simulink model "simulator_prototype_v2"  (R2021b)
(part 5 of 12)

tau_c = ft_4({t100,t1000,t1001,t1002,t1003,t1006,t1009,t101,t1011,t1014,t1015,t1017,t1018,t1019,t1020,t1021,t1023,t1024,t1025,t1028,t1029,t103,t1030,t1031,t1032,t1035,t1038,t1039,t104,t1041,t1042,t1044,t1045,t1046,t1048,t1049,t1050,t1051,t1052,t1055,t1056,t1057,t1058,t1059,t106,t1061,t1062,t1065,t1066,t1067,t107,t1070,t1071,t1072,t1073,t1074,t1075,t1076,t108,t1080,t1083,t1084,t1089,t109,t1090,t1091,t1092,t1094,t1095,t1098,t1099,t110,t1100,t1102,t1103,t1104,t1105,t1106,t1107,t1108,t1109,t111,t1110,t1111,t1112,t1113,t1114,t1115,t1116,t1117,t1118,t1119,t1120,t1121,t1122,t1123,t1124,t1125,t1126,t1129,t113,t1132,t1135,t1137,t1138,t1139,t114,t1140,t1141,t1142,t1144,t1145,t1146,t1147,t1148,t1149,t115,t1150,t1154,t1158,t1159,t1162,t1165,t1166,t1167,t1170,t1174,t1176,t1177,t1178,t1179,t118,t1180,t1184,t1185,t1186,t1187,t1188,t1189,t1190,t1192,t1193,t1194,t1195,t1196,t1197,t1198,t1199,t120,t1202,t1203,t1204,t1205,t1206,t1207,t1208,t1209,t121,t1210,t1212,t1213,t1214,t1217,t1218,t1219,t122,t1220,t1221,t1222,t1223,t1224,t1229,t123,t1230,t1232,t1234,t1235,t1236,t1237,t1238,t124,t1241,t1242,t1245,t1246,t1247,t1248,t125,t1251,t1252,t1253,t1254,t1255,t1256,t1259,t126,t1260,t1261,t1262,t1263,t1264,t1265,t1266,t1267,t1268,t127,t1270,t1271,t1272,t1277,t1278,t128,t1280,t1281,t1285,t1286,t1287,t1288,t1289,t1290,t1291,t1292,t1294,t1295,t1296,t1297,t1298,t1299,t130,t1300,t1301,t1302,t1303,t1304,t1305,t1307,t1310,t1311,t1316,t1317,t1319,t132,t1320,t1322,t1323,t1324,t1325,t1326,t1328,t133,t1330,t1331,t1332,t1334,t1335,t1336,t1337,t1338,t134,t1342,t1343,t1344,t1345,t1348,t1349,t1350,t1351,t1352,t1353,t1354,t136,t1360,t1364,t1366,t1367,t1368,t1369,t1370,t1371,t1372,t1374,t1375,t1376,t1377,t1378,t1379,t138,t1380,t1383,t1385,t1386,t1387,t1388,t1389,t139,t1392,t1393,t1394,t1395,t1396,t1397,t1398,t1399,t14,t140,t1401,t1402,t1403,t1404,t1405,t1406,t1407,t1408,t1409,t1410,t1411,t1412,t1413,t1414,t1415,t1416,t1417,t1418,t1419,t1420,t1421,t1422,t1423,t1424,t1425,t1426,t1427,t1428,t1429,t1430,t1431,t1432,t1433,t1434,t1435,t1436,t1437,t1439,t144,t1440,t1441,t1443,t1444,t1445,t1446,t1447,t1448,t145,t1451,t1453,t1454,t1456,t1457,t1458,t1459,t1460,t1461,t1462,t1463,t1464,t1468,t1469,t1471,t1474,t1477,t1478,t1479,t148,t1480,t1481,t1482,t1483,t1484,t1485,t1486,t1487,t1488,t1489,t149,t1490,t1491,t1492,t1493,t1494,t1495,t1497,t1498,t1499,t15,t150,t1500,t1501,t1503,t1504,t1505,t1506,t1507,t1509,t151,t1510,t1512,t1513,t1514,t1515,t1516,t1517,t1518,t1519,t152,t1520,t1522,t1523,t1525,t1526,t1527,t1528,t1529,t153,t1530,t1531,t1532,t1533,t1535,t1536,t1537,t1538,t1539,t1541,t1542,t1543,t1544,t1545,t1546,t1547,t1549,t1550,t1551,t1552,t1554,t1555,t1556,t1558,t1559,t156,t1560,t1565,t1567,t1568,t1569,t157,t1570,t1571,t1572,t1574,t1575,t1576,t1577,t1578,t1579,t158,t1581,t1582,t1583,t1584,t1585,t1586,t1587,t1588,t1591,t1592,t1593,t1594,t1595,t1596,t1599,t16,t160,t1600,t1601,t1602,t1604,t1605,t1606,t1607,t1608,t1609,t161,t1613,t1614,t1615,t1616,t1618,t1619,t162,t1620,t1621,t1622,t1623,t1624,t1625,t1626,t1627,t1628,t1629,t1631,t1633,t1634,t1635,t1636,t1637,t1638,t1639,t1640,t1641,t1642,t1643,t1644,t1645,t1646,t1648,t1649,t165,t1650,t1651,t1652,t1653,t1654,t1655,t1656,t1657,t1658,t166,t1660,t167,t168,t1686,t1688,t1689,t1690,t1695,t17,t170,t1700,t1701,t1702,t171,t172,t173,t174,t175,t1750,t176,t1765,t177,t178,t1780,t1782,t1795,t1796,t1797,t1798,t18,t180,t1807,t181,t1817,t182,t185,t186,t1865,t1868,t1870,t1871,t1872,t1873,t1874,t1875,t1876,t1877,t1879,t188,t1880,t1881,t1882,t1883,t1884,t1886,t1887,t1889,t189,t1890,t1891,t1894,t1895,t1897,t1898,t1899,t19,t190,t1901,t1902,t1903,t1904,t1907,t1909,t191,t1914,t1915,t1916,t1917,t1919,t192,t1920,t1922,t1923,t1924,t1925,t1926,t1927,t1928,t1929,t1930,t1931,t1936,t1937,t1940,t1941,t1942,t1943,t1947,t1948,t1949,t195,t1950,t1951,t1952,t1953,t1956,t1958,t1959,t196,t1960,t1961,t1965,t1966,t1967,t1968,t197,t1970,t1971,t1975,t1977,t198,t1982,t1991,t1997,t2,t20,t201,t2017,t202,t2021,t2022,t2024,t2025,t2027,t2028,t2029,t203,t2030,t2032,t2034,t2035,t2038,t2039,t204,t2043,t2044,t2045,t2049,t205,t2050,t2051,t2052,t2054,t2055,t2056,t2057,t2058,t2059,t2061,t2062,t2063,t2069,t207,t2075,t2077,t208,t2080,t2081,t2082,t2083,t2084,t2085,t2086,t2087,t2088,t2089,t209,t2090,t2091,t2092,t2093,t2096,t2097,t2098,t2099,t21,t210,t2100,t2101,t2102,t2103,t2104,t2105,t211,t2117,t2118,t2119,t212,t2120,t2121,t2122,t2123,t2124,t2131,t2138,t2139,t2140,t2147,t2149,t2150,t2151,t2152,t2153,t2154,t2155,t2156,t2157,t2158,t2159,t216,t217,t218,t219,t22,t221,t223,t225,t226,t227,t229,t2294,t2296,t2299,t23,t230,t2300,t2302,t2303,t2305,t2306,t2308,t2309,t231,t2310,t2313,t2314,t2315,t2316,t2317,t2318,t2319,t2322,t2323,t2324,t2325,t2326,t2327,t2328,t2329,t233,t2330,t2331,t2332,t2334,t2339,t2340,t2345,t2346,t2348,t2349,t2352,t2353,t2354,t2357,t2358,t2359,t236,t2360,t2361,t2362,t2364,t2365,t2366,t2367,t237,t2374,t2378,t238,t2382,t2383,t239,t2391,t2392,t2393,t24,t240,t2402,t2404,t2405,t2406,t2407,t2409,t241,t2411,t2415,t2416,t2417,t2418,t242,t2420,t2426,t2427,t2428,t2429,t243,t2430,t2431,t2432,t2433,t2434,t2435,t2436,t2437,t2438,t2439,t244,t2440,t2441,t2442,t2443,t2444,t2446,t2447,t2448,t2449,t245,t2451,t2452,t2453,t2454,t2455,t2456,t2457,t2459,t246,t2460,t2461,t2463,t2466,t2467,t2469,t247,t2471,t2475,t2482,t2483,t2484,t2485,t2486,t2487,t2488,t2491,t2495,t2498,t2499,t25,t2505,t251,t2512,t2513,t2515,t2529,t2541,t2544,t2546,t2551,t2560,t2567,t2568,t257,t2573,t2577,t2579,t2581,t2586,t2587,t2588,t259,t2593,t2594,t2595,t2596,t2597,t2599,t26,t260,t2600,t2601,t2603,t2605,t2606,t2607,t2608,t2609,t261,t2610,t2611,t2612,t2613,t2614,t2616,t2617,t2618,t2619,t262,t2620,t2621,t2622,t2623,t2624,t2625,t2626,t2627,t2628,t263,t2631,t2632,t2633,t2635,t2639,t264,t2640,t2641,t2642,t2643,t2645,t2646,t2647,t265,t2651,t2652,t2653,t2656,t266,t267,t268,t269,t27,t270,t271,t272,t2723,t2724,t2725,t2726,t2727,t2728,t2729,t273,t2730,t2735,t2736,t274,t2745,t2748,t2749,t275,t2750,t276,t2773,t2774,t2775,t2777,t2778,t2779,t2780,t2781,t2782,t2783,t2785,t2786,t2787,t2788,t279,t2797,t28,t280,t2800,t282,t283,t285,t2857,t2858,t2859,t286,t2860,t2865,t2867,t2868,t2872,t2879,t2883,t2884,t2886,t2887,t289,t2890,t2891,t2892,t2894,t2895,t2896,t2898,t2899,t2900,t2901,t2903,t2905,t2906,t2907,t2908,t291,t2915,t2917,t2918,t2919,t292,t293,t294,t295,t2959,t296,t2960,t2963,t2964,t2967,t2968,t297,t298,t299,t3,t30,t301,t303,t305,t306,t308,t309,t31,t310,t311,t312,t313,t314,t315,t316,t318,t319,t32,t320,t321,t322,t323,t325,t326,t328,t329,t33,t330,t331,t332,t333,t335,t336,t337,t338,t339,t34,t341,t343,t346,t348,t35,t350,t351,t352,t354,t355,t356,t358,t359,t36,t360,t361,t362,t363,t364,t365,t366,t368,t369,t370,t371,t372,t373,t377,t378,t38,t380,t381,t382,t385,t386,t387,t388,t389,t39,t390,t391,t392,t393,t396,t4,t403,t404,t406,t407,t408,t410,t411,t412,t413,t414,t415,t419,t42,t420,t421,t422,t424,t425,t426,t427,t428,t429,t43,t430,t431,t432,t433,t434,t435,t437,t438,t439,t440,t444,t445,t446,t448,t451,t452,t455,t456,t457,t458,t459,t46,t461,t463,t464,t465,t466,t467,t468,t469,t47,t471,t472,t473,t474,t476,t477,t478,t479,t480,t483,t485,t486,t488,t489,t49,t490,t491,t493,t494,t495,t496,t497,t498,t5,t50,t503,t504,t506,t507,t508,t509,t51,t510,t511,t512,t513,t514,t515,t516,t517,t518,t519,t52,t520,t521,t522,t523,t524,t525,t526,t527,t528,t53,t530,t531,t532,t533,t536,t537,t538,t539,t54,t540,t542,t543,t544,t545,t546,t547,t548,t550,t551,t552,t553,t554,t555,t556,t557,t559,t56,t560,t561,t562,t563,t565,t566,t568,t569,t570,t571,t572,t573,t574,t575,t576,t577,t578,t58,t580,t582,t583,t584,t585,t589,t59,t590,t591,t592,t595,t597,t599,t6,t60,t600,t601,t605,t606,t607,t608,t609,t610,t611,t612,t614,t615,t616,t618,t619,t620,t621,t622,t623,t624,t625,t627,t628,t629,t63,t631,t634,t635,t636,t638,t64,t640,t641,t642,t643,t645,t646,t648,t649,t65,t650,t651,t652,t654,t655,t656,t657,t658,t659,t660,t662,t663,t664,t665,t666,t667,t668,t669,t67,t670,t672,t673,t674,t675,t676,t677,t678,t679,t68,t681,t682,t683,t684,t685,t686,t687,t689,t69,t691,t692,t693,t694,t696,t698,t7,t70,t701,t702,t704,t705,t707,t708,t71,t710,t711,t712,t713,t714,t715,t716,t717,t718,t719,t720,t721,t722,t723,t724,t725,t726,t728,t73,t733,t735,t736,t738,t739,t740,t741,t742,t743,t744,t745,t746,t747,t749,t75,t750,t751,t755,t756,t757,t758,t759,t76,t762,t763,t764,t765,t766,t767,t768,t77,t770,t771,t772,t773,t774,t775,t776,t777,t778,t78,t781,t782,t783,t784,t785,t786,t787,t789,t79,t790,t791,t792,t793,t794,t796,t797,t798,t799,t80,t800,t801,t802,t806,t807,t808,t809,t81,t812,t813,t816,t817,t818,t819,t82,t820,t821,t822,t823,t824,t825,t826,t827,t828,t829,t830,t831,t832,t833,t836,t837,t838,t839,t84,t840,t841,t844,t845,t846,t85,t850,t851,t852,t853,t854,t855,t856,t857,t858,t859,t860,t861,t863,t864,t865,t866,t867,t868,t869,t870,t871,t872,t874,t875,t876,t877,t878,t881,t882,t883,t885,t887,t889,t89,t890,t891,t893,t894,t895,t896,t897,t898,t90,t900,t901,t902,t903,t904,t905,t906,t907,t908,t909,t91,t911,t912,t913,t914,t915,t916,t917,t918,t92,t920,t921,t923,t924,t926,t927,t929,t93,t930,t932,t933,t934,t935,t936,t937,t938,t939,t94,t940,t942,t943,t944,t945,t946,t947,t948,t950,t951,t952,t954,t956,t957,t959,t96,t960,t961,t962,t963,t964,t965,t966,t967,t969,t97,t970,t974,t975,t976,t977,t978,t981,t983,t985,t986,t987,t988,t989,t99,t990,t992,t993,t994,t995,t996,t997,t998,t999});
end
function tau_c = ft_4(ct)
t100 = ct{1};
t1000 = ct{2};
t1001 = ct{3};
t1002 = ct{4};
t1003 = ct{5};
t1006 = ct{6};
t1009 = ct{7};
t101 = ct{8};
t1011 = ct{9};
t1014 = ct{10};
t1015 = ct{11};
t1017 = ct{12};
t1018 = ct{13};
t1019 = ct{14};
t1020 = ct{15};
t1021 = ct{16};
t1023 = ct{17};
t1024 = ct{18};
t1025 = ct{19};
t1028 = ct{20};
t1029 = ct{21};
t103 = ct{22};
t1030 = ct{23};
t1031 = ct{24};
t1032 = ct{25};
t1035 = ct{26};
t1038 = ct{27};
t1039 = ct{28};
t104 = ct{29};
t1041 = ct{30};
t1042 = ct{31};
t1044 = ct{32};
t1045 = ct{33};
t1046 = ct{34};
t1048 = ct{35};
t1049 = ct{36};
t1050 = ct{37};
t1051 = ct{38};
t1052 = ct{39};
t1055 = ct{40};
t1056 = ct{41};
t1057 = ct{42};
t1058 = ct{43};
t1059 = ct{44};
t106 = ct{45};
t1061 = ct{46};
t1062 = ct{47};
t1065 = ct{48};
t1066 = ct{49};
t1067 = ct{50};
t107 = ct{51};
t1070 = ct{52};
t1071 = ct{53};
t1072 = ct{54};
t1073 = ct{55};
t1074 = ct{56};
t1075 = ct{57};
t1076 = ct{58};
t108 = ct{59};
t1080 = ct{60};
t1083 = ct{61};
t1084 = ct{62};
t1089 = ct{63};
t109 = ct{64};
t1090 = ct{65};
t1091 = ct{66};
t1092 = ct{67};
t1094 = ct{68};
t1095 = ct{69};
t1098 = ct{70};
t1099 = ct{71};
t110 = ct{72};
t1100 = ct{73};
t1102 = ct{74};
t1103 = ct{75};
t1104 = ct{76};
t1105 = ct{77};
t1106 = ct{78};
t1107 = ct{79};
t1108 = ct{80};
t1109 = ct{81};
t111 = ct{82};
t1110 = ct{83};
t1111 = ct{84};
t1112 = ct{85};
t1113 = ct{86};
t1114 = ct{87};
t1115 = ct{88};
t1116 = ct{89};
t1117 = ct{90};
t1118 = ct{91};
t1119 = ct{92};
t1120 = ct{93};
t1121 = ct{94};
t1122 = ct{95};
t1123 = ct{96};
t1124 = ct{97};
t1125 = ct{98};
t1126 = ct{99};
t1129 = ct{100};
t113 = ct{101};
t1132 = ct{102};
t1135 = ct{103};
t1137 = ct{104};
t1138 = ct{105};
t1139 = ct{106};
t114 = ct{107};
t1140 = ct{108};
t1141 = ct{109};
t1142 = ct{110};
t1144 = ct{111};
t1145 = ct{112};
t1146 = ct{113};
t1147 = ct{114};
t1148 = ct{115};
t1149 = ct{116};
t115 = ct{117};
t1150 = ct{118};
t1154 = ct{119};
t1158 = ct{120};
t1159 = ct{121};
t1162 = ct{122};
t1165 = ct{123};
t1166 = ct{124};
t1167 = ct{125};
t1170 = ct{126};
t1174 = ct{127};
t1176 = ct{128};
t1177 = ct{129};
t1178 = ct{130};
t1179 = ct{131};
t118 = ct{132};
t1180 = ct{133};
t1184 = ct{134};
t1185 = ct{135};
t1186 = ct{136};
t1187 = ct{137};
t1188 = ct{138};
t1189 = ct{139};
t1190 = ct{140};
t1192 = ct{141};
t1193 = ct{142};
t1194 = ct{143};
t1195 = ct{144};
t1196 = ct{145};
t1197 = ct{146};
t1198 = ct{147};
t1199 = ct{148};
t120 = ct{149};
t1202 = ct{150};
t1203 = ct{151};
t1204 = ct{152};
t1205 = ct{153};
t1206 = ct{154};
t1207 = ct{155};
t1208 = ct{156};
t1209 = ct{157};
t121 = ct{158};
t1210 = ct{159};
t1212 = ct{160};
t1213 = ct{161};
t1214 = ct{162};
t1217 = ct{163};
t1218 = ct{164};
t1219 = ct{165};
t122 = ct{166};
t1220 = ct{167};
t1221 = ct{168};
t1222 = ct{169};
t1223 = ct{170};
t1224 = ct{171};
t1229 = ct{172};
t123 = ct{173};
t1230 = ct{174};
t1232 = ct{175};
t1234 = ct{176};
t1235 = ct{177};
t1236 = ct{178};
t1237 = ct{179};
t1238 = ct{180};
t124 = ct{181};
t1241 = ct{182};
t1242 = ct{183};
t1245 = ct{184};
t1246 = ct{185};
t1247 = ct{186};
t1248 = ct{187};
t125 = ct{188};
t1251 = ct{189};
t1252 = ct{190};
t1253 = ct{191};
t1254 = ct{192};
t1255 = ct{193};
t1256 = ct{194};
t1259 = ct{195};
t126 = ct{196};
t1260 = ct{197};
t1261 = ct{198};
t1262 = ct{199};
t1263 = ct{200};
t1264 = ct{201};
t1265 = ct{202};
t1266 = ct{203};
t1267 = ct{204};
t1268 = ct{205};
t127 = ct{206};
t1270 = ct{207};
t1271 = ct{208};
t1272 = ct{209};
t1277 = ct{210};
t1278 = ct{211};
t128 = ct{212};
t1280 = ct{213};
t1281 = ct{214};
t1285 = ct{215};
t1286 = ct{216};
t1287 = ct{217};
t1288 = ct{218};
t1289 = ct{219};
t1290 = ct{220};
t1291 = ct{221};
t1292 = ct{222};
t1294 = ct{223};
t1295 = ct{224};
t1296 = ct{225};
t1297 = ct{226};
t1298 = ct{227};
t1299 = ct{228};
t130 = ct{229};
t1300 = ct{230};
t1301 = ct{231};
t1302 = ct{232};
t1303 = ct{233};
t1304 = ct{234};
t1305 = ct{235};
t1307 = ct{236};
t1310 = ct{237};
t1311 = ct{238};
t1316 = ct{239};
t1317 = ct{240};
t1319 = ct{241};
t132 = ct{242};
t1320 = ct{243};
t1322 = ct{244};
t1323 = ct{245};
t1324 = ct{246};
t1325 = ct{247};
t1326 = ct{248};
t1328 = ct{249};
t133 = ct{250};
t1330 = ct{251};
t1331 = ct{252};
t1332 = ct{253};
t1334 = ct{254};
t1335 = ct{255};
t1336 = ct{256};
t1337 = ct{257};
t1338 = ct{258};
t134 = ct{259};
t1342 = ct{260};
t1343 = ct{261};
t1344 = ct{262};
t1345 = ct{263};
t1348 = ct{264};
t1349 = ct{265};
t1350 = ct{266};
t1351 = ct{267};
t1352 = ct{268};
t1353 = ct{269};
t1354 = ct{270};
t136 = ct{271};
t1360 = ct{272};
t1364 = ct{273};
t1366 = ct{274};
t1367 = ct{275};
t1368 = ct{276};
t1369 = ct{277};
t1370 = ct{278};
t1371 = ct{279};
t1372 = ct{280};
t1374 = ct{281};
t1375 = ct{282};
t1376 = ct{283};
t1377 = ct{284};
t1378 = ct{285};
t1379 = ct{286};
t138 = ct{287};
t1380 = ct{288};
t1383 = ct{289};
t1385 = ct{290};
t1386 = ct{291};
t1387 = ct{292};
t1388 = ct{293};
t1389 = ct{294};
t139 = ct{295};
t1392 = ct{296};
t1393 = ct{297};
t1394 = ct{298};
t1395 = ct{299};
t1396 = ct{300};
t1397 = ct{301};
t1398 = ct{302};
t1399 = ct{303};
t14 = ct{304};
t140 = ct{305};
t1401 = ct{306};
t1402 = ct{307};
t1403 = ct{308};
t1404 = ct{309};
t1405 = ct{310};
t1406 = ct{311};
t1407 = ct{312};
t1408 = ct{313};
t1409 = ct{314};
t1410 = ct{315};
t1411 = ct{316};
t1412 = ct{317};
t1413 = ct{318};
t1414 = ct{319};
t1415 = ct{320};
t1416 = ct{321};
t1417 = ct{322};
t1418 = ct{323};
t1419 = ct{324};
t1420 = ct{325};
t1421 = ct{326};
t1422 = ct{327};
t1423 = ct{328};
t1424 = ct{329};
t1425 = ct{330};
t1426 = ct{331};
t1427 = ct{332};
t1428 = ct{333};
t1429 = ct{334};
t1430 = ct{335};
t1431 = ct{336};
t1432 = ct{337};
t1433 = ct{338};
t1434 = ct{339};
t1435 = ct{340};
t1436 = ct{341};
t1437 = ct{342};
t1439 = ct{343};
t144 = ct{344};
t1440 = ct{345};
t1441 = ct{346};
t1443 = ct{347};
t1444 = ct{348};
t1445 = ct{349};
t1446 = ct{350};
t1447 = ct{351};
t1448 = ct{352};
t145 = ct{353};
t1451 = ct{354};
t1453 = ct{355};
t1454 = ct{356};
t1456 = ct{357};
t1457 = ct{358};
t1458 = ct{359};
t1459 = ct{360};
t1460 = ct{361};
t1461 = ct{362};
t1462 = ct{363};
t1463 = ct{364};
t1464 = ct{365};
t1468 = ct{366};
t1469 = ct{367};
t1471 = ct{368};
t1474 = ct{369};
t1477 = ct{370};
t1478 = ct{371};
t1479 = ct{372};
t148 = ct{373};
t1480 = ct{374};
t1481 = ct{375};
t1482 = ct{376};
t1483 = ct{377};
t1484 = ct{378};
t1485 = ct{379};
t1486 = ct{380};
t1487 = ct{381};
t1488 = ct{382};
t1489 = ct{383};
t149 = ct{384};
t1490 = ct{385};
t1491 = ct{386};
t1492 = ct{387};
t1493 = ct{388};
t1494 = ct{389};
t1495 = ct{390};
t1497 = ct{391};
t1498 = ct{392};
t1499 = ct{393};
t15 = ct{394};
t150 = ct{395};
t1500 = ct{396};
t1501 = ct{397};
t1503 = ct{398};
t1504 = ct{399};
t1505 = ct{400};
t1506 = ct{401};
t1507 = ct{402};
t1509 = ct{403};
t151 = ct{404};
t1510 = ct{405};
t1512 = ct{406};
t1513 = ct{407};
t1514 = ct{408};
t1515 = ct{409};
t1516 = ct{410};
t1517 = ct{411};
t1518 = ct{412};
t1519 = ct{413};
t152 = ct{414};
t1520 = ct{415};
t1522 = ct{416};
t1523 = ct{417};
t1525 = ct{418};
t1526 = ct{419};
t1527 = ct{420};
t1528 = ct{421};
t1529 = ct{422};
t153 = ct{423};
t1530 = ct{424};
t1531 = ct{425};
t1532 = ct{426};
t1533 = ct{427};
t1535 = ct{428};
t1536 = ct{429};
t1537 = ct{430};
t1538 = ct{431};
t1539 = ct{432};
t1541 = ct{433};
t1542 = ct{434};
t1543 = ct{435};
t1544 = ct{436};
t1545 = ct{437};
t1546 = ct{438};
t1547 = ct{439};
t1549 = ct{440};
t1550 = ct{441};
t1551 = ct{442};
t1552 = ct{443};
t1554 = ct{444};
t1555 = ct{445};
t1556 = ct{446};
t1558 = ct{447};
t1559 = ct{448};
t156 = ct{449};
t1560 = ct{450};
t1565 = ct{451};
t1567 = ct{452};
t1568 = ct{453};
t1569 = ct{454};
t157 = ct{455};
t1570 = ct{456};
t1571 = ct{457};
t1572 = ct{458};
t1574 = ct{459};
t1575 = ct{460};
t1576 = ct{461};
t1577 = ct{462};
t1578 = ct{463};
t1579 = ct{464};
t158 = ct{465};
t1581 = ct{466};
t1582 = ct{467};
t1583 = ct{468};
t1584 = ct{469};
t1585 = ct{470};
t1586 = ct{471};
t1587 = ct{472};
t1588 = ct{473};
t1591 = ct{474};
t1592 = ct{475};
t1593 = ct{476};
t1594 = ct{477};
t1595 = ct{478};
t1596 = ct{479};
t1599 = ct{480};
t16 = ct{481};
t160 = ct{482};
t1600 = ct{483};
t1601 = ct{484};
t1602 = ct{485};
t1604 = ct{486};
t1605 = ct{487};
t1606 = ct{488};
t1607 = ct{489};
t1608 = ct{490};
t1609 = ct{491};
t161 = ct{492};
t1613 = ct{493};
t1614 = ct{494};
t1615 = ct{495};
t1616 = ct{496};
t1618 = ct{497};
t1619 = ct{498};
t162 = ct{499};
t1620 = ct{500};
t1621 = ct{501};
t1622 = ct{502};
t1623 = ct{503};
t1624 = ct{504};
t1625 = ct{505};
t1626 = ct{506};
t1627 = ct{507};
t1628 = ct{508};
t1629 = ct{509};
t1631 = ct{510};
t1633 = ct{511};
t1634 = ct{512};
t1635 = ct{513};
t1636 = ct{514};
t1637 = ct{515};
t1638 = ct{516};
t1639 = ct{517};
t1640 = ct{518};
t1641 = ct{519};
t1642 = ct{520};
t1643 = ct{521};
t1644 = ct{522};
t1645 = ct{523};
t1646 = ct{524};
t1648 = ct{525};
t1649 = ct{526};
t165 = ct{527};
t1650 = ct{528};
t1651 = ct{529};
t1652 = ct{530};
t1653 = ct{531};
t1654 = ct{532};
t1655 = ct{533};
t1656 = ct{534};
t1657 = ct{535};
t1658 = ct{536};
t166 = ct{537};
t1660 = ct{538};
t167 = ct{539};
t168 = ct{540};
t1686 = ct{541};
t1688 = ct{542};
t1689 = ct{543};
t1690 = ct{544};
t1695 = ct{545};
t17 = ct{546};
t170 = ct{547};
t1700 = ct{548};
t1701 = ct{549};
t1702 = ct{550};
t171 = ct{551};
t172 = ct{552};
t173 = ct{553};
t174 = ct{554};
t175 = ct{555};
t1750 = ct{556};
t176 = ct{557};
t1765 = ct{558};
t177 = ct{559};
t178 = ct{560};
t1780 = ct{561};
t1782 = ct{562};
t1795 = ct{563};
t1796 = ct{564};
t1797 = ct{565};
t1798 = ct{566};
t18 = ct{567};
t180 = ct{568};
t1807 = ct{569};
t181 = ct{570};
t1817 = ct{571};
t182 = ct{572};
t185 = ct{573};
t186 = ct{574};
t1865 = ct{575};
t1868 = ct{576};
t1870 = ct{577};
t1871 = ct{578};
t1872 = ct{579};
t1873 = ct{580};
t1874 = ct{581};
t1875 = ct{582};
t1876 = ct{583};
t1877 = ct{584};
t1879 = ct{585};
t188 = ct{586};
t1880 = ct{587};
t1881 = ct{588};
t1882 = ct{589};
t1883 = ct{590};
t1884 = ct{591};
t1886 = ct{592};
t1887 = ct{593};
t1889 = ct{594};
t189 = ct{595};
t1890 = ct{596};
t1891 = ct{597};
t1894 = ct{598};
t1895 = ct{599};
t1897 = ct{600};
t1898 = ct{601};
t1899 = ct{602};
t19 = ct{603};
t190 = ct{604};
t1901 = ct{605};
t1902 = ct{606};
t1903 = ct{607};
t1904 = ct{608};
t1907 = ct{609};
t1909 = ct{610};
t191 = ct{611};
t1914 = ct{612};
t1915 = ct{613};
t1916 = ct{614};
t1917 = ct{615};
t1919 = ct{616};
t192 = ct{617};
t1920 = ct{618};
t1922 = ct{619};
t1923 = ct{620};
t1924 = ct{621};
t1925 = ct{622};
t1926 = ct{623};
t1927 = ct{624};
t1928 = ct{625};
t1929 = ct{626};
t1930 = ct{627};
t1931 = ct{628};
t1936 = ct{629};
t1937 = ct{630};
t1940 = ct{631};
t1941 = ct{632};
t1942 = ct{633};
t1943 = ct{634};
t1947 = ct{635};
t1948 = ct{636};
t1949 = ct{637};
t195 = ct{638};
t1950 = ct{639};
t1951 = ct{640};
t1952 = ct{641};
t1953 = ct{642};
t1956 = ct{643};
t1958 = ct{644};
t1959 = ct{645};
t196 = ct{646};
t1960 = ct{647};
t1961 = ct{648};
t1965 = ct{649};
t1966 = ct{650};
t1967 = ct{651};
t1968 = ct{652};
t197 = ct{653};
t1970 = ct{654};
t1971 = ct{655};
t1975 = ct{656};
t1977 = ct{657};
t198 = ct{658};
t1982 = ct{659};
t1991 = ct{660};
t1997 = ct{661};
t2 = ct{662};
t20 = ct{663};
t201 = ct{664};
t2017 = ct{665};
t202 = ct{666};
t2021 = ct{667};
t2022 = ct{668};
t2024 = ct{669};
t2025 = ct{670};
t2027 = ct{671};
t2028 = ct{672};
t2029 = ct{673};
t203 = ct{674};
t2030 = ct{675};
t2032 = ct{676};
t2034 = ct{677};
t2035 = ct{678};
t2038 = ct{679};
t2039 = ct{680};
t204 = ct{681};
t2043 = ct{682};
t2044 = ct{683};
t2045 = ct{684};
t2049 = ct{685};
t205 = ct{686};
t2050 = ct{687};
t2051 = ct{688};
t2052 = ct{689};
t2054 = ct{690};
t2055 = ct{691};
t2056 = ct{692};
t2057 = ct{693};
t2058 = ct{694};
t2059 = ct{695};
t2061 = ct{696};
t2062 = ct{697};
t2063 = ct{698};
t2069 = ct{699};
t207 = ct{700};
t2075 = ct{701};
t2077 = ct{702};
t208 = ct{703};
t2080 = ct{704};
t2081 = ct{705};
t2082 = ct{706};
t2083 = ct{707};
t2084 = ct{708};
t2085 = ct{709};
t2086 = ct{710};
t2087 = ct{711};
t2088 = ct{712};
t2089 = ct{713};
t209 = ct{714};
t2090 = ct{715};
t2091 = ct{716};
t2092 = ct{717};
t2093 = ct{718};
t2096 = ct{719};
t2097 = ct{720};
t2098 = ct{721};
t2099 = ct{722};
t21 = ct{723};
t210 = ct{724};
t2100 = ct{725};
t2101 = ct{726};
t2102 = ct{727};
t2103 = ct{728};
t2104 = ct{729};
t2105 = ct{730};
t211 = ct{731};
t2117 = ct{732};
t2118 = ct{733};
t2119 = ct{734};
t212 = ct{735};
t2120 = ct{736};
t2121 = ct{737};
t2122 = ct{738};
t2123 = ct{739};
t2124 = ct{740};
t2131 = ct{741};
t2138 = ct{742};
t2139 = ct{743};
t2140 = ct{744};
t2147 = ct{745};
t2149 = ct{746};
t2150 = ct{747};
t2151 = ct{748};
t2152 = ct{749};
t2153 = ct{750};
t2154 = ct{751};
t2155 = ct{752};
t2156 = ct{753};
t2157 = ct{754};
t2158 = ct{755};
t2159 = ct{756};
t216 = ct{757};
t217 = ct{758};
t218 = ct{759};
t219 = ct{760};
t22 = ct{761};
t221 = ct{762};
t223 = ct{763};
t225 = ct{764};
t226 = ct{765};
t227 = ct{766};
t229 = ct{767};
t2294 = ct{768};
t2296 = ct{769};
t2299 = ct{770};
t23 = ct{771};
t230 = ct{772};
t2300 = ct{773};
t2302 = ct{774};
t2303 = ct{775};
t2305 = ct{776};
t2306 = ct{777};
t2308 = ct{778};
t2309 = ct{779};
t231 = ct{780};
t2310 = ct{781};
t2313 = ct{782};
t2314 = ct{783};
t2315 = ct{784};
t2316 = ct{785};
t2317 = ct{786};
t2318 = ct{787};
t2319 = ct{788};
t2322 = ct{789};
t2323 = ct{790};
t2324 = ct{791};
t2325 = ct{792};
t2326 = ct{793};
t2327 = ct{794};
t2328 = ct{795};
t2329 = ct{796};
t233 = ct{797};
t2330 = ct{798};
t2331 = ct{799};
t2332 = ct{800};
t2334 = ct{801};
t2339 = ct{802};
t2340 = ct{803};
t2345 = ct{804};
t2346 = ct{805};
t2348 = ct{806};
t2349 = ct{807};
t2352 = ct{808};
t2353 = ct{809};
t2354 = ct{810};
t2357 = ct{811};
t2358 = ct{812};
t2359 = ct{813};
t236 = ct{814};
t2360 = ct{815};
t2361 = ct{816};
t2362 = ct{817};
t2364 = ct{818};
t2365 = ct{819};
t2366 = ct{820};
t2367 = ct{821};
t237 = ct{822};
t2374 = ct{823};
t2378 = ct{824};
t238 = ct{825};
t2382 = ct{826};
t2383 = ct{827};
t239 = ct{828};
t2391 = ct{829};
t2392 = ct{830};
t2393 = ct{831};
t24 = ct{832};
t240 = ct{833};
t2402 = ct{834};
t2404 = ct{835};
t2405 = ct{836};
t2406 = ct{837};
t2407 = ct{838};
t2409 = ct{839};
t241 = ct{840};
t2411 = ct{841};
t2415 = ct{842};
t2416 = ct{843};
t2417 = ct{844};
t2418 = ct{845};
t242 = ct{846};
t2420 = ct{847};
t2426 = ct{848};
t2427 = ct{849};
t2428 = ct{850};
t2429 = ct{851};
t243 = ct{852};
t2430 = ct{853};
t2431 = ct{854};
t2432 = ct{855};
t2433 = ct{856};
t2434 = ct{857};
t2435 = ct{858};
t2436 = ct{859};
t2437 = ct{860};
t2438 = ct{861};
t2439 = ct{862};
t244 = ct{863};
t2440 = ct{864};
t2441 = ct{865};
t2442 = ct{866};
t2443 = ct{867};
t2444 = ct{868};
t2446 = ct{869};
t2447 = ct{870};
t2448 = ct{871};
t2449 = ct{872};
t245 = ct{873};
t2451 = ct{874};
t2452 = ct{875};
t2453 = ct{876};
t2454 = ct{877};
t2455 = ct{878};
t2456 = ct{879};
t2457 = ct{880};
t2459 = ct{881};
t246 = ct{882};
t2460 = ct{883};
t2461 = ct{884};
t2463 = ct{885};
t2466 = ct{886};
t2467 = ct{887};
t2469 = ct{888};
t247 = ct{889};
t2471 = ct{890};
t2475 = ct{891};
t2482 = ct{892};
t2483 = ct{893};
t2484 = ct{894};
t2485 = ct{895};
t2486 = ct{896};
t2487 = ct{897};
t2488 = ct{898};
t2491 = ct{899};
t2495 = ct{900};
t2498 = ct{901};
t2499 = ct{902};
t25 = ct{903};
t2505 = ct{904};
t251 = ct{905};
t2512 = ct{906};
t2513 = ct{907};
t2515 = ct{908};
t2529 = ct{909};
t2541 = ct{910};
t2544 = ct{911};
t2546 = ct{912};
t2551 = ct{913};
t2560 = ct{914};
t2567 = ct{915};
t2568 = ct{916};
t257 = ct{917};
t2573 = ct{918};
t2577 = ct{919};
t2579 = ct{920};
t2581 = ct{921};
t2586 = ct{922};
t2587 = ct{923};
t2588 = ct{924};
t259 = ct{925};
t2593 = ct{926};
t2594 = ct{927};
t2595 = ct{928};
t2596 = ct{929};
t2597 = ct{930};
t2599 = ct{931};
t26 = ct{932};
t260 = ct{933};
t2600 = ct{934};
t2601 = ct{935};
t2603 = ct{936};
t2605 = ct{937};
t2606 = ct{938};
t2607 = ct{939};
t2608 = ct{940};
t2609 = ct{941};
t261 = ct{942};
t2610 = ct{943};
t2611 = ct{944};
t2612 = ct{945};
t2613 = ct{946};
t2614 = ct{947};
t2616 = ct{948};
t2617 = ct{949};
t2618 = ct{950};
t2619 = ct{951};
t262 = ct{952};
t2620 = ct{953};
t2621 = ct{954};
t2622 = ct{955};
t2623 = ct{956};
t2624 = ct{957};
t2625 = ct{958};
t2626 = ct{959};
t2627 = ct{960};
t2628 = ct{961};
t263 = ct{962};
t2631 = ct{963};
t2632 = ct{964};
t2633 = ct{965};
t2635 = ct{966};
t2639 = ct{967};
t264 = ct{968};
t2640 = ct{969};
t2641 = ct{970};
t2642 = ct{971};
t2643 = ct{972};
t2645 = ct{973};
t2646 = ct{974};
t2647 = ct{975};
t265 = ct{976};
t2651 = ct{977};
t2652 = ct{978};
t2653 = ct{979};
t2656 = ct{980};
t266 = ct{981};
t267 = ct{982};
t268 = ct{983};
t269 = ct{984};
t27 = ct{985};
t270 = ct{986};
t271 = ct{987};
t272 = ct{988};
t2723 = ct{989};
t2724 = ct{990};
t2725 = ct{991};
t2726 = ct{992};
t2727 = ct{993};
t2728 = ct{994};
t2729 = ct{995};
t273 = ct{996};
t2730 = ct{997};
t2735 = ct{998};
t2736 = ct{999};
t274 = ct{1000};
t2745 = ct{1001};
t2748 = ct{1002};
t2749 = ct{1003};
t275 = ct{1004};
t2750 = ct{1005};
t276 = ct{1006};
t2773 = ct{1007};
t2774 = ct{1008};
t2775 = ct{1009};
t2777 = ct{1010};
t2778 = ct{1011};
t2779 = ct{1012};
t2780 = ct{1013};
t2781 = ct{1014};
t2782 = ct{1015};
t2783 = ct{1016};
t2785 = ct{1017};
t2786 = ct{1018};
t2787 = ct{1019};
t2788 = ct{1020};
t279 = ct{1021};
t2797 = ct{1022};
t28 = ct{1023};
t280 = ct{1024};
t2800 = ct{1025};
t282 = ct{1026};
t283 = ct{1027};
t285 = ct{1028};
t2857 = ct{1029};
t2858 = ct{1030};
t2859 = ct{1031};
t286 = ct{1032};
t2860 = ct{1033};
t2865 = ct{1034};
t2867 = ct{1035};
t2868 = ct{1036};
t2872 = ct{1037};
t2879 = ct{1038};
t2883 = ct{1039};
t2884 = ct{1040};
t2886 = ct{1041};
t2887 = ct{1042};
t289 = ct{1043};
t2890 = ct{1044};
t2891 = ct{1045};
t2892 = ct{1046};
t2894 = ct{1047};
t2895 = ct{1048};
t2896 = ct{1049};
t2898 = ct{1050};
t2899 = ct{1051};
t2900 = ct{1052};
t2901 = ct{1053};
t2903 = ct{1054};
t2905 = ct{1055};
t2906 = ct{1056};
t2907 = ct{1057};
t2908 = ct{1058};
t291 = ct{1059};
t2915 = ct{1060};
t2917 = ct{1061};
t2918 = ct{1062};
t2919 = ct{1063};
t292 = ct{1064};
t293 = ct{1065};
t294 = ct{1066};
t295 = ct{1067};
t2959 = ct{1068};
t296 = ct{1069};
t2960 = ct{1070};
t2963 = ct{1071};
t2964 = ct{1072};
t2967 = ct{1073};
t2968 = ct{1074};
t297 = ct{1075};
t298 = ct{1076};
t299 = ct{1077};
t3 = ct{1078};
t30 = ct{1079};
t301 = ct{1080};
t303 = ct{1081};
t305 = ct{1082};
t306 = ct{1083};
t308 = ct{1084};
t309 = ct{1085};
t31 = ct{1086};
t310 = ct{1087};
t311 = ct{1088};
t312 = ct{1089};
t313 = ct{1090};
t314 = ct{1091};
t315 = ct{1092};
t316 = ct{1093};
t318 = ct{1094};
t319 = ct{1095};
t32 = ct{1096};
t320 = ct{1097};
t321 = ct{1098};
t322 = ct{1099};
t323 = ct{1100};
t325 = ct{1101};
t326 = ct{1102};
t328 = ct{1103};
t329 = ct{1104};
t33 = ct{1105};
t330 = ct{1106};
t331 = ct{1107};
t332 = ct{1108};
t333 = ct{1109};
t335 = ct{1110};
t336 = ct{1111};
t337 = ct{1112};
t338 = ct{1113};
t339 = ct{1114};
t34 = ct{1115};
t341 = ct{1116};
t343 = ct{1117};
t346 = ct{1118};
t348 = ct{1119};
t35 = ct{1120};
t350 = ct{1121};
t351 = ct{1122};
t352 = ct{1123};
t354 = ct{1124};
t355 = ct{1125};
t356 = ct{1126};
t358 = ct{1127};
t359 = ct{1128};
t36 = ct{1129};
t360 = ct{1130};
t361 = ct{1131};
t362 = ct{1132};
t363 = ct{1133};
t364 = ct{1134};
t365 = ct{1135};
t366 = ct{1136};
t368 = ct{1137};
t369 = ct{1138};
t370 = ct{1139};
t371 = ct{1140};
t372 = ct{1141};
t373 = ct{1142};
t377 = ct{1143};
t378 = ct{1144};
t38 = ct{1145};
t380 = ct{1146};
t381 = ct{1147};
t382 = ct{1148};
t385 = ct{1149};
t386 = ct{1150};
t387 = ct{1151};
t388 = ct{1152};
t389 = ct{1153};
t39 = ct{1154};
t390 = ct{1155};
t391 = ct{1156};
t392 = ct{1157};
t393 = ct{1158};
t396 = ct{1159};
t4 = ct{1160};
t403 = ct{1161};
t404 = ct{1162};
t406 = ct{1163};
t407 = ct{1164};
t408 = ct{1165};
t410 = ct{1166};
t411 = ct{1167};
t412 = ct{1168};
t413 = ct{1169};
t414 = ct{1170};
t415 = ct{1171};
t419 = ct{1172};
t42 = ct{1173};
t420 = ct{1174};
t421 = ct{1175};
t422 = ct{1176};
t424 = ct{1177};
t425 = ct{1178};
t426 = ct{1179};
t427 = ct{1180};
t428 = ct{1181};
t429 = ct{1182};
t43 = ct{1183};
t430 = ct{1184};
t431 = ct{1185};
t432 = ct{1186};
t433 = ct{1187};
t434 = ct{1188};
t435 = ct{1189};
t437 = ct{1190};
t438 = ct{1191};
t439 = ct{1192};
t440 = ct{1193};
t444 = ct{1194};
t445 = ct{1195};
t446 = ct{1196};
t448 = ct{1197};
t451 = ct{1198};
t452 = ct{1199};
t455 = ct{1200};
t456 = ct{1201};
t457 = ct{1202};
t458 = ct{1203};
t459 = ct{1204};
t46 = ct{1205};
t461 = ct{1206};
t463 = ct{1207};
t464 = ct{1208};
t465 = ct{1209};
t466 = ct{1210};
t467 = ct{1211};
t468 = ct{1212};
t469 = ct{1213};
t47 = ct{1214};
t471 = ct{1215};
t472 = ct{1216};
t473 = ct{1217};
t474 = ct{1218};
t476 = ct{1219};
t477 = ct{1220};
t478 = ct{1221};
t479 = ct{1222};
t480 = ct{1223};
t483 = ct{1224};
t485 = ct{1225};
t486 = ct{1226};
t488 = ct{1227};
t489 = ct{1228};
t49 = ct{1229};
t490 = ct{1230};
t491 = ct{1231};
t493 = ct{1232};
t494 = ct{1233};
t495 = ct{1234};
t496 = ct{1235};
t497 = ct{1236};
t498 = ct{1237};
t5 = ct{1238};
t50 = ct{1239};
t503 = ct{1240};
t504 = ct{1241};
t506 = ct{1242};
t507 = ct{1243};
t508 = ct{1244};
t509 = ct{1245};
t51 = ct{1246};
t510 = ct{1247};
t511 = ct{1248};
t512 = ct{1249};
t513 = ct{1250};
t514 = ct{1251};
t515 = ct{1252};
t516 = ct{1253};
t517 = ct{1254};
t518 = ct{1255};
t519 = ct{1256};
t52 = ct{1257};
t520 = ct{1258};
t521 = ct{1259};
t522 = ct{1260};
t523 = ct{1261};
t524 = ct{1262};
t525 = ct{1263};
t526 = ct{1264};
t527 = ct{1265};
t528 = ct{1266};
t53 = ct{1267};
t530 = ct{1268};
t531 = ct{1269};
t532 = ct{1270};
t533 = ct{1271};
t536 = ct{1272};
t537 = ct{1273};
t538 = ct{1274};
t539 = ct{1275};
t54 = ct{1276};
t540 = ct{1277};
t542 = ct{1278};
t543 = ct{1279};
t544 = ct{1280};
t545 = ct{1281};
t546 = ct{1282};
t547 = ct{1283};
t548 = ct{1284};
t550 = ct{1285};
t551 = ct{1286};
t552 = ct{1287};
t553 = ct{1288};
t554 = ct{1289};
t555 = ct{1290};
t556 = ct{1291};
t557 = ct{1292};
t559 = ct{1293};
t56 = ct{1294};
t560 = ct{1295};
t561 = ct{1296};
t562 = ct{1297};
t563 = ct{1298};
t565 = ct{1299};
t566 = ct{1300};
t568 = ct{1301};
t569 = ct{1302};
t570 = ct{1303};
t571 = ct{1304};
t572 = ct{1305};
t573 = ct{1306};
t574 = ct{1307};
t575 = ct{1308};
t576 = ct{1309};
t577 = ct{1310};
t578 = ct{1311};
t58 = ct{1312};
t580 = ct{1313};
t582 = ct{1314};
t583 = ct{1315};
t584 = ct{1316};
t585 = ct{1317};
t589 = ct{1318};
t59 = ct{1319};
t590 = ct{1320};
t591 = ct{1321};
t592 = ct{1322};
t595 = ct{1323};
t597 = ct{1324};
t599 = ct{1325};
t6 = ct{1326};
t60 = ct{1327};
t600 = ct{1328};
t601 = ct{1329};
t605 = ct{1330};
t606 = ct{1331};
t607 = ct{1332};
t608 = ct{1333};
t609 = ct{1334};
t610 = ct{1335};
t611 = ct{1336};
t612 = ct{1337};
t614 = ct{1338};
t615 = ct{1339};
t616 = ct{1340};
t618 = ct{1341};
t619 = ct{1342};
t620 = ct{1343};
t621 = ct{1344};
t622 = ct{1345};
t623 = ct{1346};
t624 = ct{1347};
t625 = ct{1348};
t627 = ct{1349};
t628 = ct{1350};
t629 = ct{1351};
t63 = ct{1352};
t631 = ct{1353};
t634 = ct{1354};
t635 = ct{1355};
t636 = ct{1356};
t638 = ct{1357};
t64 = ct{1358};
t640 = ct{1359};
t641 = ct{1360};
t642 = ct{1361};
t643 = ct{1362};
t645 = ct{1363};
t646 = ct{1364};
t648 = ct{1365};
t649 = ct{1366};
t65 = ct{1367};
t650 = ct{1368};
t651 = ct{1369};
t652 = ct{1370};
t654 = ct{1371};
t655 = ct{1372};
t656 = ct{1373};
t657 = ct{1374};
t658 = ct{1375};
t659 = ct{1376};
t660 = ct{1377};
t662 = ct{1378};
t663 = ct{1379};
t664 = ct{1380};
t665 = ct{1381};
t666 = ct{1382};
t667 = ct{1383};
t668 = ct{1384};
t669 = ct{1385};
t67 = ct{1386};
t670 = ct{1387};
t672 = ct{1388};
t673 = ct{1389};
t674 = ct{1390};
t675 = ct{1391};
t676 = ct{1392};
t677 = ct{1393};
t678 = ct{1394};
t679 = ct{1395};
t68 = ct{1396};
t681 = ct{1397};
t682 = ct{1398};
t683 = ct{1399};
t684 = ct{1400};
t685 = ct{1401};
t686 = ct{1402};
t687 = ct{1403};
t689 = ct{1404};
t69 = ct{1405};
t691 = ct{1406};
t692 = ct{1407};
t693 = ct{1408};
t694 = ct{1409};
t696 = ct{1410};
t698 = ct{1411};
t7 = ct{1412};
t70 = ct{1413};
t701 = ct{1414};
t702 = ct{1415};
t704 = ct{1416};
t705 = ct{1417};
t707 = ct{1418};
t708 = ct{1419};
t71 = ct{1420};
t710 = ct{1421};
t711 = ct{1422};
t712 = ct{1423};
t713 = ct{1424};
t714 = ct{1425};
t715 = ct{1426};
t716 = ct{1427};
t717 = ct{1428};
t718 = ct{1429};
t719 = ct{1430};
t720 = ct{1431};
t721 = ct{1432};
t722 = ct{1433};
t723 = ct{1434};
t724 = ct{1435};
t725 = ct{1436};
t726 = ct{1437};
t728 = ct{1438};
t73 = ct{1439};
t733 = ct{1440};
t735 = ct{1441};
t736 = ct{1442};
t738 = ct{1443};
t739 = ct{1444};
t740 = ct{1445};
t741 = ct{1446};
t742 = ct{1447};
t743 = ct{1448};
t744 = ct{1449};
t745 = ct{1450};
t746 = ct{1451};
t747 = ct{1452};
t749 = ct{1453};
t75 = ct{1454};
t750 = ct{1455};
t751 = ct{1456};
t755 = ct{1457};
t756 = ct{1458};
t757 = ct{1459};
t758 = ct{1460};
t759 = ct{1461};
t76 = ct{1462};
t762 = ct{1463};
t763 = ct{1464};
t764 = ct{1465};
t765 = ct{1466};
t766 = ct{1467};
t767 = ct{1468};
t768 = ct{1469};
t77 = ct{1470};
t770 = ct{1471};
t771 = ct{1472};
t772 = ct{1473};
t773 = ct{1474};
t774 = ct{1475};
t775 = ct{1476};
t776 = ct{1477};
t777 = ct{1478};
t778 = ct{1479};
t78 = ct{1480};
t781 = ct{1481};
t782 = ct{1482};
t783 = ct{1483};
t784 = ct{1484};
t785 = ct{1485};
t786 = ct{1486};
t787 = ct{1487};
t789 = ct{1488};
t79 = ct{1489};
t790 = ct{1490};
t791 = ct{1491};
t792 = ct{1492};
t793 = ct{1493};
t794 = ct{1494};
t796 = ct{1495};
t797 = ct{1496};
t798 = ct{1497};
t799 = ct{1498};
t80 = ct{1499};
t800 = ct{1500};
t801 = ct{1501};
t802 = ct{1502};
t806 = ct{1503};
t807 = ct{1504};
t808 = ct{1505};
t809 = ct{1506};
t81 = ct{1507};
t812 = ct{1508};
t813 = ct{1509};
t816 = ct{1510};
t817 = ct{1511};
t818 = ct{1512};
t819 = ct{1513};
t82 = ct{1514};
t820 = ct{1515};
t821 = ct{1516};
t822 = ct{1517};
t823 = ct{1518};
t824 = ct{1519};
t825 = ct{1520};
t826 = ct{1521};
t827 = ct{1522};
t828 = ct{1523};
t829 = ct{1524};
t830 = ct{1525};
t831 = ct{1526};
t832 = ct{1527};
t833 = ct{1528};
t836 = ct{1529};
t837 = ct{1530};
t838 = ct{1531};
t839 = ct{1532};
t84 = ct{1533};
t840 = ct{1534};
t841 = ct{1535};
t844 = ct{1536};
t845 = ct{1537};
t846 = ct{1538};
t85 = ct{1539};
t850 = ct{1540};
t851 = ct{1541};
t852 = ct{1542};
t853 = ct{1543};
t854 = ct{1544};
t855 = ct{1545};
t856 = ct{1546};
t857 = ct{1547};
t858 = ct{1548};
t859 = ct{1549};
t860 = ct{1550};
t861 = ct{1551};
t863 = ct{1552};
t864 = ct{1553};
t865 = ct{1554};
t866 = ct{1555};
t867 = ct{1556};
t868 = ct{1557};
t869 = ct{1558};
t870 = ct{1559};
t871 = ct{1560};
t872 = ct{1561};
t874 = ct{1562};
t875 = ct{1563};
t876 = ct{1564};
t877 = ct{1565};
t878 = ct{1566};
t881 = ct{1567};
t882 = ct{1568};
t883 = ct{1569};
t885 = ct{1570};
t887 = ct{1571};
t889 = ct{1572};
t89 = ct{1573};
t890 = ct{1574};
t891 = ct{1575};
t893 = ct{1576};
t894 = ct{1577};
t895 = ct{1578};
t896 = ct{1579};
t897 = ct{1580};
t898 = ct{1581};
t90 = ct{1582};
t900 = ct{1583};
t901 = ct{1584};
t902 = ct{1585};
t903 = ct{1586};
t904 = ct{1587};
t905 = ct{1588};
t906 = ct{1589};
t907 = ct{1590};
t908 = ct{1591};
t909 = ct{1592};
t91 = ct{1593};
t911 = ct{1594};
t912 = ct{1595};
t913 = ct{1596};
t914 = ct{1597};
t915 = ct{1598};
t916 = ct{1599};
t917 = ct{1600};
t918 = ct{1601};
t92 = ct{1602};
t920 = ct{1603};
t921 = ct{1604};
t923 = ct{1605};
t924 = ct{1606};
t926 = ct{1607};
t927 = ct{1608};
t929 = ct{1609};
t93 = ct{1610};
t930 = ct{1611};
t932 = ct{1612};
t933 = ct{1613};
t934 = ct{1614};
t935 = ct{1615};
t936 = ct{1616};
t937 = ct{1617};
t938 = ct{1618};
t939 = ct{1619};
t94 = ct{1620};
t940 = ct{1621};
t942 = ct{1622};
t943 = ct{1623};
t944 = ct{1624};
t945 = ct{1625};
t946 = ct{1626};
t947 = ct{1627};
t948 = ct{1628};
t950 = ct{1629};
t951 = ct{1630};
t952 = ct{1631};
t954 = ct{1632};
t956 = ct{1633};
t957 = ct{1634};
t959 = ct{1635};
t96 = ct{1636};
t960 = ct{1637};
t961 = ct{1638};
t962 = ct{1639};
t963 = ct{1640};
t964 = ct{1641};
t965 = ct{1642};
t966 = ct{1643};
t967 = ct{1644};
t969 = ct{1645};
t97 = ct{1646};
t970 = ct{1647};
t974 = ct{1648};
t975 = ct{1649};
t976 = ct{1650};
t977 = ct{1651};
t978 = ct{1652};
t981 = ct{1653};
t983 = ct{1654};
t985 = ct{1655};
t986 = ct{1656};
t987 = ct{1657};
t988 = ct{1658};
t989 = ct{1659};
t99 = ct{1660};
t990 = ct{1661};
t992 = ct{1662};
t993 = ct{1663};
t994 = ct{1664};
t995 = ct{1665};
t996 = ct{1666};
t997 = ct{1667};
t998 = ct{1668};
t999 = ct{1669};
t1659 = t17.*t19.*t20.*t237.*3.257046415933332e-3;
t1661 = t14.*t15.*t22.*t237.*1.485161268617439e-3;
t1662 = t14.*t17.*t20.*t237.*1.485161268617439e-3;
t1663 = t15.*t17.*t19.*t237.*1.485161268617439e-3;
t1664 = t14.*t15.*t22.*t237.*5.478347731418506e-3;
t1665 = t14.*t15.*t17.*t238.*5.478347731418506e-3;
t1666 = t14.*t17.*t20.*t237.*5.478347731418506e-3;
t1667 = t15.*t17.*t19.*t237.*5.478347731418506e-3;
t1668 = t19.*t20.*t22.*t238.*2.498039274760989e-3;
t1669 = -t1623;
t1670 = t19.*t20.*t22.*t237.*3.257046415933332e-3;
t1671 = t17.*t19.*t20.*t238.*3.257046415933332e-3;
t1672 = t14.*t15.*t22.*t238.*1.485161268617439e-3;
t1673 = t14.*t20.*t22.*t237.*1.485161268617439e-3;
t1674 = t15.*t19.*t22.*t237.*1.485161268617439e-3;
t1675 = t17.*t19.*t20.*t237.*1.485161268617439e-3;
t1676 = t14.*t20.*t22.*t237.*5.478347731418506e-3;
t1677 = t14.*t17.*t20.*t238.*5.478347731418506e-3;
t1678 = t15.*t19.*t22.*t237.*5.478347731418506e-3;
t1679 = t15.*t17.*t19.*t238.*5.478347731418506e-3;
t1680 = t17.*t19.*t20.*t237.*5.478347731418506e-3;
t1681 = t14.*t20.*t22.*t238.*1.485161268617439e-3;
t1682 = t15.*t19.*t22.*t238.*1.485161268617439e-3;
t1683 = t19.*t20.*t22.*t237.*1.485161268617439e-3;
t1684 = t19.*t20.*t22.*t237.*5.478347731418506e-3;
t1685 = t17.*t19.*t20.*t238.*5.478347731418506e-3;
t1687 = t19.*t20.*t22.*t238.*1.485161268617439e-3;
t1691 = t14.*t15.*t237.*1.509490621508912e-3;
t1692 = t14.*t15.*t238.*1.509490621508912e-3;
t1693 = t14.*t20.*t237.*1.509490621508912e-3;
t1694 = t15.*t19.*t237.*1.509490621508912e-3;
t1696 = t14.*t20.*t238.*1.509490621508912e-3;
t1697 = t15.*t19.*t238.*1.509490621508912e-3;
t1698 = t19.*t20.*t237.*1.509490621508912e-3;
t1699 = t264.*3.212809800067317e-5;
t1704 = t262.*(t46-t47).*(-7.183142969324763e-22);
t1705 = t14.*t15.*t237.*1.689683482265228e-6;
t1706 = t14.*t15.*t238.*1.689683482265228e-6;
t1707 = t14.*t20.*t237.*1.689683482265228e-6;
t1708 = t15.*t19.*t237.*1.689683482265228e-6;
t1710 = t14.*t20.*t238.*1.689683482265228e-6;
t1711 = t15.*t19.*t238.*1.689683482265228e-6;
t1712 = t19.*t20.*t237.*1.689683482265228e-6;
t1716 = t19.*t20.*t238.*1.689683482265228e-6;
t1717 = -t1638;
t1738 = -t1686;
t1739 = t33.*t262.*3.161027044821787e-5;
t1740 = t27.*t264.*3.161027044821787e-5;
t1741 = -t1688;
t1742 = -t1689;
t1743 = t33.*t264.*3.161027044821787e-5;
t1745 = t27.*t262.*6.932319085178867e-5;
t1749 = t27.*t264.*6.932319085178867e-5;
t1751 = t33.*t264.*6.932319085178867e-5;
t1752 = -t1700;
t1753 = -t1701;
t1754 = -t1702;
t1756 = t14.*t15.*t237.*2.842045365580232e-6;
t1757 = t14.*t15.*t238.*2.842045365580232e-6;
t1758 = t14.*t20.*t237.*2.842045365580232e-6;
t1759 = t15.*t19.*t237.*2.842045365580232e-6;
t1760 = t14.*t20.*t238.*2.842045365580232e-6;
t1761 = t15.*t19.*t238.*2.842045365580232e-6;
t1762 = t19.*t20.*t237.*2.842045365580232e-6;
t1764 = t19.*t20.*t238.*2.842045365580232e-6;
t1766 = t262.*9.554306323645785e-8;
t1768 = t262.*3.596333474007969e-8;
t1769 = t264.*9.554306323645785e-8;
t1770 = t14.*t15.*t237.*2.538961213904336e-3;
t1771 = t14.*t15.*t238.*2.538961213904336e-3;
t1772 = t14.*t20.*t237.*2.538961213904336e-3;
t1773 = t15.*t19.*t237.*2.538961213904336e-3;
t1775 = t14.*t20.*t238.*2.538961213904336e-3;
t1776 = t15.*t19.*t238.*2.538961213904336e-3;
t1777 = t19.*t20.*t237.*2.538961213904336e-3;
t1779 = t19.*t20.*t238.*2.538961213904336e-3;
t1786 = t26.*t50.*t240.*1.553819674864718e+37i;
t1793 = -t1780;
t1794 = -t1782;
t1799 = t26.*t28.*t50.*t240.*2.657049668350291e+37i;
t1800 = -t1798;
t1801 = t26.*t34.*t50.*t240.*4.888570919953966e+37i;
t1802 = t32.*t50.*t240.*1.720021026545681e+34i;
t1810 = t24.*t25.*t262.*3.212809800067317e-5;
t1813 = t24.*t31.*t262.*3.212809800067317e-5;
t1814 = t25.*t30.*t262.*3.212809800067317e-5;
t1816 = t30.*t31.*t262.*3.212809800067317e-5;
t1819 = t24.*t25.*t33.*t264.*(-3.161027044821787e-5);
t1820 = t24.*t25.*t264.*3.596333474007969e-8;
t1821 = t24.*t31.*t33.*t264.*(-3.161027044821787e-5);
t1822 = t25.*t30.*t33.*t264.*(-3.161027044821787e-5);
t1823 = t24.*t31.*t264.*3.596333474007969e-8;
t1824 = t25.*t30.*t264.*3.596333474007969e-8;
t1825 = t24.*t25.*t33.*t264.*5.316843277159623e-5;
t1826 = t24.*t25.*t27.*t264.*1.166015146360021e-4;
t1827 = t30.*t31.*t264.*3.596333474007969e-8;
t1828 = t24.*t31.*t33.*t264.*5.316843277159623e-5;
t1829 = t25.*t30.*t33.*t264.*5.316843277159623e-5;
t1830 = t24.*t25.*t262.*5.403941802479429e-5;
t1831 = t24.*t27.*t31.*t264.*1.166015146360021e-4;
t1832 = t25.*t27.*t30.*t264.*1.166015146360021e-4;
t1834 = t30.*t31.*t33.*t264.*5.316843277159623e-5;
t1835 = t24.*t31.*t262.*5.403941802479429e-5;
t1836 = t25.*t30.*t262.*5.403941802479429e-5;
t1837 = t27.*t30.*t31.*t264.*1.166015146360021e-4;
t1840 = t30.*t31.*t262.*5.403941802479429e-5;
t1841 = t27.*t30.*t31.*t264.*(-6.932319085178867e-5);
t1842 = t26.*t27.*t50.*t240.*4.064789595703988e+32i;
t1843 = t24.*t25.*t264.*6.049028110982645e-8;
t1844 = t24.*t31.*t264.*6.049028110982645e-8;
t1845 = t25.*t30.*t264.*6.049028110982645e-8;
t1850 = t26.*t33.*t50.*t240.*1.618908833671003e+34i;
t1851 = t30.*t31.*t264.*6.049028110982645e-8;
t1856 = t32.*t33.*t34.*t50.*t240.*2.657049668350291e+37i;
t1858 = t28.*t32.*t33.*t50.*t240.*4.888570919953966e+37i;
t1860 = (t16.*t50.*t123.*t189)./8.112963841460668e+31;
t1861 = (t21.*t50.*t123.*t189)./8.112963841460668e+31;
t1862 = t26.*t27.*t34.*t50.*t240.*1.297387533374166e+34i;
t1866 = t26.*t27.*t28.*t50.*t240.*2.386997519508773e+34i;
t1878 = -t1872;
t1885 = -t1873;
t1888 = -t1874;
t1892 = -t1877;
t1900 = -t1879;
t1905 = -t1887;
t1906 = -t1889;
t1908 = t26.*t50.*t202.*(t46-t47).*(-1.232595164407831e-32);
t1910 = -t1895;
t1911 = -t1894;
t1913 = t32.*t50.*t202.*(t46-t47).*(-1.232595164407831e-32);
t1918 = -t1897;
t1921 = -t1899;
t1932 = -t1907;
t1933 = (t26.*t50.*t202.*(t46-t47))./8.112963841460668e+31;
t1934 = -t1916;
t1935 = -t1915;
t1938 = -t1919;
t1939 = -t1922;
t1944 = -t1928;
t1945 = -t1929;
t1946 = -t1930;
t1954 = -t1940;
t1955 = -t1941;
t1957 = -t1942;
t1962 = -t1947;
t1963 = -t1949;
t1964 = -t1950;
t1969 = -t1953;
t1972 = -t1959;
t1973 = t14.*t15.*t1924;
t1974 = t14.*t20.*t1922;
t1976 = t15.*t19.*t1922;
t1978 = -t1965;
t1979 = t14.*t20.*t1924;
t1980 = t15.*t19.*t1924;
t1981 = t19.*t20.*t1922;
t1983 = t14.*t15.*t16.*t1884;
t1984 = t14.*t15.*t21.*t1882;
t1985 = t19.*t20.*t1924;
t1986 = t14.*t15.*t21.*t1884;
t1987 = t14.*t16.*t20.*t1884;
t1988 = t14.*t20.*t21.*t1882;
t1989 = t15.*t16.*t19.*t1884;
t1990 = t15.*t19.*t21.*t1882;
t1992 = -t1967;
t1993 = t14.*t20.*t21.*t1884;
t1994 = t15.*t19.*t21.*t1884;
t1995 = t16.*t19.*t20.*t1884;
t1996 = t19.*t20.*t21.*t1882;
t1998 = -t1968;
t1999 = t19.*t20.*t21.*t1884;
t2000 = t14.*t15.*t16.*t1889;
t2001 = t14.*t15.*t21.*t1889;
t2002 = t14.*t16.*t20.*t1889;
t2003 = t15.*t16.*t19.*t1889;
t2004 = -t1970;
t2005 = t14.*t15.*t21.*t1890;
t2006 = t14.*t20.*t21.*t1889;
t2007 = t15.*t19.*t21.*t1889;
t2008 = t16.*t19.*t20.*t1889;
t2009 = t14.*t20.*t21.*t1890;
t2010 = t15.*t19.*t21.*t1890;
t2011 = t19.*t20.*t21.*t1889;
t2012 = t19.*t20.*t21.*t1890;
t2013 = t14.*t15.*t1909;
t2014 = t14.*t15.*t1915;
t2015 = t14.*t20.*t1909;
t2016 = t15.*t19.*t1909;
t2018 = t14.*t20.*t1915;
t2019 = t15.*t19.*t1915;
t2020 = t19.*t20.*t1909;
t2023 = t19.*t20.*t1915;
t2026 = t14.*t15.*t1922;
t2031 = -t1975;
t2033 = -t1977;
t2036 = -t1982;
t2037 = t14.*t15.*t1940;
t2040 = t14.*t15.*t1942;
t2041 = t14.*t20.*t1940;
t2042 = t15.*t19.*t1940;
t2046 = t14.*t20.*t1942;
t2047 = t15.*t19.*t1942;
t2048 = t19.*t20.*t1940;
t2053 = t19.*t20.*t1942;
t2060 = t14.*t15.*t1936;
t2064 = t14.*t15.*t1937;
t2065 = t14.*t20.*t1936;
t2066 = t15.*t19.*t1936;
t2067 = -t2021;
t2068 = -t2022;
t2070 = t14.*t20.*t1937;
t2071 = t15.*t19.*t1937;
t2072 = t19.*t20.*t1936;
t2073 = -t2024;
t2074 = -t2025;
t2076 = t19.*t20.*t1937;
t2078 = -t2038;
t2079 = -t2039;
t2094 = -t2055;
t2095 = -t2057;
t2106 = -t2080;
t2107 = -t2088;
t2108 = -t2092;
t2109 = -t2096;
t2110 = -t2097;
t2111 = -t2098;
t2112 = -t2099;
t2113 = t963+2.61156643317655e-1;
t2114 = t964+7.38843356682345e-1;
t2115 = t986+2.61156643317655e-1;
t2116 = t988+7.38843356682345e-1;
t2126 = -t2120;
t2127 = -t2122;
t2128 = -t2123;
t2129 = -t2124;
t2130 = t264.*(t46-t47).*(-1.875105520197095e-20);
t2136 = t264.*7.0482312e-7;
t2141 = -t2131;
t2144 = t264.*(t46-t47).*(-7.825108561121397e-23);
t2145 = -t2139;
t2146 = -t2140;
t2148 = t33.*t262.*6.1855407534e-5;
t2160 = t262.*(t46-t47).*(-2.075672598245148e-23);
t2161 = t27.*t262.*1.35652563578e-4;
t2162 = t264.*(t46-t47).*7.825108561121397e-23;
t2164 = -t2152;
t2165 = -t2153;
t2166 = -t2154;
t2167 = -t2155;
t2168 = -t2158;
t2169 = -t2159;
t2174 = t24.*t25.*t27.*t262.*3.542656816146526e-5;
t2175 = t24.*t25.*t33.*t262.*3.542656816146526e-5;
t2176 = t24.*t25.*t27.*t264.*3.542656816146526e-5;
t2177 = t24.*t27.*t31.*t262.*3.542656816146526e-5;
t2178 = t25.*t27.*t30.*t262.*3.542656816146526e-5;
t2179 = t24.*t31.*t33.*t262.*3.542656816146526e-5;
t2180 = t24.*t27.*t31.*t264.*3.542656816146526e-5;
t2181 = t25.*t30.*t33.*t262.*3.542656816146526e-5;
t2182 = t25.*t27.*t30.*t264.*3.542656816146526e-5;
t2183 = t27.*t30.*t31.*t262.*3.542656816146526e-5;
t2184 = t30.*t31.*t33.*t262.*3.542656816146526e-5;
t2185 = t27.*t30.*t31.*t264.*3.542656816146526e-5;
t2186 = t24.*t25.*t262.*1.641857854109028e-5;
t2187 = t24.*t25.*t264.*1.641857854109028e-5;
t2188 = t24.*t31.*t262.*1.641857854109028e-5;
t2189 = t25.*t30.*t262.*1.641857854109028e-5;
t2190 = t24.*t31.*t264.*1.641857854109028e-5;
t2191 = t25.*t30.*t264.*1.641857854109028e-5;
t2192 = t30.*t31.*t262.*1.641857854109028e-5;
t2193 = t30.*t31.*t264.*1.641857854109028e-5;
t2194 = t24.*t31.*t264.*2.761602722751607e-5;
t2195 = t25.*t30.*t264.*2.761602722751607e-5;
t2196 = t30.*t31.*t262.*2.761602722751607e-5;
t2197 = t24.*t25.*t27.*t262.*1.615395060262503e-5;
t2198 = t30.*t31.*t264.*2.761602722751607e-5;
t2199 = t24.*t25.*t33.*t262.*1.615395060262503e-5;
t2200 = t24.*t27.*t31.*t262.*1.615395060262503e-5;
t2201 = t25.*t27.*t30.*t262.*1.615395060262503e-5;
t2203 = t24.*t25.*t262.*1.837851826825065e-8;
t2204 = t24.*t25.*t33.*t264.*1.615395060262503e-5;
t2205 = t24.*t31.*t33.*t262.*1.615395060262503e-5;
t2206 = t25.*t30.*t33.*t262.*1.615395060262503e-5;
t2207 = t27.*t30.*t31.*t262.*1.615395060262503e-5;
t2209 = t24.*t25.*t264.*1.837851826825065e-8;
t2210 = t24.*t31.*t262.*1.837851826825065e-8;
t2211 = t25.*t30.*t262.*1.837851826825065e-8;
t2212 = t24.*t25.*t27.*t262.*5.958744043986595e-5;
t2213 = t24.*t31.*t33.*t264.*1.615395060262503e-5;
t2214 = t25.*t30.*t33.*t264.*1.615395060262503e-5;
t2215 = t30.*t31.*t33.*t262.*1.615395060262503e-5;
t2217 = t24.*t31.*t264.*1.837851826825065e-8;
t2218 = t25.*t30.*t264.*1.837851826825065e-8;
t2219 = t30.*t31.*t262.*1.837851826825065e-8;
t2220 = t24.*t25.*t33.*t262.*5.958744043986595e-5;
t2221 = t24.*t25.*t27.*t264.*5.958744043986595e-5;
t2222 = t24.*t27.*t31.*t262.*5.958744043986595e-5;
t2223 = t25.*t27.*t30.*t262.*5.958744043986595e-5;
t2224 = t30.*t31.*t33.*t264.*1.615395060262503e-5;
t2225 = t30.*t31.*t264.*1.837851826825065e-8;
t2226 = t24.*t31.*t33.*t262.*5.958744043986595e-5;
t2227 = t24.*t27.*t31.*t264.*5.958744043986595e-5;
t2228 = t25.*t30.*t33.*t262.*5.958744043986595e-5;
t2229 = t25.*t27.*t30.*t264.*5.958744043986595e-5;
t2230 = t27.*t30.*t31.*t262.*5.958744043986595e-5;
t2231 = t24.*t25.*t27.*t262.*2.71709233876478e-5;
t2232 = t30.*t31.*t33.*t262.*5.958744043986595e-5;
t2233 = t27.*t30.*t31.*t264.*5.958744043986595e-5;
t2234 = t24.*t25.*t33.*t262.*2.71709233876478e-5;
t2235 = t24.*t27.*t31.*t262.*2.71709233876478e-5;
t2236 = t25.*t27.*t30.*t262.*2.71709233876478e-5;
t2238 = t24.*t25.*t33.*t264.*2.71709233876478e-5;
t2239 = t24.*t31.*t33.*t262.*2.71709233876478e-5;
t2240 = t25.*t30.*t33.*t262.*2.71709233876478e-5;
t2241 = t27.*t30.*t31.*t262.*2.71709233876478e-5;
t2244 = t24.*t31.*t33.*t264.*2.71709233876478e-5;
t2245 = t25.*t30.*t33.*t264.*2.71709233876478e-5;
t2246 = t30.*t31.*t33.*t262.*2.71709233876478e-5;
t2247 = t30.*t31.*t33.*t264.*2.71709233876478e-5;
t2249 = t24.*t25.*t262.*2.761602722751607e-5;
t2250 = t24.*t25.*t264.*2.761602722751607e-5;
t2251 = t24.*t31.*t262.*2.761602722751607e-5;
t2252 = t25.*t30.*t262.*2.761602722751607e-5;
t2253 = t24.*t25.*t262.*3.091264323687963e-8;
t2255 = t24.*t25.*t264.*3.091264323687963e-8;
t2256 = t24.*t31.*t262.*3.091264323687963e-8;
t2257 = t25.*t30.*t262.*3.091264323687963e-8;
t2259 = t24.*t31.*t264.*3.091264323687963e-8;
t2260 = t25.*t30.*t264.*3.091264323687963e-8;
t2261 = t30.*t31.*t262.*3.091264323687963e-8;
t2263 = t30.*t31.*t264.*3.091264323687963e-8;
t2290 = t16.*t50.*t123.*t189.*7.204296868834178e-35;
t2291 = t21.*t50.*t123.*t189.*7.204296868834178e-35;
t2292 = t16.*t50.*t123.*t189.*7.987216665362745e-37;
t2295 = t21.*t50.*t123.*t189.*7.987216665362745e-37;
t2297 = t238+t1454;
t2304 = t21.*t50.*t123.*t189.*7.974890713718666e-38;
t2311 = t16.*t50.*t123.*t189.*7.974890713718666e-38;
t2320 = -t2308;
t2333 = -t2318;
t2336 = -t2319;
t2341 = -t2326;
t2343 = -t2329;
t2347 = -t2330;
t2363 = t264+t1474;
t2370 = t26.*t50.*t202.*(t46-t47).*(-7.204296868834178e-35);
t2372 = t32.*t50.*t202.*(t46-t47).*(-7.204296868834178e-35);
t2375 = -t2348;
t2377 = -t2349;
t2379 = -t2352;
t2380 = -t2353;
t2384 = -t2359;
t2385 = -t2361;
t2386 = -t2362;
t2389 = -t2364;
t2394 = -t2365;
t2395 = -t2366;
t2396 = -t2367;
t2398 = t26.*t50.*t202.*(t46-t47).*(-7.987216665362745e-37);
t2401 = t32.*t50.*t202.*(t46-t47).*(-7.987216665362745e-37);
t2403 = t32.*t50.*t202.*(t46-t47).*7.204296868834178e-35;
t2408 = -t2383;
t2413 = -t2392;
t2414 = -t2393;
t2422 = -t2406;
t2425 = -t2407;
t2450 = -t2415;
t2458 = -t2420;
t2462 = t26.*t50.*t202.*(t46-t47).*(-7.974890713718666e-38);
t2464 = t32.*t50.*t202.*(t46-t47).*(-7.974890713718666e-38);
t2472 = -t2428;
t2473 = -t2429;
t2474 = -t2430;
t2476 = -t2435;
t2477 = -t2436;
t2478 = -t2437;
t2479 = -t2439;
t2480 = -t2442;
t2481 = -t2443;
t2489 = -t2454;
t2490 = -t2453;
t2492 = -t2456;
t2493 = t26.*t50.*t202.*(t46-t47).*7.974890713718666e-38;
t2494 = t32.*t50.*t202.*(t46-t47).*7.974890713718666e-38;
t2504 = -t2469;
t2508 = -t2475;
t2509 = t35.*t50.*t265.*6.209141233430105e-19i;
t2510 = t36.*t50.*t265.*6.209141233430105e-19i;
t2511 = -t2483;
t2514 = -t2486;
t2516 = -t2495;
t2518 = t188.*t201.*(t46-t47).*(-2.442490654175345e-23);
t2520 = t189.*t202.*(t46-t47).*(-2.442490654175345e-23);
t2524 = -t2513;
t2525 = t188.*t201.*(t46-t47).*2.442490654175345e-23;
t2530 = t35.*t50.*t265.*3.200438707086705e-18i;
t2532 = t36.*t50.*t265.*3.200438707086705e-18i;
t2540 = t24.*t25.*t2483;
t2542 = t24.*t25.*t2484;
t2543 = t24.*t31.*t2483;
t2545 = t25.*t30.*t2483;
t2548 = t24.*t31.*t2484;
t2549 = t25.*t30.*t2484;
t2550 = t30.*t31.*t2483;
t2552 = t24.*t25.*t2451;
t2555 = t30.*t31.*t2484;
t2556 = t24.*t25.*t2453;
t2557 = t24.*t31.*t2451;
t2558 = t25.*t30.*t2451;
t2559 = t24.*t25.*t2455;
t2561 = t24.*t31.*t2453;
t2562 = t25.*t30.*t2453;
t2563 = t30.*t31.*t2451;
t2564 = t24.*t25.*t2457;
t2565 = t24.*t31.*t2455;
t2566 = t25.*t30.*t2455;
t2569 = t30.*t31.*t2453;
t2570 = t24.*t31.*t2457;
t2571 = t25.*t30.*t2457;
t2572 = t30.*t31.*t2455;
t2574 = t30.*t31.*t2457;
t2578 = t24.*t25.*t2512;
t2580 = -t2544;
t2582 = -t2546;
t2583 = t24.*t25.*t2513;
t2584 = t24.*t31.*t2512;
t2585 = t25.*t30.*t2512;
t2589 = -t2551;
t2590 = t24.*t31.*t2513;
t2591 = t25.*t30.*t2513;
t2592 = t30.*t31.*t2512;
t2604 = t30.*t31.*t2513;
t2629 = -t2567;
t2630 = -t2568;
t2634 = -t2573;
t2644 = -t2588;
t2648 = -t2593;
t2649 = -t2594;
t2650 = -t2596;
t2654 = -t2607;
t2655 = -t2608;
t2657 = -t2609;
t2658 = -t2612;
t2659 = -t2613;
t2660 = -t2617;
t2661 = -t2625;
t2662 = -t2631;
t2665 = -t2639;
t2666 = -t2651;
t2667 = -t2652;
t2668 = -t2656;
t2699 = t850+t874;
t2718 = t855+t878;
t2731 = -t2726;
t2734 = -t2727;
t2741 = t26.*t50.*t202.*(t46-t47).*(-2.081785322124547e-36);
t2742 = t32.*t50.*t202.*(t46-t47).*(-2.081785322124547e-36);
t2753 = t26.*t50.*t202.*(t46-t47).*2.081785322124547e-36;
t2754 = t32.*t50.*t202.*(t46-t47).*2.081785322124547e-36;
t2759 = t32.*t50.*t202.*(t46-t47).*(-8.687615694748404e-39);
t2762 = -t2745;
t2769 = t26.*t50.*t202.*(t46-t47).*(-8.687615694748404e-39);
t2790 = t26.*t50.*t202.*(t46-t47).*(-2.304459510155286e-39);
t2792 = t32.*t50.*t202.*(t46-t47).*(-2.304459510155286e-39);
t2795 = -t2773;
t2796 = -t2774;
t2798 = -t2777;
t2799 = -t2778;
t2802 = -t2779;
t2803 = -t2780;
t2805 = -t2781;
t2807 = -t2782;
t2808 = -t2783;
t2811 = -t2785;
t2812 = -t2786;
t2814 = t26.*t50.*t202.*(t46-t47).*2.304459510155286e-39;
t2823 = -t2800;
t2893 = -t2860;
t2911 = -t2872;
t2914 = -t2879;
t2920 = -t2887;
t2922 = -t2891;
t2923 = -t2892;
t2925 = -t2896;
t2926 = -t2899;
t2930 = -t2906;
t2931 = -t2907;
t2933 = -t2908;
t2935 = -t2915;
t2962 = t50.*t188.*t202.*(t46-t47).*(-2.711709361697228e-39);
t2965 = -t2959;
t2966 = -t2960;
t2969 = -t2967;
t2970 = -t2968;
t3940 = t175+t210+t219+t433+t472+t477+t867+t897+t901+t1242+t1291+t1295;
t3961 = t166+t190+t403+t427+t431+t446+t851+t875+t1184+t1197+t1202+t1256;
t4220 = t52+t77+t84+t85+t122+t125+t245+t294+t296+t520+t548+t559+t560+t591+t619+t909+t952+t954;
t4280 = t145+t157+t171+t181+t390+t407+t415+t440+t840+t845+t854+t864+t1166+t1170+t1223+t1254;
t4295 = t64+t65+t96+t104+t115+t246+t247+t266+t298+t299+t532+t533+t561+t566+t595+t913+t920+t938+t946+t957;
t4644 = t51+t69+t75+t80+t81+t82+t93+t118+t233+t251+t269+t282+t289+t515+t519+t537+t545+t554+t555+t557+t570+t599+t923+t929+t939+t975+t977+3.064357668490995e+34;
tau_c = ft_5({t100,t1000,t1001,t1002,t1003,t1006,t1009,t101,t1011,t1014,t1015,t1017,t1018,t1019,t1020,t1021,t1023,t1024,t1025,t1028,t1029,t103,t1030,t1031,t1032,t1035,t1038,t1039,t1041,t1042,t1044,t1045,t1046,t1048,t1049,t1050,t1051,t1052,t1055,t1056,t1057,t1058,t1059,t106,t1061,t1062,t1065,t1066,t1067,t107,t1070,t1071,t1072,t1073,t1074,t1075,t1076,t108,t1080,t1083,t1084,t1089,t109,t1090,t1091,t1092,t1094,t1095,t1098,t1099,t110,t1100,t1102,t1103,t1104,t1105,t1106,t1107,t1108,t1109,t111,t1110,t1111,t1112,t1113,t1114,t1115,t1116,t1117,t1118,t1119,t1120,t1121,t1122,t1123,t1124,t1125,t1126,t1129,t113,t1132,t1135,t1137,t1138,t1139,t114,t1140,t1141,t1142,t1144,t1145,t1146,t1147,t1148,t1149,t1150,t1154,t1158,t1159,t1162,t1165,t1167,t1174,t1176,t1177,t1178,t1179,t1180,t1185,t1186,t1187,t1188,t1189,t1190,t1192,t1193,t1194,t1195,t1196,t1198,t1199,t120,t1203,t1204,t1205,t1206,t1207,t1208,t1209,t121,t1210,t1212,t1213,t1214,t1217,t1218,t1219,t1220,t1221,t1222,t1224,t1229,t123,t1230,t1232,t1234,t1235,t1236,t1237,t1238,t124,t1241,t1245,t1246,t1247,t1248,t1251,t1252,t1253,t1255,t1259,t126,t1260,t1261,t1262,t1263,t1264,t1265,t1266,t1267,t1268,t127,t1270,t1271,t1272,t1277,t1278,t128,t1280,t1281,t1285,t1286,t1287,t1288,t1289,t1290,t1292,t1294,t1296,t1297,t1298,t1299,t130,t1300,t1301,t1302,t1303,t1304,t1305,t1307,t1310,t1311,t1316,t1317,t1319,t132,t1320,t1322,t1323,t1324,t1325,t1326,t1328,t133,t1330,t1331,t1332,t1334,t1335,t1336,t1337,t1338,t134,t1342,t1343,t1344,t1345,t1348,t1349,t1350,t1351,t1352,t1353,t1354,t136,t1360,t1364,t1366,t1367,t1368,t1369,t1370,t1371,t1372,t1374,t1375,t1376,t1377,t1378,t1379,t138,t1380,t1383,t1385,t1386,t1387,t1388,t1389,t139,t1392,t1393,t1394,t1395,t1396,t1397,t1398,t1399,t14,t140,t1401,t1402,t1403,t1404,t1405,t1406,t1407,t1408,t1409,t1410,t1411,t1412,t1413,t1414,t1415,t1416,t1417,t1418,t1419,t1420,t1421,t1422,t1423,t1424,t1425,t1426,t1427,t1428,t1429,t1430,t1431,t1432,t1433,t1434,t1435,t1436,t1437,t1439,t144,t1440,t1441,t1443,t1444,t1445,t1446,t1447,t1448,t1451,t1453,t1456,t1457,t1458,t1459,t1460,t1461,t1462,t1463,t1464,t1468,t1469,t1471,t1477,t1478,t1479,t148,t1480,t1481,t1482,t1483,t1484,t1485,t1486,t1487,t1488,t1489,t149,t1490,t1491,t1492,t1493,t1494,t1495,t1497,t1498,t1499,t15,t150,t1500,t1501,t1503,t1504,t1505,t1506,t1507,t1509,t151,t1510,t1512,t1513,t1514,t1515,t1516,t1517,t1518,t1519,t152,t1520,t1522,t1523,t1525,t1526,t1527,t1528,t1529,t153,t1530,t1531,t1532,t1533,t1535,t1536,t1537,t1538,t1539,t1541,t1542,t1543,t1544,t1545,t1546,t1547,t1549,t1550,t1551,t1552,t1554,t1555,t1556,t1558,t1559,t156,t1560,t1565,t1567,t1568,t1569,t1570,t1571,t1572,t1574,t1575,t1576,t1577,t1578,t1579,t158,t1581,t1582,t1583,t1584,t1585,t1586,t1587,t1588,t1591,t1592,t1593,t1594,t1595,t1596,t1599,t16,t160,t1600,t1601,t1602,t1604,t1605,t1606,t1607,t1608,t1609,t161,t1613,t1614,t1615,t1616,t1618,t1619,t162,t1620,t1621,t1622,t1624,t1625,t1626,t1627,t1628,t1629,t1631,t1633,t1634,t1635,t1636,t1637,t1639,t1640,t1641,t1642,t1643,t1644,t1645,t1646,t1648,t1649,t165,t1650,t1651,t1652,t1653,t1654,t1655,t1656,t1657,t1658,t1659,t1660,t1661,t1662,t1663,t1664,t1665,t1666,t1667,t1668,t1669,t167,t1670,t1671,t1672,t1673,t1674,t1675,t1676,t1677,t1678,t1679,t168,t1680,t1681,t1682,t1683,t1684,t1685,t1686,t1687,t1690,t1691,t1692,t1693,t1694,t1695,t1696,t1697,t1698,t1699,t17,t170,t1700,t1701,t1704,t1705,t1706,t1707,t1708,t1710,t1711,t1712,t1716,t1717,t172,t173,t1738,t1739,t174,t1740,t1741,t1742,t1743,t1745,t1749,t1750,t1751,t1752,t1753,t1754,t1756,t1757,t1758,t1759,t176,t1760,t1761,t1762,t1764,t1765,t1766,t1768,t1769,t177,t1770,t1771,t1772,t1773,t1775,t1776,t1777,t1779,t178,t1786,t1793,t1794,t1795,t1796,t1797,t1799,t18,t180,t1800,t1801,t1802,t1807,t1810,t1813,t1814,t1816,t1817,t1819,t182,t1820,t1821,t1822,t1823,t1824,t1825,t1826,t1827,t1828,t1829,t1830,t1831,t1832,t1834,t1835,t1836,t1837,t1840,t1841,t1842,t1843,t1844,t1845,t185,t1850,t1851,t1856,t1858,t186,t1860,t1861,t1862,t1865,t1866,t1868,t1870,t1871,t1874,t1875,t1876,t1878,t1879,t188,t1880,t1881,t1882,t1883,t1884,t1885,t1886,t1887,t1888,t1889,t189,t1890,t1891,t1892,t1898,t19,t1900,t1901,t1902,t1903,t1904,t1905,t1906,t1909,t191,t1910,t1911,t1913,t1914,t1917,t1918,t192,t1920,t1921,t1923,t1924,t1925,t1926,t1927,t1929,t1930,t1931,t1932,t1933,t1934,t1935,t1936,t1937,t1938,t1939,t1940,t1941,t1943,t1944,t1945,t1946,t1948,t195,t1951,t1952,t1953,t1954,t1955,t1956,t1957,t1958,t1959,t196,t1960,t1961,t1962,t1963,t1964,t1966,t1967,t1969,t197,t1971,t1972,t1973,t1978,t1979,t198,t1980,t1981,t1983,t1984,t1985,t1988,t1990,t1991,t1992,t1993,t1994,t1997,t1998,t1999,t2,t20,t2001,t2002,t2003,t2004,t2005,t2006,t2007,t2008,t2009,t201,t2010,t2013,t2014,t2015,t2016,t2017,t202,t2023,t2024,t2027,t2028,t2029,t203,t2030,t2031,t2032,t2033,t2034,t2035,t2036,t2037,t2039,t204,t2040,t2041,t2042,t2043,t2044,t2045,t2049,t205,t2050,t2051,t2052,t2053,t2054,t2056,t2057,t2058,t2059,t2060,t2061,t2062,t2063,t2064,t2065,t2066,t2067,t2068,t2069,t207,t2070,t2071,t2072,t2073,t2074,t2075,t2077,t2078,t2079,t208,t2081,t2082,t2083,t2084,t2085,t2086,t2087,t2089,t209,t2090,t2091,t2093,t2094,t2095,t2098,t2099,t21,t2100,t2101,t2102,t2103,t2104,t2105,t2106,t2107,t2108,t2109,t211,t2110,t2111,t2112,t2113,t2114,t2115,t2116,t2117,t2118,t2119,t212,t2120,t2121,t2122,t2123,t2126,t2127,t2128,t2129,t2130,t2136,t2138,t2139,t2140,t2141,t2145,t2146,t2147,t2148,t2149,t2150,t2151,t2152,t2153,t2154,t2155,t2156,t2157,t2159,t216,t2160,t2161,t2162,t2164,t2165,t2166,t2167,t2168,t2169,t217,t2174,t2175,t2176,t2177,t2178,t2179,t218,t2180,t2181,t2182,t2183,t2184,t2185,t2186,t2187,t2188,t2189,t2190,t2191,t2192,t2193,t2194,t2195,t2196,t2197,t2198,t2199,t22,t2200,t2201,t2203,t2204,t2205,t2206,t2207,t2209,t221,t2210,t2211,t2212,t2213,t2214,t2215,t2217,t2218,t2219,t2220,t2221,t2222,t2223,t2224,t2225,t2226,t2227,t2228,t2229,t223,t2230,t2231,t2232,t2233,t2234,t2235,t2236,t2238,t2239,t2240,t2241,t2244,t2245,t2246,t2247,t2249,t225,t2250,t2251,t2252,t2253,t2255,t2256,t2257,t2259,t226,t2260,t2261,t2263,t227,t229,t2290,t2291,t2292,t2294,t2295,t2296,t2297,t2299,t23,t230,t2300,t2302,t2303,t2304,t2305,t2306,t2308,t2309,t231,t2310,t2311,t2313,t2314,t2315,t2316,t2317,t2320,t2322,t2323,t2324,t2325,t2326,t2327,t2328,t2329,t2331,t2332,t2333,t2334,t2336,t2339,t2340,t2341,t2343,t2345,t2346,t2347,t2352,t2353,t2354,t2357,t2358,t2359,t236,t2360,t2361,t2362,t2363,t2364,t2365,t2366,t2367,t237,t2370,t2374,t2375,t2377,t2378,t2379,t238,t2380,t2382,t2384,t2385,t2386,t2389,t239,t2391,t2393,t2394,t2395,t2396,t2398,t24,t240,t2401,t2402,t2403,t2404,t2405,t2408,t2409,t241,t2411,t2413,t2414,t2416,t2417,t2418,t242,t2422,t2425,t2426,t2427,t243,t2431,t2432,t2433,t2434,t2438,t244,t2440,t2441,t2444,t2446,t2447,t2448,t2449,t2450,t2451,t2452,t2455,t2457,t2458,t2459,t2460,t2461,t2463,t2466,t2467,t2471,t2472,t2473,t2474,t2476,t2477,t2478,t2479,t2480,t2481,t2482,t2484,t2485,t2487,t2488,t2489,t2490,t2491,t2492,t2493,t2494,t2498,t2499,t25,t2504,t2505,t2508,t2509,t2510,t2511,t2512,t2514,t2515,t2516,t2520,t2524,t2525,t2529,t2530,t2532,t2541,t2542,t2548,t2549,t2550,t2552,t2555,t2556,t2557,t2558,t2559,t2560,t2564,t2565,t2566,t2569,t257,t2570,t2571,t2572,t2577,t2578,t2579,t2580,t2581,t2582,t2583,t2584,t2585,t2586,t2587,t2589,t259,t2595,t2597,t2599,t26,t260,t2600,t2601,t2603,t2604,t2605,t2606,t261,t2610,t2611,t2612,t2613,t2614,t2616,t2618,t2619,t262,t2620,t2621,t2622,t2623,t2624,t2626,t2627,t2628,t2629,t263,t2630,t2632,t2633,t2634,t2635,t264,t2640,t2641,t2642,t2643,t2644,t2645,t2646,t2647,t2648,t2649,t2650,t2651,t2652,t2653,t2654,t2655,t2657,t2658,t2659,t2660,t2661,t2662,t2665,t2666,t2667,t2668,t267,t268,t2699,t27,t270,t271,t2718,t272,t2723,t2724,t2725,t2728,t2729,t273,t2730,t2731,t2734,t2735,t2736,t274,t2742,t2745,t2748,t2749,t275,t2750,t2753,t2754,t2759,t276,t2762,t2769,t2773,t2774,t2775,t2777,t2778,t2779,t2781,t2785,t2786,t2787,t2788,t279,t2790,t2792,t2795,t2796,t2797,t2798,t2799,t28,t280,t2802,t2803,t2805,t2807,t2808,t2811,t2812,t2814,t2823,t283,t285,t2857,t2858,t2859,t286,t2865,t2867,t2868,t2883,t2884,t2886,t2890,t2893,t2894,t2895,t2898,t2900,t2901,t2903,t2905,t291,t2911,t2914,t2917,t2918,t2919,t292,t2920,t2922,t2923,t2925,t2926,t293,t2930,t2931,t2933,t2935,t295,t2962,t2963,t2964,t2965,t2966,t2969,t297,t2970,t3,t30,t301,t303,t305,t306,t308,t309,t31,t310,t311,t312,t313,t314,t315,t316,t318,t319,t32,t320,t321,t322,t323,t325,t326,t328,t329,t33,t330,t331,t332,t333,t335,t336,t337,t338,t339,t34,t341,t343,t346,t348,t35,t350,t351,t352,t354,t355,t356,t358,t359,t36,t360,t361,t362,t363,t364,t365,t366,t368,t369,t370,t371,t372,t373,t377,t378,t38,t380,t381,t382,t385,t386,t387,t388,t389,t39,t391,t392,t393,t3940,t396,t3961,t4,t404,t406,t408,t410,t411,t412,t413,t414,t419,t42,t420,t421,t422,t4220,t424,t425,t426,t428,t4280,t429,t4295,t43,t430,t432,t434,t435,t437,t438,t439,t444,t445,t448,t451,t452,t455,t456,t457,t458,t459,t46,t461,t463,t464,t4644,t465,t466,t467,t468,t469,t47,t471,t473,t474,t476,t478,t479,t480,t483,t485,t486,t488,t489,t49,t490,t491,t493,t494,t495,t496,t497,t498,t5,t50,t503,t504,t506,t507,t508,t509,t510,t511,t512,t513,t514,t516,t517,t518,t521,t522,t523,t524,t525,t526,t527,t528,t53,t530,t531,t536,t538,t539,t54,t540,t542,t543,t544,t546,t547,t550,t551,t552,t553,t556,t56,t562,t563,t565,t568,t569,t571,t572,t573,t574,t575,t576,t577,t578,t58,t580,t582,t583,t584,t585,t589,t59,t590,t592,t597,t6,t60,t600,t601,t605,t606,t607,t608,t609,t610,t611,t612,t614,t615,t616,t618,t620,t621,t622,t623,t624,t625,t627,t628,t629,t63,t631,t634,t635,t636,t638,t640,t641,t642,t643,t645,t646,t648,t649,t650,t651,t652,t654,t655,t656,t657,t658,t659,t660,t662,t663,t664,t665,t666,t667,t668,t669,t67,t670,t672,t673,t674,t675,t676,t677,t678,t679,t68,t681,t682,t683,t684,t685,t686,t687,t689,t691,t692,t693,t694,t696,t698,t7,t70,t701,t702,t704,t705,t707,t708,t71,t710,t711,t712,t713,t714,t715,t716,t717,t718,t719,t720,t721,t722,t723,t724,t725,t726,t728,t73,t733,t735,t736,t738,t739,t740,t741,t742,t743,t744,t745,t746,t747,t749,t750,t751,t755,t756,t757,t758,t759,t76,t762,t763,t764,t765,t766,t767,t768,t770,t771,t772,t773,t774,t775,t776,t777,t778,t78,t781,t782,t783,t784,t785,t786,t787,t789,t79,t790,t791,t792,t793,t794,t796,t797,t798,t799,t800,t801,t802,t806,t807,t808,t809,t812,t813,t816,t817,t818,t819,t820,t821,t822,t823,t824,t825,t826,t827,t828,t829,t830,t831,t832,t833,t836,t837,t838,t839,t841,t844,t846,t850,t852,t853,t855,t856,t857,t858,t859,t860,t861,t863,t865,t866,t868,t869,t870,t871,t872,t874,t876,t877,t878,t881,t882,t883,t885,t887,t889,t89,t890,t891,t893,t894,t895,t896,t898,t90,t900,t902,t903,t904,t905,t906,t907,t908,t91,t911,t912,t914,t915,t916,t917,t918,t92,t921,t924,t926,t927,t930,t932,t933,t934,t935,t936,t937,t94,t940,t942,t943,t944,t945,t947,t948,t950,t951,t956,t959,t960,t961,t962,t965,t966,t967,t969,t97,t970,t974,t976,t978,t981,t983,t985,t987,t989,t99,t990,t992,t993,t994,t995,t996,t997,t998,t999});
end
function tau_c = ft_5(ct)
t100 = ct{1};
t1000 = ct{2};
t1001 = ct{3};
t1002 = ct{4};
t1003 = ct{5};
t1006 = ct{6};
t1009 = ct{7};
t101 = ct{8};
t1011 = ct{9};
t1014 = ct{10};
t1015 = ct{11};
t1017 = ct{12};
t1018 = ct{13};
t1019 = ct{14};
t1020 = ct{15};
t1021 = ct{16};
t1023 = ct{17};
t1024 = ct{18};
t1025 = ct{19};
t1028 = ct{20};
t1029 = ct{21};
t103 = ct{22};
t1030 = ct{23};
t1031 = ct{24};
t1032 = ct{25};
t1035 = ct{26};
t1038 = ct{27};
t1039 = ct{28};
t1041 = ct{29};
t1042 = ct{30};
t1044 = ct{31};
t1045 = ct{32};
t1046 = ct{33};
t1048 = ct{34};
t1049 = ct{35};
t1050 = ct{36};
t1051 = ct{37};
t1052 = ct{38};
t1055 = ct{39};
t1056 = ct{40};
t1057 = ct{41};
t1058 = ct{42};
t1059 = ct{43};
t106 = ct{44};
t1061 = ct{45};
t1062 = ct{46};
t1065 = ct{47};
t1066 = ct{48};
t1067 = ct{49};
t107 = ct{50};
t1070 = ct{51};
t1071 = ct{52};
t1072 = ct{53};
t1073 = ct{54};
t1074 = ct{55};
t1075 = ct{56};
t1076 = ct{57};
t108 = ct{58};
t1080 = ct{59};
t1083 = ct{60};
t1084 = ct{61};
t1089 = ct{62};
t109 = ct{63};
t1090 = ct{64};
t1091 = ct{65};
t1092 = ct{66};
t1094 = ct{67};
t1095 = ct{68};
t1098 = ct{69};
t1099 = ct{70};
t110 = ct{71};
t1100 = ct{72};
t1102 = ct{73};
t1103 = ct{74};
t1104 = ct{75};
t1105 = ct{76};
t1106 = ct{77};
t1107 = ct{78};
t1108 = ct{79};
t1109 = ct{80};
t111 = ct{81};
t1110 = ct{82};
t1111 = ct{83};
t1112 = ct{84};
t1113 = ct{85};
t1114 = ct{86};
t1115 = ct{87};
t1116 = ct{88};
t1117 = ct{89};
t1118 = ct{90};
t1119 = ct{91};
t1120 = ct{92};
t1121 = ct{93};
t1122 = ct{94};
t1123 = ct{95};
t1124 = ct{96};
t1125 = ct{97};
t1126 = ct{98};
t1129 = ct{99};
t113 = ct{100};
t1132 = ct{101};
t1135 = ct{102};
t1137 = ct{103};
t1138 = ct{104};
t1139 = ct{105};
t114 = ct{106};
t1140 = ct{107};
t1141 = ct{108};
t1142 = ct{109};
t1144 = ct{110};
t1145 = ct{111};
t1146 = ct{112};
t1147 = ct{113};
t1148 = ct{114};
t1149 = ct{115};
t1150 = ct{116};
t1154 = ct{117};
t1158 = ct{118};
t1159 = ct{119};
t1162 = ct{120};
t1165 = ct{121};
t1167 = ct{122};
t1174 = ct{123};
t1176 = ct{124};
t1177 = ct{125};
t1178 = ct{126};
t1179 = ct{127};
t1180 = ct{128};
t1185 = ct{129};
t1186 = ct{130};
t1187 = ct{131};
t1188 = ct{132};
t1189 = ct{133};
t1190 = ct{134};
t1192 = ct{135};
t1193 = ct{136};
t1194 = ct{137};
t1195 = ct{138};
t1196 = ct{139};
t1198 = ct{140};
t1199 = ct{141};
t120 = ct{142};
t1203 = ct{143};
t1204 = ct{144};
t1205 = ct{145};
t1206 = ct{146};
t1207 = ct{147};
t1208 = ct{148};
t1209 = ct{149};
t121 = ct{150};
t1210 = ct{151};
t1212 = ct{152};
t1213 = ct{153};
t1214 = ct{154};
t1217 = ct{155};
t1218 = ct{156};
t1219 = ct{157};
t1220 = ct{158};
t1221 = ct{159};
t1222 = ct{160};
t1224 = ct{161};
t1229 = ct{162};
t123 = ct{163};
t1230 = ct{164};
t1232 = ct{165};
t1234 = ct{166};
t1235 = ct{167};
t1236 = ct{168};
t1237 = ct{169};
t1238 = ct{170};
t124 = ct{171};
t1241 = ct{172};
t1245 = ct{173};
t1246 = ct{174};
t1247 = ct{175};
t1248 = ct{176};
t1251 = ct{177};
t1252 = ct{178};
t1253 = ct{179};
t1255 = ct{180};
t1259 = ct{181};
t126 = ct{182};
t1260 = ct{183};
t1261 = ct{184};
t1262 = ct{185};
t1263 = ct{186};
t1264 = ct{187};
t1265 = ct{188};
t1266 = ct{189};
t1267 = ct{190};
t1268 = ct{191};
t127 = ct{192};
t1270 = ct{193};
t1271 = ct{194};
t1272 = ct{195};
t1277 = ct{196};
t1278 = ct{197};
t128 = ct{198};
t1280 = ct{199};
t1281 = ct{200};
t1285 = ct{201};
t1286 = ct{202};
t1287 = ct{203};
t1288 = ct{204};
t1289 = ct{205};
t1290 = ct{206};
t1292 = ct{207};
t1294 = ct{208};
t1296 = ct{209};
t1297 = ct{210};
t1298 = ct{211};
t1299 = ct{212};
t130 = ct{213};
t1300 = ct{214};
t1301 = ct{215};
t1302 = ct{216};
t1303 = ct{217};
t1304 = ct{218};
t1305 = ct{219};
t1307 = ct{220};
t1310 = ct{221};
t1311 = ct{222};
t1316 = ct{223};
t1317 = ct{224};
t1319 = ct{225};
t132 = ct{226};
t1320 = ct{227};
t1322 = ct{228};
t1323 = ct{229};
t1324 = ct{230};
t1325 = ct{231};
t1326 = ct{232};
t1328 = ct{233};
t133 = ct{234};
t1330 = ct{235};
t1331 = ct{236};
t1332 = ct{237};
t1334 = ct{238};
t1335 = ct{239};
t1336 = ct{240};
t1337 = ct{241};
t1338 = ct{242};
t134 = ct{243};
t1342 = ct{244};
t1343 = ct{245};
t1344 = ct{246};
t1345 = ct{247};
t1348 = ct{248};
t1349 = ct{249};
t1350 = ct{250};
t1351 = ct{251};
t1352 = ct{252};
t1353 = ct{253};
t1354 = ct{254};
t136 = ct{255};
t1360 = ct{256};
t1364 = ct{257};
t1366 = ct{258};
t1367 = ct{259};
t1368 = ct{260};
t1369 = ct{261};
t1370 = ct{262};
t1371 = ct{263};
t1372 = ct{264};
t1374 = ct{265};
t1375 = ct{266};
t1376 = ct{267};
t1377 = ct{268};
t1378 = ct{269};
t1379 = ct{270};
t138 = ct{271};
t1380 = ct{272};
t1383 = ct{273};
t1385 = ct{274};
t1386 = ct{275};
t1387 = ct{276};
t1388 = ct{277};
t1389 = ct{278};
t139 = ct{279};
t1392 = ct{280};
t1393 = ct{281};
t1394 = ct{282};
t1395 = ct{283};
t1396 = ct{284};
t1397 = ct{285};
t1398 = ct{286};
t1399 = ct{287};
t14 = ct{288};
t140 = ct{289};
t1401 = ct{290};
t1402 = ct{291};
t1403 = ct{292};
t1404 = ct{293};
t1405 = ct{294};
t1406 = ct{295};
t1407 = ct{296};
t1408 = ct{297};
t1409 = ct{298};
t1410 = ct{299};
t1411 = ct{300};
t1412 = ct{301};
t1413 = ct{302};
t1414 = ct{303};
t1415 = ct{304};
t1416 = ct{305};
t1417 = ct{306};
t1418 = ct{307};
t1419 = ct{308};
t1420 = ct{309};
t1421 = ct{310};
t1422 = ct{311};
t1423 = ct{312};
t1424 = ct{313};
t1425 = ct{314};
t1426 = ct{315};
t1427 = ct{316};
t1428 = ct{317};
t1429 = ct{318};
t1430 = ct{319};
t1431 = ct{320};
t1432 = ct{321};
t1433 = ct{322};
t1434 = ct{323};
t1435 = ct{324};
t1436 = ct{325};
t1437 = ct{326};
t1439 = ct{327};
t144 = ct{328};
t1440 = ct{329};
t1441 = ct{330};
t1443 = ct{331};
t1444 = ct{332};
t1445 = ct{333};
t1446 = ct{334};
t1447 = ct{335};
t1448 = ct{336};
t1451 = ct{337};
t1453 = ct{338};
t1456 = ct{339};
t1457 = ct{340};
t1458 = ct{341};
t1459 = ct{342};
t1460 = ct{343};
t1461 = ct{344};
t1462 = ct{345};
t1463 = ct{346};
t1464 = ct{347};
t1468 = ct{348};
t1469 = ct{349};
t1471 = ct{350};
t1477 = ct{351};
t1478 = ct{352};
t1479 = ct{353};
t148 = ct{354};
t1480 = ct{355};
t1481 = ct{356};
t1482 = ct{357};
t1483 = ct{358};
t1484 = ct{359};
t1485 = ct{360};
t1486 = ct{361};
t1487 = ct{362};
t1488 = ct{363};
t1489 = ct{364};
t149 = ct{365};
t1490 = ct{366};
t1491 = ct{367};
t1492 = ct{368};
t1493 = ct{369};
t1494 = ct{370};
t1495 = ct{371};
t1497 = ct{372};
t1498 = ct{373};
t1499 = ct{374};
t15 = ct{375};
t150 = ct{376};
t1500 = ct{377};
t1501 = ct{378};
t1503 = ct{379};
t1504 = ct{380};
t1505 = ct{381};
t1506 = ct{382};
t1507 = ct{383};
t1509 = ct{384};
t151 = ct{385};
t1510 = ct{386};
t1512 = ct{387};
t1513 = ct{388};
t1514 = ct{389};
t1515 = ct{390};
t1516 = ct{391};
t1517 = ct{392};
t1518 = ct{393};
t1519 = ct{394};
t152 = ct{395};
t1520 = ct{396};
t1522 = ct{397};
t1523 = ct{398};
t1525 = ct{399};
t1526 = ct{400};
t1527 = ct{401};
t1528 = ct{402};
t1529 = ct{403};
t153 = ct{404};
t1530 = ct{405};
t1531 = ct{406};
t1532 = ct{407};
t1533 = ct{408};
t1535 = ct{409};
t1536 = ct{410};
t1537 = ct{411};
t1538 = ct{412};
t1539 = ct{413};
t1541 = ct{414};
t1542 = ct{415};
t1543 = ct{416};
t1544 = ct{417};
t1545 = ct{418};
t1546 = ct{419};
t1547 = ct{420};
t1549 = ct{421};
t1550 = ct{422};
t1551 = ct{423};
t1552 = ct{424};
t1554 = ct{425};
t1555 = ct{426};
t1556 = ct{427};
t1558 = ct{428};
t1559 = ct{429};
t156 = ct{430};
t1560 = ct{431};
t1565 = ct{432};
t1567 = ct{433};
t1568 = ct{434};
t1569 = ct{435};
t1570 = ct{436};
t1571 = ct{437};
t1572 = ct{438};
t1574 = ct{439};
t1575 = ct{440};
t1576 = ct{441};
t1577 = ct{442};
t1578 = ct{443};
t1579 = ct{444};
t158 = ct{445};
t1581 = ct{446};
t1582 = ct{447};
t1583 = ct{448};
t1584 = ct{449};
t1585 = ct{450};
t1586 = ct{451};
t1587 = ct{452};
t1588 = ct{453};
t1591 = ct{454};
t1592 = ct{455};
t1593 = ct{456};
t1594 = ct{457};
t1595 = ct{458};
t1596 = ct{459};
t1599 = ct{460};
t16 = ct{461};
t160 = ct{462};
t1600 = ct{463};
t1601 = ct{464};
t1602 = ct{465};
t1604 = ct{466};
t1605 = ct{467};
t1606 = ct{468};
t1607 = ct{469};
t1608 = ct{470};
t1609 = ct{471};
t161 = ct{472};
t1613 = ct{473};
t1614 = ct{474};
t1615 = ct{475};
t1616 = ct{476};
t1618 = ct{477};
t1619 = ct{478};
t162 = ct{479};
t1620 = ct{480};
t1621 = ct{481};
t1622 = ct{482};
t1624 = ct{483};
t1625 = ct{484};
t1626 = ct{485};
t1627 = ct{486};
t1628 = ct{487};
t1629 = ct{488};
t1631 = ct{489};
t1633 = ct{490};
t1634 = ct{491};
t1635 = ct{492};
t1636 = ct{493};
t1637 = ct{494};
t1639 = ct{495};
t1640 = ct{496};
t1641 = ct{497};
t1642 = ct{498};
t1643 = ct{499};
t1644 = ct{500};
t1645 = ct{501};
t1646 = ct{502};
t1648 = ct{503};
t1649 = ct{504};
t165 = ct{505};
t1650 = ct{506};
t1651 = ct{507};
t1652 = ct{508};
t1653 = ct{509};
t1654 = ct{510};
t1655 = ct{511};
t1656 = ct{512};
t1657 = ct{513};
t1658 = ct{514};
t1659 = ct{515};
t1660 = ct{516};
t1661 = ct{517};
t1662 = ct{518};
t1663 = ct{519};
t1664 = ct{520};
t1665 = ct{521};
t1666 = ct{522};
t1667 = ct{523};
t1668 = ct{524};
t1669 = ct{525};
t167 = ct{526};
t1670 = ct{527};
t1671 = ct{528};
t1672 = ct{529};
t1673 = ct{530};
t1674 = ct{531};
t1675 = ct{532};
t1676 = ct{533};
t1677 = ct{534};
t1678 = ct{535};
t1679 = ct{536};
t168 = ct{537};
t1680 = ct{538};
t1681 = ct{539};
t1682 = ct{540};
t1683 = ct{541};
t1684 = ct{542};
t1685 = ct{543};
t1686 = ct{544};
t1687 = ct{545};
t1690 = ct{546};
t1691 = ct{547};
t1692 = ct{548};
t1693 = ct{549};
t1694 = ct{550};
t1695 = ct{551};
t1696 = ct{552};
t1697 = ct{553};
t1698 = ct{554};
t1699 = ct{555};
t17 = ct{556};
t170 = ct{557};
t1700 = ct{558};
t1701 = ct{559};
t1704 = ct{560};
t1705 = ct{561};
t1706 = ct{562};
t1707 = ct{563};
t1708 = ct{564};
t1710 = ct{565};
t1711 = ct{566};
t1712 = ct{567};
t1716 = ct{568};
t1717 = ct{569};
t172 = ct{570};
t173 = ct{571};
t1738 = ct{572};
t1739 = ct{573};
t174 = ct{574};
t1740 = ct{575};
t1741 = ct{576};
t1742 = ct{577};
t1743 = ct{578};
t1745 = ct{579};
t1749 = ct{580};
t1750 = ct{581};
t1751 = ct{582};
t1752 = ct{583};
t1753 = ct{584};
t1754 = ct{585};
t1756 = ct{586};
t1757 = ct{587};
t1758 = ct{588};
t1759 = ct{589};
t176 = ct{590};
t1760 = ct{591};
t1761 = ct{592};
t1762 = ct{593};
t1764 = ct{594};
t1765 = ct{595};
t1766 = ct{596};
t1768 = ct{597};
t1769 = ct{598};
t177 = ct{599};
t1770 = ct{600};
t1771 = ct{601};
t1772 = ct{602};
t1773 = ct{603};
t1775 = ct{604};
t1776 = ct{605};
t1777 = ct{606};
t1779 = ct{607};
t178 = ct{608};
t1786 = ct{609};
t1793 = ct{610};
t1794 = ct{611};
t1795 = ct{612};
t1796 = ct{613};
t1797 = ct{614};
t1799 = ct{615};
t18 = ct{616};
t180 = ct{617};
t1800 = ct{618};
t1801 = ct{619};
t1802 = ct{620};
t1807 = ct{621};
t1810 = ct{622};
t1813 = ct{623};
t1814 = ct{624};
t1816 = ct{625};
t1817 = ct{626};
t1819 = ct{627};
t182 = ct{628};
t1820 = ct{629};
t1821 = ct{630};
t1822 = ct{631};
t1823 = ct{632};
t1824 = ct{633};
t1825 = ct{634};
t1826 = ct{635};
t1827 = ct{636};
t1828 = ct{637};
t1829 = ct{638};
t1830 = ct{639};
t1831 = ct{640};
t1832 = ct{641};
t1834 = ct{642};
t1835 = ct{643};
t1836 = ct{644};
t1837 = ct{645};
t1840 = ct{646};
t1841 = ct{647};
t1842 = ct{648};
t1843 = ct{649};
t1844 = ct{650};
t1845 = ct{651};
t185 = ct{652};
t1850 = ct{653};
t1851 = ct{654};
t1856 = ct{655};
t1858 = ct{656};
t186 = ct{657};
t1860 = ct{658};
t1861 = ct{659};
t1862 = ct{660};
t1865 = ct{661};
t1866 = ct{662};
t1868 = ct{663};
t1870 = ct{664};
t1871 = ct{665};
t1874 = ct{666};
t1875 = ct{667};
t1876 = ct{668};
t1878 = ct{669};
t1879 = ct{670};
t188 = ct{671};
t1880 = ct{672};
t1881 = ct{673};
t1882 = ct{674};
t1883 = ct{675};
t1884 = ct{676};
t1885 = ct{677};
t1886 = ct{678};
t1887 = ct{679};
t1888 = ct{680};
t1889 = ct{681};
t189 = ct{682};
t1890 = ct{683};
t1891 = ct{684};
t1892 = ct{685};
t1898 = ct{686};
t19 = ct{687};
t1900 = ct{688};
t1901 = ct{689};
t1902 = ct{690};
t1903 = ct{691};
t1904 = ct{692};
t1905 = ct{693};
t1906 = ct{694};
t1909 = ct{695};
t191 = ct{696};
t1910 = ct{697};
t1911 = ct{698};
t1913 = ct{699};
t1914 = ct{700};
t1917 = ct{701};
t1918 = ct{702};
t192 = ct{703};
t1920 = ct{704};
t1921 = ct{705};
t1923 = ct{706};
t1924 = ct{707};
t1925 = ct{708};
t1926 = ct{709};
t1927 = ct{710};
t1929 = ct{711};
t1930 = ct{712};
t1931 = ct{713};
t1932 = ct{714};
t1933 = ct{715};
t1934 = ct{716};
t1935 = ct{717};
t1936 = ct{718};
t1937 = ct{719};
t1938 = ct{720};
t1939 = ct{721};
t1940 = ct{722};
t1941 = ct{723};
t1943 = ct{724};
t1944 = ct{725};
t1945 = ct{726};
t1946 = ct{727};
t1948 = ct{728};
t195 = ct{729};
t1951 = ct{730};
t1952 = ct{731};
t1953 = ct{732};
t1954 = ct{733};
t1955 = ct{734};
t1956 = ct{735};
t1957 = ct{736};
t1958 = ct{737};
t1959 = ct{738};
t196 = ct{739};
t1960 = ct{740};
t1961 = ct{741};
t1962 = ct{742};
t1963 = ct{743};
t1964 = ct{744};
t1966 = ct{745};
t1967 = ct{746};
t1969 = ct{747};
t197 = ct{748};
t1971 = ct{749};
t1972 = ct{750};
t1973 = ct{751};
t1978 = ct{752};
t1979 = ct{753};
t198 = ct{754};
t1980 = ct{755};
t1981 = ct{756};
t1983 = ct{757};
t1984 = ct{758};
t1985 = ct{759};
t1988 = ct{760};
t1990 = ct{761};
t1991 = ct{762};
t1992 = ct{763};
t1993 = ct{764};
t1994 = ct{765};
t1997 = ct{766};
t1998 = ct{767};
t1999 = ct{768};
t2 = ct{769};
t20 = ct{770};
t2001 = ct{771};
t2002 = ct{772};
t2003 = ct{773};
t2004 = ct{774};
t2005 = ct{775};
t2006 = ct{776};
t2007 = ct{777};
t2008 = ct{778};
t2009 = ct{779};
t201 = ct{780};
t2010 = ct{781};
t2013 = ct{782};
t2014 = ct{783};
t2015 = ct{784};
t2016 = ct{785};
t2017 = ct{786};
t202 = ct{787};
t2023 = ct{788};
t2024 = ct{789};
t2027 = ct{790};
t2028 = ct{791};
t2029 = ct{792};
t203 = ct{793};
t2030 = ct{794};
t2031 = ct{795};
t2032 = ct{796};
t2033 = ct{797};
t2034 = ct{798};
t2035 = ct{799};
t2036 = ct{800};
t2037 = ct{801};
t2039 = ct{802};
t204 = ct{803};
t2040 = ct{804};
t2041 = ct{805};
t2042 = ct{806};
t2043 = ct{807};
t2044 = ct{808};
t2045 = ct{809};
t2049 = ct{810};
t205 = ct{811};
t2050 = ct{812};
t2051 = ct{813};
t2052 = ct{814};
t2053 = ct{815};
t2054 = ct{816};
t2056 = ct{817};
t2057 = ct{818};
t2058 = ct{819};
t2059 = ct{820};
t2060 = ct{821};
t2061 = ct{822};
t2062 = ct{823};
t2063 = ct{824};
t2064 = ct{825};
t2065 = ct{826};
t2066 = ct{827};
t2067 = ct{828};
t2068 = ct{829};
t2069 = ct{830};
t207 = ct{831};
t2070 = ct{832};
t2071 = ct{833};
t2072 = ct{834};
t2073 = ct{835};
t2074 = ct{836};
t2075 = ct{837};
t2077 = ct{838};
t2078 = ct{839};
t2079 = ct{840};
t208 = ct{841};
t2081 = ct{842};
t2082 = ct{843};
t2083 = ct{844};
t2084 = ct{845};
t2085 = ct{846};
t2086 = ct{847};
t2087 = ct{848};
t2089 = ct{849};
t209 = ct{850};
t2090 = ct{851};
t2091 = ct{852};
t2093 = ct{853};
t2094 = ct{854};
t2095 = ct{855};
t2098 = ct{856};
t2099 = ct{857};
t21 = ct{858};
t2100 = ct{859};
t2101 = ct{860};
t2102 = ct{861};
t2103 = ct{862};
t2104 = ct{863};
t2105 = ct{864};
t2106 = ct{865};
t2107 = ct{866};
t2108 = ct{867};
t2109 = ct{868};
t211 = ct{869};
t2110 = ct{870};
t2111 = ct{871};
t2112 = ct{872};
t2113 = ct{873};
t2114 = ct{874};
t2115 = ct{875};
t2116 = ct{876};
t2117 = ct{877};
t2118 = ct{878};
t2119 = ct{879};
t212 = ct{880};
t2120 = ct{881};
t2121 = ct{882};
t2122 = ct{883};
t2123 = ct{884};
t2126 = ct{885};
t2127 = ct{886};
t2128 = ct{887};
t2129 = ct{888};
t2130 = ct{889};
t2136 = ct{890};
t2138 = ct{891};
t2139 = ct{892};
t2140 = ct{893};
t2141 = ct{894};
t2145 = ct{895};
t2146 = ct{896};
t2147 = ct{897};
t2148 = ct{898};
t2149 = ct{899};
t2150 = ct{900};
t2151 = ct{901};
t2152 = ct{902};
t2153 = ct{903};
t2154 = ct{904};
t2155 = ct{905};
t2156 = ct{906};
t2157 = ct{907};
t2159 = ct{908};
t216 = ct{909};
t2160 = ct{910};
t2161 = ct{911};
t2162 = ct{912};
t2164 = ct{913};
t2165 = ct{914};
t2166 = ct{915};
t2167 = ct{916};
t2168 = ct{917};
t2169 = ct{918};
t217 = ct{919};
t2174 = ct{920};
t2175 = ct{921};
t2176 = ct{922};
t2177 = ct{923};
t2178 = ct{924};
t2179 = ct{925};
t218 = ct{926};
t2180 = ct{927};
t2181 = ct{928};
t2182 = ct{929};
t2183 = ct{930};
t2184 = ct{931};
t2185 = ct{932};
t2186 = ct{933};
t2187 = ct{934};
t2188 = ct{935};
t2189 = ct{936};
t2190 = ct{937};
t2191 = ct{938};
t2192 = ct{939};
t2193 = ct{940};
t2194 = ct{941};
t2195 = ct{942};
t2196 = ct{943};
t2197 = ct{944};
t2198 = ct{945};
t2199 = ct{946};
t22 = ct{947};
t2200 = ct{948};
t2201 = ct{949};
t2203 = ct{950};
t2204 = ct{951};
t2205 = ct{952};
t2206 = ct{953};
t2207 = ct{954};
t2209 = ct{955};
t221 = ct{956};
t2210 = ct{957};
t2211 = ct{958};
t2212 = ct{959};
t2213 = ct{960};
t2214 = ct{961};
t2215 = ct{962};
t2217 = ct{963};
t2218 = ct{964};
t2219 = ct{965};
t2220 = ct{966};
t2221 = ct{967};
t2222 = ct{968};
t2223 = ct{969};
t2224 = ct{970};
t2225 = ct{971};
t2226 = ct{972};
t2227 = ct{973};
t2228 = ct{974};
t2229 = ct{975};
t223 = ct{976};
t2230 = ct{977};
t2231 = ct{978};
t2232 = ct{979};
t2233 = ct{980};
t2234 = ct{981};
t2235 = ct{982};
t2236 = ct{983};
t2238 = ct{984};
t2239 = ct{985};
t2240 = ct{986};
t2241 = ct{987};
t2244 = ct{988};
t2245 = ct{989};
t2246 = ct{990};
t2247 = ct{991};
t2249 = ct{992};
t225 = ct{993};
t2250 = ct{994};
t2251 = ct{995};
t2252 = ct{996};
t2253 = ct{997};
t2255 = ct{998};
t2256 = ct{999};
t2257 = ct{1000};
t2259 = ct{1001};
t226 = ct{1002};
t2260 = ct{1003};
t2261 = ct{1004};
t2263 = ct{1005};
t227 = ct{1006};
t229 = ct{1007};
t2290 = ct{1008};
t2291 = ct{1009};
t2292 = ct{1010};
t2294 = ct{1011};
t2295 = ct{1012};
t2296 = ct{1013};
t2297 = ct{1014};
t2299 = ct{1015};
t23 = ct{1016};
t230 = ct{1017};
t2300 = ct{1018};
t2302 = ct{1019};
t2303 = ct{1020};
t2304 = ct{1021};
t2305 = ct{1022};
t2306 = ct{1023};
t2308 = ct{1024};
t2309 = ct{1025};
t231 = ct{1026};
t2310 = ct{1027};
t2311 = ct{1028};
t2313 = ct{1029};
t2314 = ct{1030};
t2315 = ct{1031};
t2316 = ct{1032};
t2317 = ct{1033};
t2320 = ct{1034};
t2322 = ct{1035};
t2323 = ct{1036};
t2324 = ct{1037};
t2325 = ct{1038};
t2326 = ct{1039};
t2327 = ct{1040};
t2328 = ct{1041};
t2329 = ct{1042};
t2331 = ct{1043};
t2332 = ct{1044};
t2333 = ct{1045};
t2334 = ct{1046};
t2336 = ct{1047};
t2339 = ct{1048};
t2340 = ct{1049};
t2341 = ct{1050};
t2343 = ct{1051};
t2345 = ct{1052};
t2346 = ct{1053};
t2347 = ct{1054};
t2352 = ct{1055};
t2353 = ct{1056};
t2354 = ct{1057};
t2357 = ct{1058};
t2358 = ct{1059};
t2359 = ct{1060};
t236 = ct{1061};
t2360 = ct{1062};
t2361 = ct{1063};
t2362 = ct{1064};
t2363 = ct{1065};
t2364 = ct{1066};
t2365 = ct{1067};
t2366 = ct{1068};
t2367 = ct{1069};
t237 = ct{1070};
t2370 = ct{1071};
t2374 = ct{1072};
t2375 = ct{1073};
t2377 = ct{1074};
t2378 = ct{1075};
t2379 = ct{1076};
t238 = ct{1077};
t2380 = ct{1078};
t2382 = ct{1079};
t2384 = ct{1080};
t2385 = ct{1081};
t2386 = ct{1082};
t2389 = ct{1083};
t239 = ct{1084};
t2391 = ct{1085};
t2393 = ct{1086};
t2394 = ct{1087};
t2395 = ct{1088};
t2396 = ct{1089};
t2398 = ct{1090};
t24 = ct{1091};
t240 = ct{1092};
t2401 = ct{1093};
t2402 = ct{1094};
t2403 = ct{1095};
t2404 = ct{1096};
t2405 = ct{1097};
t2408 = ct{1098};
t2409 = ct{1099};
t241 = ct{1100};
t2411 = ct{1101};
t2413 = ct{1102};
t2414 = ct{1103};
t2416 = ct{1104};
t2417 = ct{1105};
t2418 = ct{1106};
t242 = ct{1107};
t2422 = ct{1108};
t2425 = ct{1109};
t2426 = ct{1110};
t2427 = ct{1111};
t243 = ct{1112};
t2431 = ct{1113};
t2432 = ct{1114};
t2433 = ct{1115};
t2434 = ct{1116};
t2438 = ct{1117};
t244 = ct{1118};
t2440 = ct{1119};
t2441 = ct{1120};
t2444 = ct{1121};
t2446 = ct{1122};
t2447 = ct{1123};
t2448 = ct{1124};
t2449 = ct{1125};
t2450 = ct{1126};
t2451 = ct{1127};
t2452 = ct{1128};
t2455 = ct{1129};
t2457 = ct{1130};
t2458 = ct{1131};
t2459 = ct{1132};
t2460 = ct{1133};
t2461 = ct{1134};
t2463 = ct{1135};
t2466 = ct{1136};
t2467 = ct{1137};
t2471 = ct{1138};
t2472 = ct{1139};
t2473 = ct{1140};
t2474 = ct{1141};
t2476 = ct{1142};
t2477 = ct{1143};
t2478 = ct{1144};
t2479 = ct{1145};
t2480 = ct{1146};
t2481 = ct{1147};
t2482 = ct{1148};
t2484 = ct{1149};
t2485 = ct{1150};
t2487 = ct{1151};
t2488 = ct{1152};
t2489 = ct{1153};
t2490 = ct{1154};
t2491 = ct{1155};
t2492 = ct{1156};
t2493 = ct{1157};
t2494 = ct{1158};
t2498 = ct{1159};
t2499 = ct{1160};
t25 = ct{1161};
t2504 = ct{1162};
t2505 = ct{1163};
t2508 = ct{1164};
t2509 = ct{1165};
t2510 = ct{1166};
t2511 = ct{1167};
t2512 = ct{1168};
t2514 = ct{1169};
t2515 = ct{1170};
t2516 = ct{1171};
t2520 = ct{1172};
t2524 = ct{1173};
t2525 = ct{1174};
t2529 = ct{1175};
t2530 = ct{1176};
t2532 = ct{1177};
t2541 = ct{1178};
t2542 = ct{1179};
t2548 = ct{1180};
t2549 = ct{1181};
t2550 = ct{1182};
t2552 = ct{1183};
t2555 = ct{1184};
t2556 = ct{1185};
t2557 = ct{1186};
t2558 = ct{1187};
t2559 = ct{1188};
t2560 = ct{1189};
t2564 = ct{1190};
t2565 = ct{1191};
t2566 = ct{1192};
t2569 = ct{1193};
t257 = ct{1194};
t2570 = ct{1195};
t2571 = ct{1196};
t2572 = ct{1197};
t2577 = ct{1198};
t2578 = ct{1199};
t2579 = ct{1200};
t2580 = ct{1201};
t2581 = ct{1202};
t2582 = ct{1203};
t2583 = ct{1204};
t2584 = ct{1205};
t2585 = ct{1206};
t2586 = ct{1207};
t2587 = ct{1208};
t2589 = ct{1209};
t259 = ct{1210};
t2595 = ct{1211};
t2597 = ct{1212};
t2599 = ct{1213};
t26 = ct{1214};
t260 = ct{1215};
t2600 = ct{1216};
t2601 = ct{1217};
t2603 = ct{1218};
t2604 = ct{1219};
t2605 = ct{1220};
t2606 = ct{1221};
t261 = ct{1222};
t2610 = ct{1223};
t2611 = ct{1224};
t2612 = ct{1225};
t2613 = ct{1226};
t2614 = ct{1227};
t2616 = ct{1228};
t2618 = ct{1229};
t2619 = ct{1230};
t262 = ct{1231};
t2620 = ct{1232};
t2621 = ct{1233};
t2622 = ct{1234};
t2623 = ct{1235};
t2624 = ct{1236};
t2626 = ct{1237};
t2627 = ct{1238};
t2628 = ct{1239};
t2629 = ct{1240};
t263 = ct{1241};
t2630 = ct{1242};
t2632 = ct{1243};
t2633 = ct{1244};
t2634 = ct{1245};
t2635 = ct{1246};
t264 = ct{1247};
t2640 = ct{1248};
t2641 = ct{1249};
t2642 = ct{1250};
t2643 = ct{1251};
t2644 = ct{1252};
t2645 = ct{1253};
t2646 = ct{1254};
t2647 = ct{1255};
t2648 = ct{1256};
t2649 = ct{1257};
t2650 = ct{1258};
t2651 = ct{1259};
t2652 = ct{1260};
t2653 = ct{1261};
t2654 = ct{1262};
t2655 = ct{1263};
t2657 = ct{1264};
t2658 = ct{1265};
t2659 = ct{1266};
t2660 = ct{1267};
t2661 = ct{1268};
t2662 = ct{1269};
t2665 = ct{1270};
t2666 = ct{1271};
t2667 = ct{1272};
t2668 = ct{1273};
t267 = ct{1274};
t268 = ct{1275};
t2699 = ct{1276};
t27 = ct{1277};
t270 = ct{1278};
t271 = ct{1279};
t2718 = ct{1280};
t272 = ct{1281};
t2723 = ct{1282};
t2724 = ct{1283};
t2725 = ct{1284};
t2728 = ct{1285};
t2729 = ct{1286};
t273 = ct{1287};
t2730 = ct{1288};
t2731 = ct{1289};
t2734 = ct{1290};
t2735 = ct{1291};
t2736 = ct{1292};
t274 = ct{1293};
t2742 = ct{1294};
t2745 = ct{1295};
t2748 = ct{1296};
t2749 = ct{1297};
t275 = ct{1298};
t2750 = ct{1299};
t2753 = ct{1300};
t2754 = ct{1301};
t2759 = ct{1302};
t276 = ct{1303};
t2762 = ct{1304};
t2769 = ct{1305};
t2773 = ct{1306};
t2774 = ct{1307};
t2775 = ct{1308};
t2777 = ct{1309};
t2778 = ct{1310};
t2779 = ct{1311};
t2781 = ct{1312};
t2785 = ct{1313};
t2786 = ct{1314};
t2787 = ct{1315};
t2788 = ct{1316};
t279 = ct{1317};
t2790 = ct{1318};
t2792 = ct{1319};
t2795 = ct{1320};
t2796 = ct{1321};
t2797 = ct{1322};
t2798 = ct{1323};
t2799 = ct{1324};
t28 = ct{1325};
t280 = ct{1326};
t2802 = ct{1327};
t2803 = ct{1328};
t2805 = ct{1329};
t2807 = ct{1330};
t2808 = ct{1331};
t2811 = ct{1332};
t2812 = ct{1333};
t2814 = ct{1334};
t2823 = ct{1335};
t283 = ct{1336};
t285 = ct{1337};
t2857 = ct{1338};
t2858 = ct{1339};
t2859 = ct{1340};
t286 = ct{1341};
t2865 = ct{1342};
t2867 = ct{1343};
t2868 = ct{1344};
t2883 = ct{1345};
t2884 = ct{1346};
t2886 = ct{1347};
t2890 = ct{1348};
t2893 = ct{1349};
t2894 = ct{1350};
t2895 = ct{1351};
t2898 = ct{1352};
t2900 = ct{1353};
t2901 = ct{1354};
t2903 = ct{1355};
t2905 = ct{1356};
t291 = ct{1357};
t2911 = ct{1358};
t2914 = ct{1359};
t2917 = ct{1360};
t2918 = ct{1361};
t2919 = ct{1362};
t292 = ct{1363};
t2920 = ct{1364};
t2922 = ct{1365};
t2923 = ct{1366};
t2925 = ct{1367};
t2926 = ct{1368};
t293 = ct{1369};
t2930 = ct{1370};
t2931 = ct{1371};
t2933 = ct{1372};
t2935 = ct{1373};
t295 = ct{1374};
t2962 = ct{1375};
t2963 = ct{1376};
t2964 = ct{1377};
t2965 = ct{1378};
t2966 = ct{1379};
t2969 = ct{1380};
t297 = ct{1381};
t2970 = ct{1382};
t3 = ct{1383};
t30 = ct{1384};
t301 = ct{1385};
t303 = ct{1386};
t305 = ct{1387};
t306 = ct{1388};
t308 = ct{1389};
t309 = ct{1390};
t31 = ct{1391};
t310 = ct{1392};
t311 = ct{1393};
t312 = ct{1394};
t313 = ct{1395};
t314 = ct{1396};
t315 = ct{1397};
t316 = ct{1398};
t318 = ct{1399};
t319 = ct{1400};
t32 = ct{1401};
t320 = ct{1402};
t321 = ct{1403};
t322 = ct{1404};
t323 = ct{1405};
t325 = ct{1406};
t326 = ct{1407};
t328 = ct{1408};
t329 = ct{1409};
t33 = ct{1410};
t330 = ct{1411};
t331 = ct{1412};
t332 = ct{1413};
t333 = ct{1414};
t335 = ct{1415};
t336 = ct{1416};
t337 = ct{1417};
t338 = ct{1418};
t339 = ct{1419};
t34 = ct{1420};
t341 = ct{1421};
t343 = ct{1422};
t346 = ct{1423};
t348 = ct{1424};
t35 = ct{1425};
t350 = ct{1426};
t351 = ct{1427};
t352 = ct{1428};
t354 = ct{1429};
t355 = ct{1430};
t356 = ct{1431};
t358 = ct{1432};
t359 = ct{1433};
t36 = ct{1434};
t360 = ct{1435};
t361 = ct{1436};
t362 = ct{1437};
t363 = ct{1438};
t364 = ct{1439};
t365 = ct{1440};
t366 = ct{1441};
t368 = ct{1442};
t369 = ct{1443};
t370 = ct{1444};
t371 = ct{1445};
t372 = ct{1446};
t373 = ct{1447};
t377 = ct{1448};
t378 = ct{1449};
t38 = ct{1450};
t380 = ct{1451};
t381 = ct{1452};
t382 = ct{1453};
t385 = ct{1454};
t386 = ct{1455};
t387 = ct{1456};
t388 = ct{1457};
t389 = ct{1458};
t39 = ct{1459};
t391 = ct{1460};
t392 = ct{1461};
t393 = ct{1462};
t3940 = ct{1463};
t396 = ct{1464};
t3961 = ct{1465};
t4 = ct{1466};
t404 = ct{1467};
t406 = ct{1468};
t408 = ct{1469};
t410 = ct{1470};
t411 = ct{1471};
t412 = ct{1472};
t413 = ct{1473};
t414 = ct{1474};
t419 = ct{1475};
t42 = ct{1476};
t420 = ct{1477};
t421 = ct{1478};
t422 = ct{1479};
t4220 = ct{1480};
t424 = ct{1481};
t425 = ct{1482};
t426 = ct{1483};
t428 = ct{1484};
t4280 = ct{1485};
t429 = ct{1486};
t4295 = ct{1487};
t43 = ct{1488};
t430 = ct{1489};
t432 = ct{1490};
t434 = ct{1491};
t435 = ct{1492};
t437 = ct{1493};
t438 = ct{1494};
t439 = ct{1495};
t444 = ct{1496};
t445 = ct{1497};
t448 = ct{1498};
t451 = ct{1499};
t452 = ct{1500};
t455 = ct{1501};
t456 = ct{1502};
t457 = ct{1503};
t458 = ct{1504};
t459 = ct{1505};
t46 = ct{1506};
t461 = ct{1507};
t463 = ct{1508};
t464 = ct{1509};
t4644 = ct{1510};
t465 = ct{1511};
t466 = ct{1512};
t467 = ct{1513};
t468 = ct{1514};
t469 = ct{1515};
t47 = ct{1516};
t471 = ct{1517};
t473 = ct{1518};
t474 = ct{1519};
t476 = ct{1520};
t478 = ct{1521};
t479 = ct{1522};
t480 = ct{1523};
t483 = ct{1524};
t485 = ct{1525};
t486 = ct{1526};
t488 = ct{1527};
t489 = ct{1528};
t49 = ct{1529};
t490 = ct{1530};
t491 = ct{1531};
t493 = ct{1532};
t494 = ct{1533};
t495 = ct{1534};
t496 = ct{1535};
t497 = ct{1536};
t498 = ct{1537};
t5 = ct{1538};
t50 = ct{1539};
t503 = ct{1540};
t504 = ct{1541};
t506 = ct{1542};
t507 = ct{1543};
t508 = ct{1544};
t509 = ct{1545};
t510 = ct{1546};
t511 = ct{1547};
t512 = ct{1548};
t513 = ct{1549};
t514 = ct{1550};
t516 = ct{1551};
t517 = ct{1552};
t518 = ct{1553};
t521 = ct{1554};
t522 = ct{1555};
t523 = ct{1556};
t524 = ct{1557};
t525 = ct{1558};
t526 = ct{1559};
t527 = ct{1560};
t528 = ct{1561};
t53 = ct{1562};
t530 = ct{1563};
t531 = ct{1564};
t536 = ct{1565};
t538 = ct{1566};
t539 = ct{1567};
t54 = ct{1568};
t540 = ct{1569};
t542 = ct{1570};
t543 = ct{1571};
t544 = ct{1572};
t546 = ct{1573};
t547 = ct{1574};
t550 = ct{1575};
t551 = ct{1576};
t552 = ct{1577};
t553 = ct{1578};
t556 = ct{1579};
t56 = ct{1580};
t562 = ct{1581};
t563 = ct{1582};
t565 = ct{1583};
t568 = ct{1584};
t569 = ct{1585};
t571 = ct{1586};
t572 = ct{1587};
t573 = ct{1588};
t574 = ct{1589};
t575 = ct{1590};
t576 = ct{1591};
t577 = ct{1592};
t578 = ct{1593};
t58 = ct{1594};
t580 = ct{1595};
t582 = ct{1596};
t583 = ct{1597};
t584 = ct{1598};
t585 = ct{1599};
t589 = ct{1600};
t59 = ct{1601};
t590 = ct{1602};
t592 = ct{1603};
t597 = ct{1604};
t6 = ct{1605};
t60 = ct{1606};
t600 = ct{1607};
t601 = ct{1608};
t605 = ct{1609};
t606 = ct{1610};
t607 = ct{1611};
t608 = ct{1612};
t609 = ct{1613};
t610 = ct{1614};
t611 = ct{1615};
t612 = ct{1616};
t614 = ct{1617};
t615 = ct{1618};
t616 = ct{1619};
t618 = ct{1620};
t620 = ct{1621};
t621 = ct{1622};
t622 = ct{1623};
t623 = ct{1624};
t624 = ct{1625};
t625 = ct{1626};
t627 = ct{1627};
t628 = ct{1628};
t629 = ct{1629};
t63 = ct{1630};
t631 = ct{1631};
t634 = ct{1632};
t635 = ct{1633};
t636 = ct{1634};
t638 = ct{1635};
t640 = ct{1636};
t641 = ct{1637};
t642 = ct{1638};
t643 = ct{1639};
t645 = ct{1640};
t646 = ct{1641};
t648 = ct{1642};
t649 = ct{1643};
t650 = ct{1644};
t651 = ct{1645};
t652 = ct{1646};
t654 = ct{1647};
t655 = ct{1648};
t656 = ct{1649};
t657 = ct{1650};
t658 = ct{1651};
t659 = ct{1652};
t660 = ct{1653};
t662 = ct{1654};
t663 = ct{1655};
t664 = ct{1656};
t665 = ct{1657};
t666 = ct{1658};
t667 = ct{1659};
t668 = ct{1660};
t669 = ct{1661};
t67 = ct{1662};
t670 = ct{1663};
t672 = ct{1664};
t673 = ct{1665};
t674 = ct{1666};
t675 = ct{1667};
t676 = ct{1668};
t677 = ct{1669};
t678 = ct{1670};
t679 = ct{1671};
t68 = ct{1672};
t681 = ct{1673};
t682 = ct{1674};
t683 = ct{1675};
t684 = ct{1676};
t685 = ct{1677};
t686 = ct{1678};
t687 = ct{1679};
t689 = ct{1680};
t691 = ct{1681};
t692 = ct{1682};
t693 = ct{1683};
t694 = ct{1684};
t696 = ct{1685};
t698 = ct{1686};
t7 = ct{1687};
t70 = ct{1688};
t701 = ct{1689};
t702 = ct{1690};
t704 = ct{1691};
t705 = ct{1692};
t707 = ct{1693};
t708 = ct{1694};
t71 = ct{1695};
t710 = ct{1696};
t711 = ct{1697};
t712 = ct{1698};
t713 = ct{1699};
t714 = ct{1700};
t715 = ct{1701};
t716 = ct{1702};
t717 = ct{1703};
t718 = ct{1704};
t719 = ct{1705};
t720 = ct{1706};
t721 = ct{1707};
t722 = ct{1708};
t723 = ct{1709};
t724 = ct{1710};
t725 = ct{1711};
t726 = ct{1712};
t728 = ct{1713};
t73 = ct{1714};
t733 = ct{1715};
t735 = ct{1716};
t736 = ct{1717};
t738 = ct{1718};
t739 = ct{1719};
t740 = ct{1720};
t741 = ct{1721};
t742 = ct{1722};
t743 = ct{1723};
t744 = ct{1724};
t745 = ct{1725};
t746 = ct{1726};
t747 = ct{1727};
t749 = ct{1728};
t750 = ct{1729};
t751 = ct{1730};
t755 = ct{1731};
t756 = ct{1732};
t757 = ct{1733};
t758 = ct{1734};
t759 = ct{1735};
t76 = ct{1736};
t762 = ct{1737};
t763 = ct{1738};
t764 = ct{1739};
t765 = ct{1740};
t766 = ct{1741};
t767 = ct{1742};
t768 = ct{1743};
t770 = ct{1744};
t771 = ct{1745};
t772 = ct{1746};
t773 = ct{1747};
t774 = ct{1748};
t775 = ct{1749};
t776 = ct{1750};
t777 = ct{1751};
t778 = ct{1752};
t78 = ct{1753};
t781 = ct{1754};
t782 = ct{1755};
t783 = ct{1756};
t784 = ct{1757};
t785 = ct{1758};
t786 = ct{1759};
t787 = ct{1760};
t789 = ct{1761};
t79 = ct{1762};
t790 = ct{1763};
t791 = ct{1764};
t792 = ct{1765};
t793 = ct{1766};
t794 = ct{1767};
t796 = ct{1768};
t797 = ct{1769};
t798 = ct{1770};
t799 = ct{1771};
t800 = ct{1772};
t801 = ct{1773};
t802 = ct{1774};
t806 = ct{1775};
t807 = ct{1776};
t808 = ct{1777};
t809 = ct{1778};
t812 = ct{1779};
t813 = ct{1780};
t816 = ct{1781};
t817 = ct{1782};
t818 = ct{1783};
t819 = ct{1784};
t820 = ct{1785};
t821 = ct{1786};
t822 = ct{1787};
t823 = ct{1788};
t824 = ct{1789};
t825 = ct{1790};
t826 = ct{1791};
t827 = ct{1792};
t828 = ct{1793};
t829 = ct{1794};
t830 = ct{1795};
t831 = ct{1796};
t832 = ct{1797};
t833 = ct{1798};
t836 = ct{1799};
t837 = ct{1800};
t838 = ct{1801};
t839 = ct{1802};
t841 = ct{1803};
t844 = ct{1804};
t846 = ct{1805};
t850 = ct{1806};
t852 = ct{1807};
t853 = ct{1808};
t855 = ct{1809};
t856 = ct{1810};
t857 = ct{1811};
t858 = ct{1812};
t859 = ct{1813};
t860 = ct{1814};
t861 = ct{1815};
t863 = ct{1816};
t865 = ct{1817};
t866 = ct{1818};
t868 = ct{1819};
t869 = ct{1820};
t870 = ct{1821};
t871 = ct{1822};
t872 = ct{1823};
t874 = ct{1824};
t876 = ct{1825};
t877 = ct{1826};
t878 = ct{1827};
t881 = ct{1828};
t882 = ct{1829};
t883 = ct{1830};
t885 = ct{1831};
t887 = ct{1832};
t889 = ct{1833};
t89 = ct{1834};
t890 = ct{1835};
t891 = ct{1836};
t893 = ct{1837};
t894 = ct{1838};
t895 = ct{1839};
t896 = ct{1840};
t898 = ct{1841};
t90 = ct{1842};
t900 = ct{1843};
t902 = ct{1844};
t903 = ct{1845};
t904 = ct{1846};
t905 = ct{1847};
t906 = ct{1848};
t907 = ct{1849};
t908 = ct{1850};
t91 = ct{1851};
t911 = ct{1852};
t912 = ct{1853};
t914 = ct{1854};
t915 = ct{1855};
t916 = ct{1856};
t917 = ct{1857};
t918 = ct{1858};
t92 = ct{1859};
t921 = ct{1860};
t924 = ct{1861};
t926 = ct{1862};
t927 = ct{1863};
t930 = ct{1864};
t932 = ct{1865};
t933 = ct{1866};
t934 = ct{1867};
t935 = ct{1868};
t936 = ct{1869};
t937 = ct{1870};
t94 = ct{1871};
t940 = ct{1872};
t942 = ct{1873};
t943 = ct{1874};
t944 = ct{1875};
t945 = ct{1876};
t947 = ct{1877};
t948 = ct{1878};
t950 = ct{1879};
t951 = ct{1880};
t956 = ct{1881};
t959 = ct{1882};
t960 = ct{1883};
t961 = ct{1884};
t962 = ct{1885};
t965 = ct{1886};
t966 = ct{1887};
t967 = ct{1888};
t969 = ct{1889};
t97 = ct{1890};
t970 = ct{1891};
t974 = ct{1892};
t976 = ct{1893};
t978 = ct{1894};
t981 = ct{1895};
t983 = ct{1896};
t985 = ct{1897};
t987 = ct{1898};
t989 = ct{1899};
t99 = ct{1900};
t990 = ct{1901};
t992 = ct{1902};
t993 = ct{1903};
t994 = ct{1904};
t995 = ct{1905};
t996 = ct{1906};
t997 = ct{1907};
t998 = ct{1908};
t999 = ct{1909};
t4704 = t144+t153+t170+t180+t368+t386+t392+t408+t424+t425+t434+t459+t839+t841+t853+t863+t1080+t1148+t1167+t1178+t1179+t1180+t1204+t1234;
t4705 = t150+t156+t168+t178+t355+t385+t391+t396+t404+t406+t432+t457+t838+t844+t852+t861+t1112+t1145+t1177+t1185+t1198+t1199+t1203+t1232;
t4974 = t149+t158+t177+t192+t198+t212+t221+t388+t420+t435+t451+t467+t476+t483+t837+t846+t869+t877+t890+t898+t903+t1092+t1192+t1246+t1252+t1267+t1294+t1297;
t4976 = t148+t165+t174+t186+t207+t209+t218+t377+t419+t448+t452+t464+t495+t496+t836+t857+t866+t883+t889+t896+t900+t1137+t1189+t1229+t1247+t1265+t1278+t1280;
t141 = t47+t49;
t300 = t292.^2;
t347 = -t335;
t535 = -t523;
t549 = -t536;
t564 = -t542;
t579 = -t551;
t581 = -t556;
t587 = -t565;
t593 = -t571;
t594 = -t577;
t598 = -t578;
t644 = -t611;
t680 = -t651;
t925 = -t907;
t941 = t188+t268;
t949 = -t944;
t991 = t948.^2;
t1004 = (t140.*t262)./9.007199254740992e+15;
t1005 = (t140.*t264)./9.007199254740992e+15;
t1022 = t999.^2;
t1033 = t33.*t992;
t1034 = t33.*t993;
t1036 = -t1015;
t1037 = t33.*t995;
t1040 = -t1020;
t1043 = -t1024;
t1053 = -t1038;
t1054 = -t1041;
t1060 = -t1046;
t1063 = -t1051;
t1064 = -t1052;
t1068 = -t1059;
t1069 = -t1062;
t1077 = t14.*t15.*t1041;
t1078 = t14.*t20.*t1041;
t1079 = t15.*t19.*t1041;
t1081 = t19.*t20.*t1041;
t1085 = t14.*t15.*t1028;
t1086 = t14.*t20.*t1028;
t1087 = t15.*t19.*t1028;
t1088 = t19.*t20.*t1028;
t1093 = -t1072;
t1097 = -t1073;
t1127 = t14.*t20.*t1059;
t1128 = t15.*t19.*t1059;
t1130 = -t1090;
t1131 = -t1091;
t1133 = -t1094;
t1134 = t19.*t20.*t1059;
t1136 = -t1095;
t1151 = -t1102;
t1152 = -t1106;
t1153 = -t1107;
t1156 = -t1117;
t1160 = -t1122;
t1163 = t14.*t15.*t1059;
t1164 = -t1132;
t1169 = -t1141;
t1172 = -t1146;
t1173 = -t1147;
t1175 = -t1149;
t1200 = -t1186;
t1211 = -t1188;
t1442 = t337+t348;
t1465 = t33.*t1431;
t1466 = t33.*t1432;
t1467 = t33.*t1439;
t1472 = -t1459;
t1476 = -t1468;
t1502 = -t1486;
t1508 = -t1499;
t1534 = -t1525;
t1540 = -t1532;
t1548 = -t1544;
t1553 = -t1547;
t1557 = -t1552;
t1564 = -t1559;
t1580 = t140.*t264.*6.489053738789607e-19;
t1597 = t140.*t264.*7.194245199571015e-21;
t1603 = -t1588;
t1610 = -t1594;
t1630 = t140.*t262.*7.183142969324763e-22;
t1632 = -t1618;
t1647 = -t1620;
t1709 = -t1633;
t1713 = -t1635;
t1714 = -t1636;
t1715 = -t1637;
t1718 = -t1643;
t1719 = -t1650;
t1720 = -t1651;
t1721 = -t1652;
t1722 = -t1653;
t1723 = -t1654;
t1724 = -t1664;
t1725 = -t1665;
t1726 = -t1666;
t1727 = -t1667;
t1728 = -t1668;
t1729 = -t1671;
t1730 = -t1672;
t1731 = -t1673;
t1732 = -t1674;
t1733 = -t1676;
t1734 = -t1678;
t1735 = -t1681;
t1736 = -t1682;
t1737 = -t1683;
t1744 = -t1691;
t1746 = -t1692;
t1747 = -t1693;
t1748 = -t1694;
t1755 = -t1705;
t1763 = -t1716;
t1767 = -t1739;
t1774 = -t1745;
t1778 = -t1749;
t1781 = -t1756;
t1783 = -t1757;
t1784 = -t1758;
t1785 = -t1759;
t1787 = -t1771;
t1788 = -t1772;
t1789 = -t1773;
t1790 = -t1775;
t1791 = -t1776;
t1792 = -t1777;
t1803 = -t1799;
t1804 = t24.*t25.*t1743;
t1805 = t24.*t31.*t1743;
t1806 = t25.*t30.*t1743;
t1808 = t30.*t31.*t1743;
t1809 = t24.*t25.*t1749;
t1811 = t24.*t31.*t1749;
t1812 = t25.*t30.*t1749;
t1815 = t30.*t31.*t1749;
t1818 = -t1802;
t1833 = -t1810;
t1838 = -t1813;
t1839 = -t1814;
t1846 = -t1826;
t1847 = -t1827;
t1848 = -t1828;
t1849 = -t1829;
t1852 = -t1834;
t1853 = -t1835;
t1854 = -t1836;
t1855 = -t1840;
t1857 = -t1842;
t1859 = -t1843;
t1864 = -t1861;
t1867 = -t1862;
t1869 = -t1866;
t1893 = (t26.*t50.*t140.*t202)./8.112963841460668e+31;
t1896 = (t32.*t50.*t140.*t202)./8.112963841460668e+31;
t2125 = t140.*t264.*1.875105520197095e-20;
t2132 = t35.*t2113;
t2133 = t35.*t2114;
t2134 = t36.*t2113;
t2135 = t36.*t2114;
t2137 = t140.*t264.*7.825108561121397e-23;
t2142 = t140.*t262.*2.075672598245148e-23;
t2143 = -t2136;
t2163 = -t2148;
t2170 = t38.*t2115;
t2171 = t38.*t2116;
t2172 = t39.*t2115;
t2173 = t39.*t2116;
t2202 = -t2175;
t2208 = -t2183;
t2216 = -t2185;
t2237 = -t2186;
t2242 = -t2188;
t2243 = -t2189;
t2248 = -t2193;
t2254 = -t2196;
t2258 = -t2197;
t2262 = -t2199;
t2264 = -t2204;
t2265 = -t2205;
t2266 = -t2206;
t2267 = -t2212;
t2268 = -t2213;
t2269 = -t2214;
t2270 = -t2219;
t2271 = -t2220;
t2272 = -t2221;
t2273 = -t2225;
t2274 = -t2226;
t2275 = -t2228;
t2276 = -t2231;
t2277 = -t2235;
t2278 = -t2236;
t2279 = -t2239;
t2280 = -t2240;
t2281 = -t2244;
t2282 = -t2245;
t2283 = -t2246;
t2284 = -t2247;
t2285 = -t2250;
t2286 = -t2251;
t2287 = -t2252;
t2288 = -t2253;
t2289 = -t2255;
t2293 = -t2290;
t2298 = -t2292;
t2301 = -t2295;
t2307 = t237+t1469;
t2312 = -t2304;
t2321 = t513+t872;
t2335 = t18.*t2297;
t2337 = t23.*t2297;
t2338 = t512+t887;
t2342 = t26.*t50.*t140.*t202.*7.204296868834178e-35;
t2344 = t32.*t50.*t140.*t202.*7.204296868834178e-35;
t2368 = t26.*t50.*t140.*t202.*7.987216665362745e-37;
t2371 = t32.*t50.*t140.*t202.*7.987216665362745e-37;
t2388 = t262+t1484;
t2399 = t518+t891;
t2419 = t517+t904;
t2421 = t26.*t50.*t140.*t202.*7.974890713718666e-38;
t2423 = t32.*t50.*t140.*t202.*7.974890713718666e-38;
t2465 = t28.*t2363;
t2468 = t34.*t2363;
t2470 = t22.*t2297.*(3.0./5.0e+2);
t2500 = t140.*t188.*t201.*2.442490654175345e-23;
t2507 = t140.*t189.*t202.*2.442490654175345e-23;
t2534 = -t2530;
t2535 = t33.*t2363.*(3.0./5.0e+2);
t2538 = t38.*t50.*t292.*6.209141233430105e-19i;
t2539 = t39.*t50.*t292.*6.209141233430105e-19i;
t2554 = (t17.*t2297)./1.0e+8;
t2576 = t39.*t50.*t292.*3.200438707086705e-18i;
t2637 = t38.*t50.*t292.*3.200438707086705e-18i;
t2670 = t35.*t236.*t291.*2.79634861451666e-3;
t2671 = t36.*t236.*t291.*2.79634861451666e-3;
t2678 = t35.*t236.*t291.*1.44134945686578e-2;
t2680 = t36.*t236.*t291.*1.44134945686578e-2;
t2706 = t859+t874;
t2722 = t865+t878;
t2732 = t26.*t50.*t140.*t202.*2.081785322124547e-36;
t2733 = t32.*t50.*t140.*t202.*2.081785322124547e-36;
t2743 = t17.*t2297.*1.247162e-2;
t2744 = t32.*t50.*t140.*t202.*8.687615694748404e-39;
t2757 = t26.*t50.*t140.*t202.*8.687615694748404e-39;
t2758 = t22.*t2297.*5.68686e-3;
t2765 = t26.*t50.*t140.*t202.*2.304459510155286e-39;
t2767 = t32.*t50.*t140.*t202.*2.304459510155286e-39;
t2793 = t22.*t2297.*3.131399999999998e-4;
t2801 = t22.*t2297.*5.7e-7;
t2831 = t17.*t2297.*2.4e-7;
t2832 = t27.*t2363.*1.247162e-2;
t2849 = t33.*t2363.*5.68686e-3;
t2850 = t17.*t2297.*4.0e-8;
t2851 = t22.*t2297.*4.0e-8;
t2909 = t33.*t2363.*3.131399999999998e-4;
t2924 = t38.*t50.*t292.*4.512400254276827e-21i;
t2927 = t39.*t50.*t292.*4.512400254276827e-21i;
t2939 = t38.*t50.*t292.*2.325870823794656e-20i;
t2940 = t39.*t50.*t292.*2.325870823794656e-20i;
t2958 = t50.*t140.*t188.*t202.*2.711709361697228e-39;
t2971 = t526+t1871;
t2972 = t997+t1483;
t2973 = t525+t1878;
t2974 = t35.*t50.*t236.*t291.*3.104570616715053e-19i;
t2975 = t36.*t50.*t236.*t291.*3.104570616715053e-19i;
t2976 = t574+t1921;
t2979 = t35.*t50.*t236.*t291.*1.600219353543352e-18i;
t2980 = t36.*t50.*t236.*t291.*1.600219353543352e-18i;
t2981 = t569+t1938;
t2988 = t318+t323+t1403;
t2989 = t315+t320+t325+t361;
t2990 = t1403.*t1535;
t2993 = t201.*t2297.*8.595599785252598e-9;
t3017 = t201.*t2297.*5.329271866856611e-7;
t3018 = t201.*t2297.*2.784974330421842e-6;
t3019 = t201.*t2297.*6.730354631852784e-6;
t3049 = t50.*t202.*t2297.*9.543032792050485e-25;
t3064 = t50.*t202.*t2297.*9.390344267377678e-22;
t3066 = t50.*t202.*t2297.*5.916680331071301e-23;
t3070 = t50.*t202.*t2297.*3.091942624624357e-22;
t3071 = t50.*t202.*t2297.*7.472194676175529e-22;
t3080 = t17.*t50.*t202.*t2297.*9.733893447891495e-23;
t3081 = t22.*t50.*t202.*t2297.*5.439528691468777e-23;
t3084 = t17.*t50.*t202.*t2297.*2.290327870092116e-23;
t3086 = t17.*t50.*t202.*t2297.*3.817213116820194e-24;
t3087 = t22.*t50.*t202.*t2297.*3.817213116820194e-24;
t3129 = (t2297.*t2363)./1.0e+8;
t3153 = t2297.*t2363.*6.2e-7;
t3154 = t576+t1898+t1932;
t3159 = t17.*t2297.*t2363.*1.02e-6;
t3165 = t572+t1917+t1944;
t3171 = t17.*t2297.*t2363.*(-4.0e-8);
t3172 = t22.*t2297.*t2363.*(-4.0e-8);
t3306 = t38.*t947.*t999.*t2718.*4.392651260556773e-1;
t3308 = t39.*t947.*t999.*t2718.*4.392651260556773e-1;
t3312 = t540+t552+t1914+t1920;
t3317 = t1017+t1057+t1480+t1531;
t3371 = t38.*t947.*t999.*t2718.*2.244797987218524e-1;
t3372 = t39.*t947.*t999.*t2718.*2.244797987218524e-1;
t3374 = t38.*t947.*t999.*t2718.*3.775747223193135e-1;
t3375 = t39.*t947.*t999.*t2718.*3.775747223193135e-1;
t3380 = t38.*t947.*t999.*t2718.*1.015213745795343e-2;
t3381 = t39.*t947.*t999.*t2718.*1.015213745795343e-2;
t3457 = t38.*t947.*t999.*t2718.*2.933606309255039e-4;
t3458 = t39.*t947.*t999.*t2718.*2.933606309255039e-4;
t3504 = t1622+t1766+t1960+t2078;
t3514 = t1100+t1118+t2452+t2482;
t3617 = t524+t575+t1885+t1886+t1957;
t3628 = t543+t610+t1892+t1927+t1998;
t3742 = t1001+t1025+t1031+t1042+t1497+t1509;
t3780 = t2314+t2331+t2332+t2333;
t3781 = t2315+t2316+t2334+t2347;
t3808 = t2723+t2728+t2729+t2731;
t3809 = t2724+t2725+t2730+t2734;
t3846 = t1624+t1669+t1740+t1751+t2056+t2077;
t3847 = t592+t600+t601+t608+t1560+t1570+t1571+t1572;
t3848 = t589+t590+t597+t621+t1567+t1568+t1569+t1583;
t3849 = t584+t585+t607+t622+t1560+t1570+t1571+t1572;
t3850 = t583+t605+t606+t609+t1567+t1568+t1569+t1583;
t3999 = t204+t260+t272+t491+t507+t509+t912+t960+t967+t1304+t1460+t1463;
t4066 = t225+t229+t439+t458+t486+t489+t932+t935+t1264+t1272+t1326+t1422;
t4109 = t1110+t1123+t1124+t1150+t2118+t2119+t2121+t2129;
t4112 = t1104+t1105+t1121+t1126+t2117+t2126+t2127+t2128;
t4115 = t1113+t1114+t1162+t1176+t2118+t2119+t2121+t2129;
t4116 = t1108+t1154+t1158+t1159+t2117+t2126+t2127+t2128;
t4270 = t54+t113+t114+t121+t133+t138+t273+t301+t303+t546+t631+t634+t652+t739+t765+t985+t1029+t1032;
t4282 = t63+t78+t79+t94+t106+t127+t267+t270+t285+t297+t531+t550+t553+t568+t582+t620+t921+t924+t956+t976;
t4289 = t162+t176+t197+t227+t421+t426+t485+t497+t871+t895+t918+t934+t1224+t1262+t1325+t1353;
t4293 = t185+t191+t211+t242+t465+t468+t478+t494+t876+t882+t902+t906+t1248+t1253+t1277+t1296;
t4421 = t1292+t1334+t1402+t1443+t1445+t1446+t1479+t1482+t1796+t1800+t1807+t1817;
t4500 = t547+t905+t908+t1055+t1061+t1066+t1070+t1491+t1523+t1528+t1530+t1533+t1541+t1542;
t4620 = t860+t1255+t1281+t1298+t1401+t1413+t1426+t1430+t1695+t1765+t1793+t1794+t1795+t1797;
t4655 = t53+t103+t109+t110+t111+t120+t132+t136+t275+t283+t295+t309+t311+t527+t544+t618+t625+t627+t629+t650+t701+t735+t970+t981+t994+t1009+t1014+3.064357668490995e+34;
t4789 = t161+t172+t196+t226+t373+t412+t414+t422+t437+t438+t469+t490+t870+t885+t917+t933+t1187+t1209+t1251+t1263+t1270+t1271+t1332+t1423;
t4792 = t160+t173+t195+t223+t389+t411+t413+t445+t455+t456+t466+t488+t868+t894+t916+t930+t1174+t1206+t1241+t1245+t1260+t1261+t1330+t1418;
t4985 = t152+t167+t205+t217+t243+t263+t274+t381+t430+t471+t479+t493+t508+t511+t858+t881+t914+t927+t943+t962+t969+t1213+t1268+t1310+t1383+t1437+t1451+t1461;
et1 = t236.*t241.*t4644.*(t208-t225-t439+t444+t463-t489+t915+t1259+t1364-t26.*t27.*t34.*t240.*1.075008113939401e+50-t33.*t34.*t50.*t240.*1.025883768304404e+34i-t27.*t28.*t32.*t50.*t240.*3.315051378778914e+33i);
et2 = -4.788365138921021e-91;
t5240 = et1.*et2;
et3 = t236.*t241.*t4644.*(t208-t225-t439+t444+t463-t489+t915+t1259+t1364-t26.*t27.*t34.*t240.*1.075008113939401e+50-t33.*t34.*t50.*t240.*1.025883768304404e+34i-t27.*t28.*t32.*t50.*t240.*3.315051378778914e+33i);
et4 = 4.788365138921021e-91;
t5243 = et3.*et4;
et5 = t236.*t241.*t4705.*(t208-t225-t439+t444+t463-t489+t915+t1259+t1364-t26.*t27.*t34.*t240.*1.075008113939401e+50-t33.*t34.*t50.*t240.*1.025883768304404e+34i-t27.*t28.*t32.*t50.*t240.*3.315051378778914e+33i);
et6 = -5.316153227542554e-107;
t5317 = et5.*et6;
et7 = t236.*t241.*t4974.*(t208-t225-t439+t444+t463-t489+t915+t1259+t1364-t26.*t27.*t34.*t240.*1.075008113939401e+50-t33.*t34.*t50.*t240.*1.025883768304404e+34i-t27.*t28.*t32.*t50.*t240.*3.315051378778914e+33i);
et8 = -2.595777943136013e-110;
t5381 = et7.*et8;
t1026 = -t1005;
t1598 = -t1580;
t1612 = -t1597;
t1703 = -t1630;
t1912 = -t1896;
t2350 = t17.*t2307;
t2351 = t18.*t2307;
t2355 = t22.*t2307;
t2356 = t23.*t2307;
t2369 = -t2342;
t2373 = t22.*t2335;
t2376 = t22.*t2337;
t2381 = -t2337;
t2387 = t17.*t2321;
t2390 = t22.*t2321;
t2397 = -t2368;
t2400 = -t2371;
t2410 = t18.*t2338;
t2412 = t23.*t2338;
t2496 = t27.*t2388;
t2497 = t28.*t2388;
t2502 = t33.*t2388;
t2503 = t34.*t2388;
t2517 = -t2500;
t2521 = t27.*t2399;
t2522 = t33.*t2399;
t2526 = t33.*t2465;
t2527 = t28.*t2419;
t2528 = t33.*t2468;
t2531 = t34.*t2419;
t2575 = -t2538;
t2638 = -t2576;
t2664 = -t2637;
t2672 = t2132.*5.110348748545983e-1;
t2673 = -t2670;
t2674 = t2134.*5.110348748545983e-1;
t2675 = -t2671;
t2676 = t2133.*8.595599785252598e-1;
t2679 = t2135.*8.595599785252598e-1;
t2681 = t2132.*2.311164e-2;
t2682 = t2134.*2.311164e-2;
t2683 = -t2678;
t2684 = t2133.*1.273194e-2;
t2685 = -t2680;
t2686 = t2132.*4.251385e-2;
t2687 = t2135.*1.273194e-2;
t2688 = t2134.*4.251385e-2;
t2691 = t2170.*5.110348748545983e-1;
t2692 = t2132.*6.562549e-2;
t2694 = t2172.*5.110348748545983e-1;
t2695 = t2134.*6.562549e-2;
t2697 = t38.*t241.*t300.*2.79634861451666e-3;
t2698 = t39.*t241.*t300.*2.79634861451666e-3;
t2701 = t2171.*8.595599785252598e-1;
t2703 = t2173.*8.595599785252598e-1;
t2707 = t2171.*1.273194e-2;
t2708 = t2170.*4.251385e-2;
t2709 = t2173.*1.273194e-2;
t2710 = t2172.*4.251385e-2;
t2711 = t38.*t241.*t300.*1.44134945686578e-2;
t2712 = t39.*t241.*t300.*1.44134945686578e-2;
t2714 = t2170.*6.562549e-2;
t2716 = t2172.*6.562549e-2;
t2737 = t2335.*9.99471e-3;
t2738 = t2337.*9.99471e-3;
t2739 = t2335.*1.838876e-2;
t2740 = t2337.*1.838876e-2;
t2771 = -t2758;
t2791 = -t2767;
t2804 = t2335.*9.3e-7;
t2806 = t2335.*1.02e-6;
t2810 = t2337.*9.3e-7;
t2813 = t2337.*1.02e-6;
t2817 = t2465.*9.99471e-3;
t2818 = t2468.*9.99471e-3;
t2819 = t2465.*1.838876e-2;
t2820 = t2468.*1.838876e-2;
t2825 = -t2801;
t2835 = t2335.*9.0e-8;
t2838 = t2337.*9.0e-8;
t2870 = -t2849;
t2875 = -t2851;
t2937 = -t2924;
t2941 = -t2939;
t2942 = -t2940;
t2943 = t38.*t241.*t300.*2.032204410370765e-5;
t2944 = t39.*t241.*t300.*2.032204410370765e-5;
t2947 = t2170.*6.678441185616e-4;
t2948 = t2172.*6.678441185616e-4;
t2949 = t2171.*9.2527464159e-5;
t2950 = t2173.*9.2527464159e-5;
t2951 = t38.*t241.*t300.*1.047479097535352e-4;
t2952 = t39.*t241.*t300.*1.047479097535352e-4;
t2955 = t2170.*4.769234047515e-4;
t2956 = t2172.*4.769234047515e-4;
t2961 = -t2958;
t2977 = -t2974;
t2978 = -t2975;
t2982 = -t2980;
t2983 = t39.*t50.*t241.*t300.*3.104570616715053e-19i;
t2984 = t38.*t50.*t241.*t300.*3.104570616715053e-19i;
t2986 = t38.*t50.*t241.*t300.*1.600219353543352e-18i;
t2987 = t39.*t50.*t241.*t300.*1.600219353543352e-18i;
t2991 = t1442.*t1536;
t2999 = t35.*t941.*t991.*2.196325630278387e-1;
t3000 = t36.*t941.*t991.*2.196325630278387e-1;
t3004 = t38.*t50.*t241.*t300.*2.256200127138414e-21i;
t3005 = t39.*t50.*t241.*t300.*2.256200127138414e-21i;
t3008 = t39.*t50.*t241.*t300.*1.162935411897328e-20i;
t3010 = t38.*t50.*t241.*t300.*1.162935411897328e-20i;
t3011 = t39.*t947.*t1022.*2.196325630278387e-1;
t3012 = t38.*t947.*t1022.*2.196325630278387e-1;
t3015 = t201.*t2307.*8.458070188688557e-6;
t3022 = t35.*t941.*t991.*1.122398993609262e-1;
t3023 = t36.*t941.*t991.*1.122398993609262e-1;
t3026 = t35.*t941.*t991.*1.887873611596568e-1;
t3027 = t36.*t941.*t991.*1.887873611596568e-1;
t3029 = t35.*t941.*t991.*5.076068728976717e-3;
t3030 = t36.*t941.*t991.*5.076068728976717e-3;
t3036 = t38.*t947.*t1022.*1.122398993609262e-1;
t3037 = t39.*t947.*t1022.*1.122398993609262e-1;
t3042 = t38.*t947.*t1022.*1.887873611596568e-1;
t3043 = t39.*t947.*t1022.*1.887873611596568e-1;
t3044 = t38.*t947.*t1022.*5.076068728976717e-3;
t3045 = t39.*t947.*t1022.*5.076068728976717e-3;
t3050 = t50.*t202.*t2307.*9.543032792050485e-25;
t3051 = t17.*t3049;
t3054 = t410.*t2989;
t3055 = t50.*t202.*t2338.*9.543032792050485e-25;
t3056 = t429.*t2988;
t3065 = t50.*t202.*t2307.*9.390344267377678e-22;
t3067 = t50.*t202.*t2307.*5.916680331071301e-23;
t3068 = t50.*t202.*t2321.*9.390344267377678e-22;
t3069 = t38.*t947.*t1022.*1.46680315462752e-4;
t3072 = t39.*t947.*t1022.*1.46680315462752e-4;
t3074 = t50.*t202.*t2307.*3.091942624624357e-22;
t3075 = -t3070;
t3076 = t50.*t202.*t2307.*7.472194676175529e-22;
t3077 = -t3071;
t3079 = t50.*t202.*t2338.*5.916680331071301e-23;
t3082 = t50.*t202.*t2338.*3.091942624624357e-22;
t3083 = t50.*t202.*t2338.*7.472194676175529e-22;
t3085 = -t3081;
t3088 = -t3084;
t3119 = t1039+t1064+t1520;
t3120 = t1030+t1069+t1518;
tau_c = ft_6({t100,t1000,t1002,t1003,t1004,t1005,t1006,t101,t1011,t1015,t1018,t1019,t1020,t1021,t1022,t1023,t1024,t1026,t1028,t1033,t1034,t1035,t1036,t1037,t1038,t1040,t1043,t1044,t1045,t1046,t1048,t1049,t1050,t1051,t1053,t1054,t1056,t1057,t1058,t1059,t1060,t1063,t1065,t1067,t1068,t107,t1071,t1072,t1074,t1075,t1076,t1077,t1078,t1079,t108,t1083,t1084,t1088,t1089,t1093,t1097,t1098,t1099,t1103,t1104,t1105,t1108,t1109,t1111,t1115,t1116,t1119,t1120,t1121,t1125,t1127,t1128,t1129,t1130,t1131,t1133,t1135,t1136,t1138,t1139,t1140,t1142,t1144,t1151,t1152,t1153,t1156,t1158,t1159,t1160,t1163,t1164,t1165,t1169,t1172,t1173,t1175,t1190,t1193,t1194,t1195,t1196,t1200,t1205,t1207,t1208,t1210,t1211,t1212,t1214,t1217,t1218,t1219,t1220,t1221,t1222,t123,t1230,t1235,t1236,t1237,t1238,t124,t126,t1266,t128,t1285,t1286,t1287,t1288,t1289,t1290,t1299,t130,t1300,t1301,t1302,t1303,t1305,t1307,t1311,t1316,t1317,t1319,t1320,t1322,t1323,t1324,t1328,t1331,t1335,t1336,t1337,t1338,t134,t1342,t1343,t1344,t1345,t1348,t1349,t1350,t1351,t1352,t1354,t1360,t1366,t1367,t1368,t1369,t1370,t1371,t1372,t1374,t1375,t1376,t1377,t1378,t1379,t1380,t1385,t1386,t1387,t1388,t1389,t139,t1392,t1393,t1394,t1395,t1396,t1397,t1398,t1399,t14,t140,t1404,t1405,t1406,t1407,t1408,t1409,t1410,t1411,t1412,t1414,t1415,t1416,t1417,t1419,t1420,t1421,t1424,t1425,t1427,t1428,t1429,t1431,t1432,t1433,t1434,t1435,t1436,t1439,t1440,t1441,t1444,t1447,t1448,t1453,t1456,t1457,t1458,t1462,t1464,t1465,t1466,t1467,t1471,t1472,t1476,t1477,t1478,t1481,t1485,t1487,t1488,t1489,t1490,t1492,t1493,t1494,t1495,t1498,t15,t1500,t1501,t1502,t1503,t1504,t1505,t1506,t1507,t1508,t151,t1510,t1512,t1513,t1514,t1515,t1516,t1517,t1519,t1522,t1526,t1527,t1529,t1531,t1534,t1537,t1538,t1539,t1540,t1543,t1544,t1545,t1546,t1547,t1548,t1549,t1550,t1551,t1553,t1554,t1555,t1556,t1557,t1558,t1559,t1564,t1565,t1574,t1575,t1576,t1577,t1578,t1579,t1581,t1582,t1584,t1585,t1586,t1587,t1591,t1592,t1593,t1595,t1596,t1598,t1599,t16,t1600,t1601,t1602,t1603,t1604,t1605,t1606,t1607,t1608,t1609,t1610,t1612,t1613,t1614,t1615,t1616,t1619,t1621,t1625,t1626,t1627,t1628,t1629,t1631,t1632,t1634,t1637,t1639,t1640,t1641,t1642,t1644,t1645,t1646,t1647,t1648,t1649,t1655,t1656,t1657,t1658,t1659,t1660,t1661,t1662,t1663,t1666,t1667,t1670,t1675,t1677,t1679,t1680,t1683,t1684,t1685,t1686,t1687,t1690,t1692,t1696,t1697,t1698,t1699,t17,t1700,t1701,t1703,t1704,t1705,t1706,t1707,t1708,t1709,t1710,t1711,t1712,t1713,t1714,t1715,t1717,t1718,t1719,t1720,t1721,t1722,t1723,t1724,t1725,t1726,t1727,t1728,t1729,t1730,t1731,t1732,t1733,t1734,t1735,t1736,t1737,t1738,t1739,t1741,t1742,t1743,t1744,t1745,t1746,t1747,t1748,t1750,t1752,t1753,t1754,t1755,t1758,t1759,t1760,t1761,t1762,t1763,t1764,t1767,t1768,t1769,t1770,t1774,t1775,t1776,t1778,t1779,t1781,t1783,t1784,t1785,t1786,t1787,t1788,t1789,t1790,t1791,t1792,t18,t1801,t1803,t1808,t1809,t1811,t1812,t1816,t1818,t1819,t182,t1820,t1821,t1822,t1823,t1824,t1825,t1830,t1831,t1832,t1833,t1837,t1838,t1839,t1841,t1844,t1845,t1846,t1847,t1848,t1849,t1850,t1851,t1852,t1853,t1854,t1855,t1856,t1857,t1858,t1859,t1860,t1861,t1864,t1865,t1867,t1868,t1869,t1870,t1874,t1875,t1876,t1879,t188,t1880,t1881,t1882,t1883,t1884,t1886,t1887,t1888,t1889,t189,t1890,t1891,t1893,t1896,t19,t1900,t1901,t1902,t1903,t1904,t1905,t1906,t1909,t1910,t1911,t1912,t1913,t1918,t1923,t1924,t1925,t1926,t1927,t1929,t1930,t1931,t1933,t1934,t1935,t1936,t1937,t1939,t1940,t1941,t1943,t1945,t1946,t1948,t1951,t1952,t1953,t1954,t1955,t1956,t1957,t1958,t1959,t1961,t1962,t1963,t1964,t1966,t1967,t1969,t1971,t1972,t1973,t1978,t1979,t1980,t1981,t1983,t1984,t1985,t1988,t1990,t1991,t1992,t1993,t1994,t1997,t1998,t1999,t2,t20,t2001,t2002,t2003,t2004,t2005,t2006,t2007,t2008,t2009,t201,t2010,t2013,t2014,t2015,t2016,t2017,t202,t2023,t2024,t2027,t2028,t2029,t203,t2030,t2031,t2032,t2033,t2034,t2035,t2036,t2037,t2039,t2040,t2041,t2042,t2043,t2044,t2045,t2049,t2050,t2051,t2052,t2053,t2054,t2057,t2058,t2059,t2060,t2061,t2062,t2063,t2064,t2065,t2066,t2067,t2068,t2069,t2070,t2071,t2072,t2073,t2074,t2075,t2079,t2081,t2082,t2083,t2084,t2085,t2086,t2087,t2089,t2090,t2091,t2093,t2094,t2095,t2098,t2099,t21,t2100,t2101,t2102,t2103,t2104,t2105,t2106,t2107,t2108,t2109,t2110,t2111,t2112,t2117,t2120,t2122,t2123,t2125,t2130,t2132,t2133,t2134,t2135,t2137,t2138,t2139,t2140,t2141,t2142,t2143,t2145,t2146,t2147,t2149,t2150,t2151,t2152,t2153,t2154,t2155,t2156,t2157,t2159,t216,t2160,t2161,t2162,t2163,t2164,t2165,t2166,t2167,t2168,t2169,t2170,t2171,t2172,t2173,t2174,t2176,t2177,t2178,t2179,t2180,t2181,t2182,t2183,t2184,t2187,t2190,t2191,t2192,t2193,t2194,t2195,t2198,t2199,t22,t2200,t2201,t2202,t2203,t2207,t2208,t2209,t2210,t2211,t2215,t2216,t2217,t2218,t2219,t2222,t2223,t2224,t2227,t2229,t2230,t2232,t2233,t2234,t2237,t2238,t2239,t2240,t2241,t2242,t2243,t2248,t2249,t2254,t2256,t2257,t2258,t2259,t2260,t2261,t2262,t2263,t2264,t2265,t2266,t2267,t2268,t2269,t2270,t2271,t2272,t2273,t2274,t2275,t2276,t2277,t2278,t2279,t2280,t2281,t2282,t2283,t2284,t2285,t2286,t2287,t2288,t2289,t2290,t2291,t2292,t2293,t2294,t2295,t2296,t2297,t2298,t2299,t23,t230,t2300,t2301,t2302,t2303,t2304,t2305,t2306,t2307,t2308,t2309,t231,t2310,t2311,t2312,t2313,t2317,t2320,t2322,t2323,t2324,t2325,t2326,t2327,t2328,t2329,t2335,t2336,t2337,t2338,t2339,t2340,t2341,t2342,t2343,t2344,t2345,t2346,t2350,t2351,t2352,t2353,t2354,t2355,t2356,t2357,t2358,t2359,t236,t2360,t2361,t2362,t2363,t2364,t2365,t2366,t2367,t2368,t2369,t237,t2370,t2371,t2373,t2374,t2375,t2376,t2377,t2378,t2379,t238,t2380,t2381,t2382,t2384,t2385,t2386,t2387,t2388,t2389,t239,t2390,t2391,t2393,t2394,t2395,t2396,t2397,t2398,t2399,t24,t2400,t2401,t2402,t2403,t2404,t2405,t2408,t2409,t241,t2410,t2411,t2412,t2413,t2414,t2416,t2417,t2418,t2419,t2421,t2422,t2423,t2425,t2426,t2427,t2431,t2432,t2433,t2434,t2438,t244,t2440,t2441,t2444,t2446,t2447,t2448,t2449,t2450,t2451,t2455,t2457,t2458,t2459,t2460,t2461,t2463,t2465,t2466,t2467,t2468,t2470,t2471,t2472,t2473,t2474,t2476,t2477,t2478,t2479,t2480,t2481,t2484,t2485,t2487,t2488,t2489,t2490,t2491,t2492,t2493,t2494,t2496,t2497,t2498,t2499,t25,t2500,t2502,t2503,t2504,t2505,t2507,t2508,t2509,t2510,t2511,t2512,t2514,t2515,t2516,t2517,t2520,t2521,t2522,t2524,t2525,t2526,t2527,t2528,t2529,t2530,t2531,t2532,t2534,t2535,t2539,t2541,t2542,t2548,t2549,t2550,t2552,t2554,t2555,t2556,t2557,t2558,t2559,t2560,t2564,t2565,t2566,t2569,t257,t2570,t2571,t2572,t2575,t2577,t2578,t2579,t2580,t2581,t2582,t2583,t2584,t2585,t2586,t2587,t2589,t259,t2595,t2597,t2599,t26,t2600,t2601,t2603,t2604,t2605,t2606,t261,t2610,t2611,t2612,t2613,t2614,t2616,t2618,t2619,t262,t2620,t2621,t2622,t2623,t2624,t2626,t2627,t2628,t2629,t2630,t2632,t2633,t2634,t2635,t2638,t264,t2640,t2641,t2642,t2643,t2644,t2645,t2646,t2647,t2648,t2649,t2650,t2651,t2652,t2653,t2654,t2655,t2657,t2658,t2659,t2660,t2661,t2662,t2664,t2665,t2666,t2667,t2668,t2670,t2671,t2672,t2673,t2674,t2675,t2676,t2678,t2679,t2680,t2681,t2682,t2683,t2684,t2685,t2686,t2687,t2688,t2691,t2692,t2694,t2695,t2697,t2698,t2699,t27,t2701,t2703,t2707,t2708,t2709,t271,t2710,t2711,t2712,t2714,t2716,t2732,t2733,t2735,t2736,t2737,t2738,t2739,t2740,t2742,t2743,t2744,t2745,t2748,t2749,t2750,t2753,t2754,t2757,t2759,t276,t2762,t2765,t2769,t2771,t2773,t2774,t2775,t2777,t2778,t2779,t2781,t2785,t2786,t2787,t2788,t279,t2790,t2791,t2792,t2793,t2795,t2796,t2797,t2798,t2799,t28,t280,t2801,t2802,t2803,t2804,t2805,t2806,t2807,t2808,t2810,t2811,t2812,t2813,t2814,t2817,t2818,t2819,t2820,t2823,t2825,t2831,t2832,t2835,t2838,t2850,t2851,t2857,t2858,t2859,t286,t2865,t2867,t2868,t2870,t2875,t2883,t2884,t2886,t2890,t2893,t2894,t2895,t2898,t2900,t2901,t2903,t2905,t2909,t2911,t2914,t2917,t2918,t2919,t2920,t2922,t2923,t2925,t2926,t2927,t293,t2930,t2931,t2933,t2935,t2937,t2941,t2942,t2943,t2944,t2947,t2948,t2949,t2950,t2951,t2952,t2955,t2956,t2961,t2962,t2963,t2964,t2965,t2966,t2969,t2970,t2971,t2972,t2973,t2975,t2976,t2977,t2978,t2979,t2981,t2982,t2983,t2984,t2986,t2987,t2990,t2991,t2993,t2999,t3,t30,t3000,t3004,t3005,t3008,t3010,t3011,t3012,t3015,t3017,t3018,t3019,t3022,t3023,t3026,t3027,t3029,t3030,t3036,t3037,t3042,t3043,t3044,t3045,t3049,t305,t3050,t3051,t3054,t3055,t3056,t306,t3064,t3065,t3066,t3067,t3068,t3069,t3072,t3074,t3075,t3076,t3077,t3079,t308,t3080,t3081,t3082,t3083,t3085,t3086,t3087,t3088,t31,t310,t3119,t312,t3120,t3129,t313,t314,t3153,t3154,t3159,t316,t3165,t3171,t3172,t319,t32,t321,t322,t326,t328,t329,t33,t330,t3306,t3308,t331,t3312,t3317,t332,t333,t335,t336,t3371,t3372,t3374,t3375,t338,t3380,t3381,t339,t34,t341,t343,t3457,t3458,t346,t347,t35,t350,t3504,t351,t3514,t352,t354,t356,t358,t359,t36,t360,t3617,t362,t3628,t363,t364,t365,t366,t369,t370,t371,t372,t3742,t378,t3780,t3781,t38,t380,t3808,t3809,t382,t3846,t3847,t3848,t3849,t3850,t387,t39,t393,t3940,t3961,t3999,t4,t410,t4109,t4115,t4116,t42,t4220,t4270,t428,t4280,t4282,t4289,t429,t4293,t4295,t43,t4421,t4500,t46,t461,t4620,t4644,t4655,t47,t4704,t4705,t473,t474,t4789,t4792,t480,t4974,t4976,t498,t4985,t5,t50,t503,t504,t506,t510,t514,t516,t521,t522,t523,t524,t5240,t5243,t528,t530,t5317,t535,t538,t5381,t539,t542,t543,t549,t56,t562,t563,t564,t573,t575,t577,t579,t58,t580,t581,t587,t59,t593,t594,t598,t6,t60,t610,t611,t612,t614,t615,t616,t623,t624,t628,t635,t636,t638,t640,t641,t642,t643,t644,t645,t646,t648,t649,t654,t655,t656,t657,t658,t659,t660,t662,t663,t664,t665,t666,t667,t668,t669,t67,t670,t672,t673,t674,t675,t676,t677,t678,t679,t68,t680,t681,t682,t683,t684,t685,t686,t687,t689,t691,t692,t693,t694,t696,t698,t7,t70,t702,t704,t705,t707,t708,t71,t710,t711,t712,t713,t714,t715,t716,t717,t718,t719,t720,t721,t722,t723,t724,t725,t726,t728,t73,t733,t736,t738,t740,t741,t742,t743,t744,t745,t746,t747,t749,t750,t751,t755,t756,t757,t758,t759,t76,t762,t763,t764,t766,t767,t768,t770,t771,t772,t773,t774,t775,t776,t777,t778,t781,t782,t783,t784,t785,t786,t787,t789,t790,t791,t792,t793,t794,t796,t797,t798,t799,t800,t801,t802,t806,t807,t808,t809,t812,t813,t816,t817,t818,t819,t820,t821,t822,t823,t824,t825,t826,t827,t828,t829,t830,t831,t832,t833,t850,t855,t856,t874,t878,t89,t893,t90,t91,t911,t92,t925,t926,t936,t937,t940,t941,t942,t944,t945,t948,t949,t950,t951,t959,t961,t965,t966,t97,t974,t978,t983,t987,t989,t99,t990,t991,t992,t993,t995,t996,t998});
end
function tau_c = ft_6(ct)
t100 = ct{1};
t1000 = ct{2};
t1002 = ct{3};
t1003 = ct{4};
t1004 = ct{5};
t1005 = ct{6};
t1006 = ct{7};
t101 = ct{8};
t1011 = ct{9};
t1015 = ct{10};
t1018 = ct{11};
t1019 = ct{12};
t1020 = ct{13};
t1021 = ct{14};
t1022 = ct{15};
t1023 = ct{16};
t1024 = ct{17};
t1026 = ct{18};
t1028 = ct{19};
t1033 = ct{20};
t1034 = ct{21};
t1035 = ct{22};
t1036 = ct{23};
t1037 = ct{24};
t1038 = ct{25};
t1040 = ct{26};
t1043 = ct{27};
t1044 = ct{28};
t1045 = ct{29};
t1046 = ct{30};
t1048 = ct{31};
t1049 = ct{32};
t1050 = ct{33};
t1051 = ct{34};
t1053 = ct{35};
t1054 = ct{36};
t1056 = ct{37};
t1057 = ct{38};
t1058 = ct{39};
t1059 = ct{40};
t1060 = ct{41};
t1063 = ct{42};
t1065 = ct{43};
t1067 = ct{44};
t1068 = ct{45};
t107 = ct{46};
t1071 = ct{47};
t1072 = ct{48};
t1074 = ct{49};
t1075 = ct{50};
t1076 = ct{51};
t1077 = ct{52};
t1078 = ct{53};
t1079 = ct{54};
t108 = ct{55};
t1083 = ct{56};
t1084 = ct{57};
t1088 = ct{58};
t1089 = ct{59};
t1093 = ct{60};
t1097 = ct{61};
t1098 = ct{62};
t1099 = ct{63};
t1103 = ct{64};
t1104 = ct{65};
t1105 = ct{66};
t1108 = ct{67};
t1109 = ct{68};
t1111 = ct{69};
t1115 = ct{70};
t1116 = ct{71};
t1119 = ct{72};
t1120 = ct{73};
t1121 = ct{74};
t1125 = ct{75};
t1127 = ct{76};
t1128 = ct{77};
t1129 = ct{78};
t1130 = ct{79};
t1131 = ct{80};
t1133 = ct{81};
t1135 = ct{82};
t1136 = ct{83};
t1138 = ct{84};
t1139 = ct{85};
t1140 = ct{86};
t1142 = ct{87};
t1144 = ct{88};
t1151 = ct{89};
t1152 = ct{90};
t1153 = ct{91};
t1156 = ct{92};
t1158 = ct{93};
t1159 = ct{94};
t1160 = ct{95};
t1163 = ct{96};
t1164 = ct{97};
t1165 = ct{98};
t1169 = ct{99};
t1172 = ct{100};
t1173 = ct{101};
t1175 = ct{102};
t1190 = ct{103};
t1193 = ct{104};
t1194 = ct{105};
t1195 = ct{106};
t1196 = ct{107};
t1200 = ct{108};
t1205 = ct{109};
t1207 = ct{110};
t1208 = ct{111};
t1210 = ct{112};
t1211 = ct{113};
t1212 = ct{114};
t1214 = ct{115};
t1217 = ct{116};
t1218 = ct{117};
t1219 = ct{118};
t1220 = ct{119};
t1221 = ct{120};
t1222 = ct{121};
t123 = ct{122};
t1230 = ct{123};
t1235 = ct{124};
t1236 = ct{125};
t1237 = ct{126};
t1238 = ct{127};
t124 = ct{128};
t126 = ct{129};
t1266 = ct{130};
t128 = ct{131};
t1285 = ct{132};
t1286 = ct{133};
t1287 = ct{134};
t1288 = ct{135};
t1289 = ct{136};
t1290 = ct{137};
t1299 = ct{138};
t130 = ct{139};
t1300 = ct{140};
t1301 = ct{141};
t1302 = ct{142};
t1303 = ct{143};
t1305 = ct{144};
t1307 = ct{145};
t1311 = ct{146};
t1316 = ct{147};
t1317 = ct{148};
t1319 = ct{149};
t1320 = ct{150};
t1322 = ct{151};
t1323 = ct{152};
t1324 = ct{153};
t1328 = ct{154};
t1331 = ct{155};
t1335 = ct{156};
t1336 = ct{157};
t1337 = ct{158};
t1338 = ct{159};
t134 = ct{160};
t1342 = ct{161};
t1343 = ct{162};
t1344 = ct{163};
t1345 = ct{164};
t1348 = ct{165};
t1349 = ct{166};
t1350 = ct{167};
t1351 = ct{168};
t1352 = ct{169};
t1354 = ct{170};
t1360 = ct{171};
t1366 = ct{172};
t1367 = ct{173};
t1368 = ct{174};
t1369 = ct{175};
t1370 = ct{176};
t1371 = ct{177};
t1372 = ct{178};
t1374 = ct{179};
t1375 = ct{180};
t1376 = ct{181};
t1377 = ct{182};
t1378 = ct{183};
t1379 = ct{184};
t1380 = ct{185};
t1385 = ct{186};
t1386 = ct{187};
t1387 = ct{188};
t1388 = ct{189};
t1389 = ct{190};
t139 = ct{191};
t1392 = ct{192};
t1393 = ct{193};
t1394 = ct{194};
t1395 = ct{195};
t1396 = ct{196};
t1397 = ct{197};
t1398 = ct{198};
t1399 = ct{199};
t14 = ct{200};
t140 = ct{201};
t1404 = ct{202};
t1405 = ct{203};
t1406 = ct{204};
t1407 = ct{205};
t1408 = ct{206};
t1409 = ct{207};
t1410 = ct{208};
t1411 = ct{209};
t1412 = ct{210};
t1414 = ct{211};
t1415 = ct{212};
t1416 = ct{213};
t1417 = ct{214};
t1419 = ct{215};
t1420 = ct{216};
t1421 = ct{217};
t1424 = ct{218};
t1425 = ct{219};
t1427 = ct{220};
t1428 = ct{221};
t1429 = ct{222};
t1431 = ct{223};
t1432 = ct{224};
t1433 = ct{225};
t1434 = ct{226};
t1435 = ct{227};
t1436 = ct{228};
t1439 = ct{229};
t1440 = ct{230};
t1441 = ct{231};
t1444 = ct{232};
t1447 = ct{233};
t1448 = ct{234};
t1453 = ct{235};
t1456 = ct{236};
t1457 = ct{237};
t1458 = ct{238};
t1462 = ct{239};
t1464 = ct{240};
t1465 = ct{241};
t1466 = ct{242};
t1467 = ct{243};
t1471 = ct{244};
t1472 = ct{245};
t1476 = ct{246};
t1477 = ct{247};
t1478 = ct{248};
t1481 = ct{249};
t1485 = ct{250};
t1487 = ct{251};
t1488 = ct{252};
t1489 = ct{253};
t1490 = ct{254};
t1492 = ct{255};
t1493 = ct{256};
t1494 = ct{257};
t1495 = ct{258};
t1498 = ct{259};
t15 = ct{260};
t1500 = ct{261};
t1501 = ct{262};
t1502 = ct{263};
t1503 = ct{264};
t1504 = ct{265};
t1505 = ct{266};
t1506 = ct{267};
t1507 = ct{268};
t1508 = ct{269};
t151 = ct{270};
t1510 = ct{271};
t1512 = ct{272};
t1513 = ct{273};
t1514 = ct{274};
t1515 = ct{275};
t1516 = ct{276};
t1517 = ct{277};
t1519 = ct{278};
t1522 = ct{279};
t1526 = ct{280};
t1527 = ct{281};
t1529 = ct{282};
t1531 = ct{283};
t1534 = ct{284};
t1537 = ct{285};
t1538 = ct{286};
t1539 = ct{287};
t1540 = ct{288};
t1543 = ct{289};
t1544 = ct{290};
t1545 = ct{291};
t1546 = ct{292};
t1547 = ct{293};
t1548 = ct{294};
t1549 = ct{295};
t1550 = ct{296};
t1551 = ct{297};
t1553 = ct{298};
t1554 = ct{299};
t1555 = ct{300};
t1556 = ct{301};
t1557 = ct{302};
t1558 = ct{303};
t1559 = ct{304};
t1564 = ct{305};
t1565 = ct{306};
t1574 = ct{307};
t1575 = ct{308};
t1576 = ct{309};
t1577 = ct{310};
t1578 = ct{311};
t1579 = ct{312};
t1581 = ct{313};
t1582 = ct{314};
t1584 = ct{315};
t1585 = ct{316};
t1586 = ct{317};
t1587 = ct{318};
t1591 = ct{319};
t1592 = ct{320};
t1593 = ct{321};
t1595 = ct{322};
t1596 = ct{323};
t1598 = ct{324};
t1599 = ct{325};
t16 = ct{326};
t1600 = ct{327};
t1601 = ct{328};
t1602 = ct{329};
t1603 = ct{330};
t1604 = ct{331};
t1605 = ct{332};
t1606 = ct{333};
t1607 = ct{334};
t1608 = ct{335};
t1609 = ct{336};
t1610 = ct{337};
t1612 = ct{338};
t1613 = ct{339};
t1614 = ct{340};
t1615 = ct{341};
t1616 = ct{342};
t1619 = ct{343};
t1621 = ct{344};
t1625 = ct{345};
t1626 = ct{346};
t1627 = ct{347};
t1628 = ct{348};
t1629 = ct{349};
t1631 = ct{350};
t1632 = ct{351};
t1634 = ct{352};
t1637 = ct{353};
t1639 = ct{354};
t1640 = ct{355};
t1641 = ct{356};
t1642 = ct{357};
t1644 = ct{358};
t1645 = ct{359};
t1646 = ct{360};
t1647 = ct{361};
t1648 = ct{362};
t1649 = ct{363};
t1655 = ct{364};
t1656 = ct{365};
t1657 = ct{366};
t1658 = ct{367};
t1659 = ct{368};
t1660 = ct{369};
t1661 = ct{370};
t1662 = ct{371};
t1663 = ct{372};
t1666 = ct{373};
t1667 = ct{374};
t1670 = ct{375};
t1675 = ct{376};
t1677 = ct{377};
t1679 = ct{378};
t1680 = ct{379};
t1683 = ct{380};
t1684 = ct{381};
t1685 = ct{382};
t1686 = ct{383};
t1687 = ct{384};
t1690 = ct{385};
t1692 = ct{386};
t1696 = ct{387};
t1697 = ct{388};
t1698 = ct{389};
t1699 = ct{390};
t17 = ct{391};
t1700 = ct{392};
t1701 = ct{393};
t1703 = ct{394};
t1704 = ct{395};
t1705 = ct{396};
t1706 = ct{397};
t1707 = ct{398};
t1708 = ct{399};
t1709 = ct{400};
t1710 = ct{401};
t1711 = ct{402};
t1712 = ct{403};
t1713 = ct{404};
t1714 = ct{405};
t1715 = ct{406};
t1717 = ct{407};
t1718 = ct{408};
t1719 = ct{409};
t1720 = ct{410};
t1721 = ct{411};
t1722 = ct{412};
t1723 = ct{413};
t1724 = ct{414};
t1725 = ct{415};
t1726 = ct{416};
t1727 = ct{417};
t1728 = ct{418};
t1729 = ct{419};
t1730 = ct{420};
t1731 = ct{421};
t1732 = ct{422};
t1733 = ct{423};
t1734 = ct{424};
t1735 = ct{425};
t1736 = ct{426};
t1737 = ct{427};
t1738 = ct{428};
t1739 = ct{429};
t1741 = ct{430};
t1742 = ct{431};
t1743 = ct{432};
t1744 = ct{433};
t1745 = ct{434};
t1746 = ct{435};
t1747 = ct{436};
t1748 = ct{437};
t1750 = ct{438};
t1752 = ct{439};
t1753 = ct{440};
t1754 = ct{441};
t1755 = ct{442};
t1758 = ct{443};
t1759 = ct{444};
t1760 = ct{445};
t1761 = ct{446};
t1762 = ct{447};
t1763 = ct{448};
t1764 = ct{449};
t1767 = ct{450};
t1768 = ct{451};
t1769 = ct{452};
t1770 = ct{453};
t1774 = ct{454};
t1775 = ct{455};
t1776 = ct{456};
t1778 = ct{457};
t1779 = ct{458};
t1781 = ct{459};
t1783 = ct{460};
t1784 = ct{461};
t1785 = ct{462};
t1786 = ct{463};
t1787 = ct{464};
t1788 = ct{465};
t1789 = ct{466};
t1790 = ct{467};
t1791 = ct{468};
t1792 = ct{469};
t18 = ct{470};
t1801 = ct{471};
t1803 = ct{472};
t1808 = ct{473};
t1809 = ct{474};
t1811 = ct{475};
t1812 = ct{476};
t1816 = ct{477};
t1818 = ct{478};
t1819 = ct{479};
t182 = ct{480};
t1820 = ct{481};
t1821 = ct{482};
t1822 = ct{483};
t1823 = ct{484};
t1824 = ct{485};
t1825 = ct{486};
t1830 = ct{487};
t1831 = ct{488};
t1832 = ct{489};
t1833 = ct{490};
t1837 = ct{491};
t1838 = ct{492};
t1839 = ct{493};
t1841 = ct{494};
t1844 = ct{495};
t1845 = ct{496};
t1846 = ct{497};
t1847 = ct{498};
t1848 = ct{499};
t1849 = ct{500};
t1850 = ct{501};
t1851 = ct{502};
t1852 = ct{503};
t1853 = ct{504};
t1854 = ct{505};
t1855 = ct{506};
t1856 = ct{507};
t1857 = ct{508};
t1858 = ct{509};
t1859 = ct{510};
t1860 = ct{511};
t1861 = ct{512};
t1864 = ct{513};
t1865 = ct{514};
t1867 = ct{515};
t1868 = ct{516};
t1869 = ct{517};
t1870 = ct{518};
t1874 = ct{519};
t1875 = ct{520};
t1876 = ct{521};
t1879 = ct{522};
t188 = ct{523};
t1880 = ct{524};
t1881 = ct{525};
t1882 = ct{526};
t1883 = ct{527};
t1884 = ct{528};
t1886 = ct{529};
t1887 = ct{530};
t1888 = ct{531};
t1889 = ct{532};
t189 = ct{533};
t1890 = ct{534};
t1891 = ct{535};
t1893 = ct{536};
t1896 = ct{537};
t19 = ct{538};
t1900 = ct{539};
t1901 = ct{540};
t1902 = ct{541};
t1903 = ct{542};
t1904 = ct{543};
t1905 = ct{544};
t1906 = ct{545};
t1909 = ct{546};
t1910 = ct{547};
t1911 = ct{548};
t1912 = ct{549};
t1913 = ct{550};
t1918 = ct{551};
t1923 = ct{552};
t1924 = ct{553};
t1925 = ct{554};
t1926 = ct{555};
t1927 = ct{556};
t1929 = ct{557};
t1930 = ct{558};
t1931 = ct{559};
t1933 = ct{560};
t1934 = ct{561};
t1935 = ct{562};
t1936 = ct{563};
t1937 = ct{564};
t1939 = ct{565};
t1940 = ct{566};
t1941 = ct{567};
t1943 = ct{568};
t1945 = ct{569};
t1946 = ct{570};
t1948 = ct{571};
t1951 = ct{572};
t1952 = ct{573};
t1953 = ct{574};
t1954 = ct{575};
t1955 = ct{576};
t1956 = ct{577};
t1957 = ct{578};
t1958 = ct{579};
t1959 = ct{580};
t1961 = ct{581};
t1962 = ct{582};
t1963 = ct{583};
t1964 = ct{584};
t1966 = ct{585};
t1967 = ct{586};
t1969 = ct{587};
t1971 = ct{588};
t1972 = ct{589};
t1973 = ct{590};
t1978 = ct{591};
t1979 = ct{592};
t1980 = ct{593};
t1981 = ct{594};
t1983 = ct{595};
t1984 = ct{596};
t1985 = ct{597};
t1988 = ct{598};
t1990 = ct{599};
t1991 = ct{600};
t1992 = ct{601};
t1993 = ct{602};
t1994 = ct{603};
t1997 = ct{604};
t1998 = ct{605};
t1999 = ct{606};
t2 = ct{607};
t20 = ct{608};
t2001 = ct{609};
t2002 = ct{610};
t2003 = ct{611};
t2004 = ct{612};
t2005 = ct{613};
t2006 = ct{614};
t2007 = ct{615};
t2008 = ct{616};
t2009 = ct{617};
t201 = ct{618};
t2010 = ct{619};
t2013 = ct{620};
t2014 = ct{621};
t2015 = ct{622};
t2016 = ct{623};
t2017 = ct{624};
t202 = ct{625};
t2023 = ct{626};
t2024 = ct{627};
t2027 = ct{628};
t2028 = ct{629};
t2029 = ct{630};
t203 = ct{631};
t2030 = ct{632};
t2031 = ct{633};
t2032 = ct{634};
t2033 = ct{635};
t2034 = ct{636};
t2035 = ct{637};
t2036 = ct{638};
t2037 = ct{639};
t2039 = ct{640};
t2040 = ct{641};
t2041 = ct{642};
t2042 = ct{643};
t2043 = ct{644};
t2044 = ct{645};
t2045 = ct{646};
t2049 = ct{647};
t2050 = ct{648};
t2051 = ct{649};
t2052 = ct{650};
t2053 = ct{651};
t2054 = ct{652};
t2057 = ct{653};
t2058 = ct{654};
t2059 = ct{655};
t2060 = ct{656};
t2061 = ct{657};
t2062 = ct{658};
t2063 = ct{659};
t2064 = ct{660};
t2065 = ct{661};
t2066 = ct{662};
t2067 = ct{663};
t2068 = ct{664};
t2069 = ct{665};
t2070 = ct{666};
t2071 = ct{667};
t2072 = ct{668};
t2073 = ct{669};
t2074 = ct{670};
t2075 = ct{671};
t2079 = ct{672};
t2081 = ct{673};
t2082 = ct{674};
t2083 = ct{675};
t2084 = ct{676};
t2085 = ct{677};
t2086 = ct{678};
t2087 = ct{679};
t2089 = ct{680};
t2090 = ct{681};
t2091 = ct{682};
t2093 = ct{683};
t2094 = ct{684};
t2095 = ct{685};
t2098 = ct{686};
t2099 = ct{687};
t21 = ct{688};
t2100 = ct{689};
t2101 = ct{690};
t2102 = ct{691};
t2103 = ct{692};
t2104 = ct{693};
t2105 = ct{694};
t2106 = ct{695};
t2107 = ct{696};
t2108 = ct{697};
t2109 = ct{698};
t2110 = ct{699};
t2111 = ct{700};
t2112 = ct{701};
t2117 = ct{702};
t2120 = ct{703};
t2122 = ct{704};
t2123 = ct{705};
t2125 = ct{706};
t2130 = ct{707};
t2132 = ct{708};
t2133 = ct{709};
t2134 = ct{710};
t2135 = ct{711};
t2137 = ct{712};
t2138 = ct{713};
t2139 = ct{714};
t2140 = ct{715};
t2141 = ct{716};
t2142 = ct{717};
t2143 = ct{718};
t2145 = ct{719};
t2146 = ct{720};
t2147 = ct{721};
t2149 = ct{722};
t2150 = ct{723};
t2151 = ct{724};
t2152 = ct{725};
t2153 = ct{726};
t2154 = ct{727};
t2155 = ct{728};
t2156 = ct{729};
t2157 = ct{730};
t2159 = ct{731};
t216 = ct{732};
t2160 = ct{733};
t2161 = ct{734};
t2162 = ct{735};
t2163 = ct{736};
t2164 = ct{737};
t2165 = ct{738};
t2166 = ct{739};
t2167 = ct{740};
t2168 = ct{741};
t2169 = ct{742};
t2170 = ct{743};
t2171 = ct{744};
t2172 = ct{745};
t2173 = ct{746};
t2174 = ct{747};
t2176 = ct{748};
t2177 = ct{749};
t2178 = ct{750};
t2179 = ct{751};
t2180 = ct{752};
t2181 = ct{753};
t2182 = ct{754};
t2183 = ct{755};
t2184 = ct{756};
t2187 = ct{757};
t2190 = ct{758};
t2191 = ct{759};
t2192 = ct{760};
t2193 = ct{761};
t2194 = ct{762};
t2195 = ct{763};
t2198 = ct{764};
t2199 = ct{765};
t22 = ct{766};
t2200 = ct{767};
t2201 = ct{768};
t2202 = ct{769};
t2203 = ct{770};
t2207 = ct{771};
t2208 = ct{772};
t2209 = ct{773};
t2210 = ct{774};
t2211 = ct{775};
t2215 = ct{776};
t2216 = ct{777};
t2217 = ct{778};
t2218 = ct{779};
t2219 = ct{780};
t2222 = ct{781};
t2223 = ct{782};
t2224 = ct{783};
t2227 = ct{784};
t2229 = ct{785};
t2230 = ct{786};
t2232 = ct{787};
t2233 = ct{788};
t2234 = ct{789};
t2237 = ct{790};
t2238 = ct{791};
t2239 = ct{792};
t2240 = ct{793};
t2241 = ct{794};
t2242 = ct{795};
t2243 = ct{796};
t2248 = ct{797};
t2249 = ct{798};
t2254 = ct{799};
t2256 = ct{800};
t2257 = ct{801};
t2258 = ct{802};
t2259 = ct{803};
t2260 = ct{804};
t2261 = ct{805};
t2262 = ct{806};
t2263 = ct{807};
t2264 = ct{808};
t2265 = ct{809};
t2266 = ct{810};
t2267 = ct{811};
t2268 = ct{812};
t2269 = ct{813};
t2270 = ct{814};
t2271 = ct{815};
t2272 = ct{816};
t2273 = ct{817};
t2274 = ct{818};
t2275 = ct{819};
t2276 = ct{820};
t2277 = ct{821};
t2278 = ct{822};
t2279 = ct{823};
t2280 = ct{824};
t2281 = ct{825};
t2282 = ct{826};
t2283 = ct{827};
t2284 = ct{828};
t2285 = ct{829};
t2286 = ct{830};
t2287 = ct{831};
t2288 = ct{832};
t2289 = ct{833};
t2290 = ct{834};
t2291 = ct{835};
t2292 = ct{836};
t2293 = ct{837};
t2294 = ct{838};
t2295 = ct{839};
t2296 = ct{840};
t2297 = ct{841};
t2298 = ct{842};
t2299 = ct{843};
t23 = ct{844};
t230 = ct{845};
t2300 = ct{846};
t2301 = ct{847};
t2302 = ct{848};
t2303 = ct{849};
t2304 = ct{850};
t2305 = ct{851};
t2306 = ct{852};
t2307 = ct{853};
t2308 = ct{854};
t2309 = ct{855};
t231 = ct{856};
t2310 = ct{857};
t2311 = ct{858};
t2312 = ct{859};
t2313 = ct{860};
t2317 = ct{861};
t2320 = ct{862};
t2322 = ct{863};
t2323 = ct{864};
t2324 = ct{865};
t2325 = ct{866};
t2326 = ct{867};
t2327 = ct{868};
t2328 = ct{869};
t2329 = ct{870};
t2335 = ct{871};
t2336 = ct{872};
t2337 = ct{873};
t2338 = ct{874};
t2339 = ct{875};
t2340 = ct{876};
t2341 = ct{877};
t2342 = ct{878};
t2343 = ct{879};
t2344 = ct{880};
t2345 = ct{881};
t2346 = ct{882};
t2350 = ct{883};
t2351 = ct{884};
t2352 = ct{885};
t2353 = ct{886};
t2354 = ct{887};
t2355 = ct{888};
t2356 = ct{889};
t2357 = ct{890};
t2358 = ct{891};
t2359 = ct{892};
t236 = ct{893};
t2360 = ct{894};
t2361 = ct{895};
t2362 = ct{896};
t2363 = ct{897};
t2364 = ct{898};
t2365 = ct{899};
t2366 = ct{900};
t2367 = ct{901};
t2368 = ct{902};
t2369 = ct{903};
t237 = ct{904};
t2370 = ct{905};
t2371 = ct{906};
t2373 = ct{907};
t2374 = ct{908};
t2375 = ct{909};
t2376 = ct{910};
t2377 = ct{911};
t2378 = ct{912};
t2379 = ct{913};
t238 = ct{914};
t2380 = ct{915};
t2381 = ct{916};
t2382 = ct{917};
t2384 = ct{918};
t2385 = ct{919};
t2386 = ct{920};
t2387 = ct{921};
t2388 = ct{922};
t2389 = ct{923};
t239 = ct{924};
t2390 = ct{925};
t2391 = ct{926};
t2393 = ct{927};
t2394 = ct{928};
t2395 = ct{929};
t2396 = ct{930};
t2397 = ct{931};
t2398 = ct{932};
t2399 = ct{933};
t24 = ct{934};
t2400 = ct{935};
t2401 = ct{936};
t2402 = ct{937};
t2403 = ct{938};
t2404 = ct{939};
t2405 = ct{940};
